simulink model "COMPONENT_MDL_Lag_QUAD_and_PEND_with_spin_rotors"  (R2021b)
(part 4 of 10)

    et228 = Lz_pend.^2.*THE_Theta_D.*m_pend.*cos(THE_Psi).^2.*cos(THE_Phi_pend).^2.*cos(THE_Psi_pend).*sin(THE_Psi_pend).*(2.0./3.0)+Lz_pend.^2.*THE_Theta_D.*m_pend.*cos(THE_Psi).^2.*cos(THE_Psi_pend).*cos(THE_Theta_pend).^2.*sin(THE_Psi_pend).*(2.0./3.0)+(Ly_pend.^2.*THE_Theta_D.*m_pend.*cos(THE_Psi).*cos(THE_Phi_pend).*cos(THE_Theta_pend).*sin(THE_Psi))./1.2e+1-(Ly_pend.^2.*THE_Theta_pend_D.*m_pend.*cos(THE_Psi).*cos(THE_Phi_pend).*cos(THE_Psi_pend).*sin(THE_Psi_pend))./6.0-(Lz_pend.^2.*THE_Theta_D.*m_pend.*cos(THE_Psi).*cos(THE_Phi_pend).*cos(THE_Theta_pend).*sin(THE_Psi))./3.0+Lz_pend.^2.*THE_Theta_pend_D.*m_pend.*cos(THE_Psi).*cos(THE_Phi_pend).*cos(THE_Psi_pend).*sin(THE_Psi_pend).*(2.0./3.0)+(Ly_pend.^2.*THE_Theta_D.*m_pend.*cos(THE_Psi).^2.*cos(THE_Phi_pend).*cos(THE_Psi_pend).^2.*sin(THE_Phi_pend).*sin(THE_Theta_pend))./6.0-Lz_pend.^2.*THE_Theta_D.*m_pend.*cos(THE_Psi).^2.*cos(THE_Phi_pend).*cos(THE_Psi_pend).^2.*sin(THE_Phi_pend).*sin(THE_Theta_pend).*(2.0./3.0)+(Ly_pend.^2.*THE_Psi_D.*m_pend.*cos(THE_Psi).*cos(THE_Phi_pend).*cos(THE_Psi_pend).*sin(THE_Phi_pend).*sin(THE_Psi_pend))./3.0-Lz_pend.^2.*THE_Psi_D.*m_pend.*cos(THE_Psi).*cos(THE_Phi_pend).*cos(THE_Psi_pend).*sin(THE_Phi_pend).*sin(THE_Psi_pend).*(4.0./3.0);
    et229 = (Ly_pend.^2.*THE_Theta_D.*m_pend.*cos(THE_Psi).^2.*cos(THE_Phi_pend).^2.*cos(THE_Psi_pend).*cos(THE_Theta_pend).^2.*sin(THE_Psi_pend))./1.2e+1-(Lz_pend.^2.*THE_Theta_D.*m_pend.*cos(THE_Psi).^2.*cos(THE_Phi_pend).^2.*cos(THE_Psi_pend).*cos(THE_Theta_pend).^2.*sin(THE_Psi_pend))./3.0+(Lz_pend.*THE_Theta_D.*Tv_Z_pend.*m_pend.*cos(THE_Psi).*cos(THE_Phi_pend).*cos(THE_Psi_pend).*sin(THE_Psi))./2.0+Lz_pend.*THE_Psi_D.*Tv_Z_pend.*m_pend.*cos(THE_Phi_pend).*sin(THE_Psi).*sin(THE_Psi_pend).*sin(THE_Theta_pend)-(Ly_pend.^2.*THE_Theta_D.*m_pend.*cos(THE_Psi).*cos(THE_Phi_pend).*cos(THE_Psi_pend).^2.*cos(THE_Theta_pend).*sin(THE_Psi))./6.0+Lz_pend.^2.*THE_Theta_D.*m_pend.*cos(THE_Psi).*cos(THE_Phi_pend).*cos(THE_Psi_pend).^2.*cos(THE_Theta_pend).*sin(THE_Psi).*(2.0./3.0)-(Ly_pend.^2.*THE_Psi_D.*m_pend.*cos(THE_Phi_pend).*cos(THE_Psi_pend).*cos(THE_Theta_pend).*sin(THE_Psi).*sin(THE_Psi_pend).*sin(THE_Theta_pend))./6.0+(Ly_pend.^2.*THE_Phi_pend_D.*m_pend.*cos(THE_Psi).*cos(THE_Psi_pend).*cos(THE_Theta_pend).*sin(THE_Phi_pend).*sin(THE_Psi_pend).*sin(THE_Theta_pend))./6.0+Lz_pend.^2.*THE_Psi_D.*m_pend.*cos(THE_Phi_pend).*cos(THE_Psi_pend).*cos(THE_Theta_pend).*sin(THE_Psi).*sin(THE_Psi_pend).*sin(THE_Theta_pend).*(2.0./3.0);
    et230 = Lz_pend.^2.*THE_Phi_pend_D.*m_pend.*cos(THE_Psi).*cos(THE_Psi_pend).*cos(THE_Theta_pend).*sin(THE_Phi_pend).*sin(THE_Psi_pend).*sin(THE_Theta_pend).*(-2.0./3.0)+(Lz_pend.*THE_Theta_D.*Tv_Z_pend.*m_pend.*cos(THE_Psi).*sin(THE_Psi).*sin(THE_Phi_pend).*sin(THE_Psi_pend).*sin(THE_Theta_pend))./2.0-(Ly_pend.^2.*THE_Psi_D.*m_pend.*cos(THE_Psi).*cos(THE_Phi_pend).*cos(THE_Psi_pend).*cos(THE_Theta_pend).^2.*sin(THE_Phi_pend).*sin(THE_Psi_pend))./6.0+Lz_pend.^2.*THE_Psi_D.*m_pend.*cos(THE_Psi).*cos(THE_Phi_pend).*cos(THE_Psi_pend).*cos(THE_Theta_pend).^2.*sin(THE_Phi_pend).*sin(THE_Psi_pend).*(2.0./3.0)-(Ly_pend.^2.*THE_Theta_D.*m_pend.*cos(THE_Psi).*cos(THE_Psi_pend).*cos(THE_Theta_pend).*sin(THE_Psi).*sin(THE_Phi_pend).*sin(THE_Psi_pend).*sin(THE_Theta_pend))./6.0+Lz_pend.^2.*THE_Theta_D.*m_pend.*cos(THE_Psi).*cos(THE_Psi_pend).*cos(THE_Theta_pend).*sin(THE_Psi).*sin(THE_Phi_pend).*sin(THE_Psi_pend).*sin(THE_Theta_pend).*(2.0./3.0);
    et231 = (Lx_pend.^2.*THE_Theta_D.*m_pend.*sin(THE_Theta_pend.*2.0))./2.4e+1-(Ly_pend.^2.*THE_Theta_D.*m_pend.*sin(THE_Theta_pend.*2.0))./2.4e+1-(Lx_pend.^2.*THE_Psi_D.*m_pend.*cos(THE_Phi_pend).*sin(THE_Psi))./6.0-(Ly_pend.^2.*THE_Phi_pend_D.*m_pend.*cos(THE_Psi).*sin(THE_Phi_pend))./6.0-(Ly_pend.^2.*THE_Psi_pend_D.*m_pend.*cos(THE_Theta_pend).*sin(THE_Psi))./6.0-(Lx_pend.^2.*THE_Theta_D.*m_pend.*cos(THE_Psi).*sin(THE_Psi).*sin(THE_Phi_pend))./1.2e+1-(Lx_pend.^2.*THE_Phi_pend_D.*m_pend.*cos(THE_Theta_pend).*sin(THE_Psi).*sin(THE_Theta_pend))./6.0+(Ly_pend.^2.*THE_Theta_D.*m_pend.*cos(THE_Psi).*sin(THE_Psi).*sin(THE_Phi_pend))./1.2e+1+(Ly_pend.^2.*THE_Psi_pend_D.*m_pend.*cos(THE_Psi).*sin(THE_Phi_pend).*sin(THE_Theta_pend))./6.0+(Ly_pend.^2.*THE_Phi_pend_D.*m_pend.*cos(THE_Theta_pend).*sin(THE_Psi).*sin(THE_Theta_pend))./6.0+(Lx_pend.^2.*THE_Psi_D.*m_pend.*cos(THE_Phi_pend).*cos(THE_Theta_pend).^2.*sin(THE_Psi))./6.0-(Lx_pend.^2.*THE_Theta_D.*m_pend.*cos(THE_Psi).^2.*cos(THE_Theta_pend).*sin(THE_Theta_pend))./6.0;
    et232 = Lx_pend.^2.*THE_Phi_pend_D.*m_pend.*cos(THE_Psi).*cos(THE_Theta_pend).^2.*sin(THE_Phi_pend).*(-1.0./6.0)-(Ly_pend.^2.*THE_Psi_D.*m_pend.*cos(THE_Phi_pend).*cos(THE_Theta_pend).^2.*sin(THE_Psi))./6.0+(Ly_pend.^2.*THE_Phi_pend_D.*m_pend.*cos(THE_Psi).*cos(THE_Psi_pend).^2.*sin(THE_Phi_pend))./6.0+(Ly_pend.^2.*THE_Theta_D.*m_pend.*cos(THE_Psi).^2.*cos(THE_Theta_pend).*sin(THE_Theta_pend))./6.0+(Ly_pend.^2.*THE_Phi_pend_D.*m_pend.*cos(THE_Psi).*cos(THE_Theta_pend).^2.*sin(THE_Phi_pend))./6.0+(Ly_pend.^2.*THE_Psi_pend_D.*m_pend.*cos(THE_Psi_pend).^2.*cos(THE_Theta_pend).*sin(THE_Psi))./6.0+(Ly_pend.^2.*THE_Theta_D.*m_pend.*cos(THE_Psi_pend).^2.*cos(THE_Theta_pend).*sin(THE_Theta_pend))./1.2e+1-Lz_pend.^2.*THE_Phi_pend_D.*m_pend.*cos(THE_Psi).*cos(THE_Psi_pend).^2.*sin(THE_Phi_pend).*(2.0./3.0)-Lz_pend.^2.*THE_Psi_pend_D.*m_pend.*cos(THE_Psi_pend).^2.*cos(THE_Theta_pend).*sin(THE_Psi).*(2.0./3.0)-(Lz_pend.^2.*THE_Theta_D.*m_pend.*cos(THE_Psi_pend).^2.*cos(THE_Theta_pend).*sin(THE_Theta_pend))./3.0+(Lx_pend.^2.*THE_Theta_D.*m_pend.*cos(THE_Psi).*cos(THE_Theta_pend).^2.*sin(THE_Psi).*sin(THE_Phi_pend))./6.0;
    et233 = Ly_pend.^2.*THE_Theta_D.*m_pend.*cos(THE_Psi).*cos(THE_Psi_pend).^2.*sin(THE_Psi).*sin(THE_Phi_pend).*(-1.0./1.2e+1)-(Ly_pend.^2.*THE_Theta_D.*m_pend.*cos(THE_Psi).*cos(THE_Theta_pend).^2.*sin(THE_Psi).*sin(THE_Phi_pend))./6.0-(Ly_pend.^2.*THE_Psi_pend_D.*m_pend.*cos(THE_Psi).*cos(THE_Psi_pend).^2.*sin(THE_Phi_pend).*sin(THE_Theta_pend))./6.0-(Ly_pend.^2.*THE_Phi_pend_D.*m_pend.*cos(THE_Psi_pend).^2.*cos(THE_Theta_pend).*sin(THE_Psi).*sin(THE_Theta_pend))./6.0+(Lz_pend.^2.*THE_Theta_D.*m_pend.*cos(THE_Psi).*cos(THE_Psi_pend).^2.*sin(THE_Psi).*sin(THE_Phi_pend))./3.0+Lz_pend.^2.*THE_Psi_pend_D.*m_pend.*cos(THE_Psi).*cos(THE_Psi_pend).^2.*sin(THE_Phi_pend).*sin(THE_Theta_pend).*(2.0./3.0)+Lz_pend.^2.*THE_Phi_pend_D.*m_pend.*cos(THE_Psi_pend).^2.*cos(THE_Theta_pend).*sin(THE_Psi).*sin(THE_Theta_pend).*(2.0./3.0)+(Lz_pend.*THE_Theta_D.*Tv_Z_pend.*m_pend.*cos(THE_Psi).^2.*cos(THE_Psi_pend).*sin(THE_Theta_pend))./2.0+(Lx_pend.^2.*THE_Theta_D.*m_pend.*cos(THE_Psi).^2.*cos(THE_Phi_pend).^2.*cos(THE_Theta_pend).*sin(THE_Theta_pend))./1.2e+1+(Ly_pend.^2.*THE_Psi_D.*m_pend.*cos(THE_Phi_pend).*cos(THE_Psi_pend).^2.*cos(THE_Theta_pend).^2.*sin(THE_Psi))./6.0;
    et234 = Ly_pend.^2.*THE_Theta_D.*m_pend.*cos(THE_Psi).^2.*cos(THE_Phi_pend).^2.*cos(THE_Theta_pend).*sin(THE_Theta_pend).*(-1.0./1.2e+1)-(Ly_pend.^2.*THE_Theta_D.*m_pend.*cos(THE_Psi).^2.*cos(THE_Psi_pend).^2.*cos(THE_Theta_pend).*sin(THE_Theta_pend))./6.0-(Ly_pend.^2.*THE_Phi_pend_D.*m_pend.*cos(THE_Psi).*cos(THE_Psi_pend).^2.*cos(THE_Theta_pend).^2.*sin(THE_Phi_pend))./6.0-Lz_pend.^2.*THE_Psi_D.*m_pend.*cos(THE_Phi_pend).*cos(THE_Psi_pend).^2.*cos(THE_Theta_pend).^2.*sin(THE_Psi).*(2.0./3.0)+Lz_pend.^2.*THE_Theta_D.*m_pend.*cos(THE_Psi).^2.*cos(THE_Psi_pend).^2.*cos(THE_Theta_pend).*sin(THE_Theta_pend).*(2.0./3.0)+Lz_pend.^2.*THE_Phi_pend_D.*m_pend.*cos(THE_Psi).*cos(THE_Psi_pend).^2.*cos(THE_Theta_pend).^2.*sin(THE_Phi_pend).*(2.0./3.0)+(Ly_pend.^2.*THE_Psi_pend_D.*m_pend.*cos(THE_Psi).*cos(THE_Phi_pend).*cos(THE_Psi_pend).*sin(THE_Psi_pend))./6.0-Lz_pend.^2.*THE_Psi_pend_D.*m_pend.*cos(THE_Psi).*cos(THE_Phi_pend).*cos(THE_Psi_pend).*sin(THE_Psi_pend).*(2.0./3.0)+(Ly_pend.^2.*THE_Theta_D.*m_pend.*cos(THE_Psi).*cos(THE_Psi_pend).^2.*cos(THE_Theta_pend).^2.*sin(THE_Psi).*sin(THE_Phi_pend))./6.0;
    et235 = Lz_pend.^2.*THE_Theta_D.*m_pend.*cos(THE_Psi).*cos(THE_Psi_pend).^2.*cos(THE_Theta_pend).^2.*sin(THE_Psi).*sin(THE_Phi_pend).*(-2.0./3.0)-(Lx_pend.^2.*THE_Psi_D.*m_pend.*cos(THE_Psi).*cos(THE_Phi_pend).*cos(THE_Theta_pend).*sin(THE_Phi_pend).*sin(THE_Theta_pend))./6.0+(Ly_pend.^2.*THE_Psi_D.*m_pend.*cos(THE_Psi).*cos(THE_Phi_pend).*cos(THE_Theta_pend).*sin(THE_Phi_pend).*sin(THE_Theta_pend))./6.0-(Ly_pend.^2.*THE_Phi_pend_D.*m_pend.*cos(THE_Psi).*cos(THE_Phi_pend).*cos(THE_Psi_pend).*sin(THE_Psi_pend).*sin(THE_Theta_pend))./6.0+Lz_pend.^2.*THE_Phi_pend_D.*m_pend.*cos(THE_Psi).*cos(THE_Phi_pend).*cos(THE_Psi_pend).*sin(THE_Psi_pend).*sin(THE_Theta_pend).*(2.0./3.0)+(Ly_pend.^2.*THE_Theta_D.*m_pend.*cos(THE_Psi).^2.*cos(THE_Phi_pend).^2.*cos(THE_Psi_pend).^2.*cos(THE_Theta_pend).*sin(THE_Theta_pend))./1.2e+1-(Lz_pend.^2.*THE_Theta_D.*m_pend.*cos(THE_Psi).^2.*cos(THE_Phi_pend).^2.*cos(THE_Psi_pend).^2.*cos(THE_Theta_pend).*sin(THE_Theta_pend))./3.0-Lz_pend.*THE_Psi_D.*Tv_Z_pend.*m_pend.*cos(THE_Phi_pend).*cos(THE_Psi_pend).*cos(THE_Theta_pend).*sin(THE_Psi)+(Ly_pend.^2.*THE_Psi_D.*m_pend.*cos(THE_Psi).*cos(THE_Phi_pend).^2.*cos(THE_Psi_pend).*cos(THE_Theta_pend).*sin(THE_Psi_pend))./6.0;
    et236 = Lz_pend.^2.*THE_Psi_D.*m_pend.*cos(THE_Psi).*cos(THE_Phi_pend).^2.*cos(THE_Psi_pend).*cos(THE_Theta_pend).*sin(THE_Psi_pend).*(-2.0./3.0)+(Ly_pend.^2.*THE_Theta_D.*m_pend.*cos(THE_Psi).*cos(THE_Phi_pend).*cos(THE_Psi_pend).*sin(THE_Psi).*sin(THE_Psi_pend).*sin(THE_Theta_pend))./1.2e+1-(Lz_pend.^2.*THE_Theta_D.*m_pend.*cos(THE_Psi).*cos(THE_Phi_pend).*cos(THE_Psi_pend).*sin(THE_Psi).*sin(THE_Psi_pend).*sin(THE_Theta_pend))./3.0-(Lz_pend.*THE_Theta_D.*Tv_Z_pend.*m_pend.*cos(THE_Psi).*cos(THE_Psi_pend).*cos(THE_Theta_pend).*sin(THE_Psi).*sin(THE_Phi_pend))./2.0-(Ly_pend.^2.*THE_Psi_D.*m_pend.*cos(THE_Psi).*cos(THE_Phi_pend).*cos(THE_Psi_pend).^2.*cos(THE_Theta_pend).*sin(THE_Phi_pend).*sin(THE_Theta_pend))./6.0+(Ly_pend.^2.*THE_Theta_D.*m_pend.*cos(THE_Psi).^2.*cos(THE_Phi_pend).*cos(THE_Psi_pend).*cos(THE_Theta_pend).*sin(THE_Phi_pend).*sin(THE_Psi_pend))./1.2e+1+Lz_pend.^2.*THE_Psi_D.*m_pend.*cos(THE_Psi).*cos(THE_Phi_pend).*cos(THE_Psi_pend).^2.*cos(THE_Theta_pend).*sin(THE_Phi_pend).*sin(THE_Theta_pend).*(2.0./3.0)-(Lz_pend.^2.*THE_Theta_D.*m_pend.*cos(THE_Psi).^2.*cos(THE_Phi_pend).*cos(THE_Psi_pend).*cos(THE_Theta_pend).*sin(THE_Phi_pend).*sin(THE_Psi_pend))./3.0;
    et237 = Ly_pend.^2.*THE_Psi_D.*m_pend.*cos(THE_Psi).*(-1.0./6.0)+(Ly_pend.^2.*THE_Theta_pend_D.*m_pend.*cos(THE_Psi).*sin(THE_Phi_pend))./6.0-(Lx_pend.^2.*THE_Psi_D.*m_pend.*cos(THE_Psi).*cos(THE_Theta_pend).^2)./6.0+(Ly_pend.^2.*THE_Psi_D.*m_pend.*cos(THE_Psi).*cos(THE_Phi_pend).^2)./6.0+(Ly_pend.^2.*THE_Psi_D.*m_pend.*cos(THE_Psi).*cos(THE_Psi_pend).^2)./6.0+(Ly_pend.^2.*THE_Psi_D.*m_pend.*cos(THE_Psi).*cos(THE_Theta_pend).^2)./6.0-Lz_pend.^2.*THE_Psi_D.*m_pend.*cos(THE_Psi).*cos(THE_Phi_pend).^2.*(2.0./3.0)-Lz_pend.^2.*THE_Psi_D.*m_pend.*cos(THE_Psi).*cos(THE_Psi_pend).^2.*(2.0./3.0)+(Lx_pend.^2.*THE_Theta_pend_D.*m_pend.*cos(THE_Theta_pend).*sin(THE_Psi).*sin(THE_Theta_pend))./6.0-(Ly_pend.^2.*THE_Theta_pend_D.*m_pend.*cos(THE_Theta_pend).*sin(THE_Psi).*sin(THE_Theta_pend))./6.0+(Lx_pend.^2.*THE_Theta_pend_D.*m_pend.*cos(THE_Psi).*cos(THE_Theta_pend).^2.*sin(THE_Phi_pend))./6.0+(Ly_pend.^2.*THE_Theta_D.*m_pend.*cos(THE_Psi).^2.*cos(THE_Phi_pend).*sin(THE_Phi_pend))./1.2e+1;
    et238 = Ly_pend.^2.*THE_Theta_pend_D.*m_pend.*cos(THE_Psi).*cos(THE_Psi_pend).^2.*sin(THE_Phi_pend).*(-1.0./6.0)-(Ly_pend.^2.*THE_Theta_pend_D.*m_pend.*cos(THE_Psi).*cos(THE_Theta_pend).^2.*sin(THE_Phi_pend))./6.0-(Lz_pend.^2.*THE_Theta_D.*m_pend.*cos(THE_Psi).^2.*cos(THE_Phi_pend).*sin(THE_Phi_pend))./3.0+Lz_pend.^2.*THE_Theta_pend_D.*m_pend.*cos(THE_Psi).*cos(THE_Psi_pend).^2.*sin(THE_Phi_pend).*(2.0./3.0)+(Lx_pend.^2.*THE_Psi_D.*m_pend.*cos(THE_Psi).*cos(THE_Phi_pend).^2.*cos(THE_Theta_pend).^2)./6.0-(Ly_pend.^2.*THE_Psi_D.*m_pend.*cos(THE_Psi).*cos(THE_Phi_pend).^2.*cos(THE_Psi_pend).^2)./3.0-(Ly_pend.^2.*THE_Psi_D.*m_pend.*cos(THE_Psi).*cos(THE_Phi_pend).^2.*cos(THE_Theta_pend).^2)./6.0-(Ly_pend.^2.*THE_Psi_D.*m_pend.*cos(THE_Psi).*cos(THE_Psi_pend).^2.*cos(THE_Theta_pend).^2)./6.0+Lz_pend.^2.*THE_Psi_D.*m_pend.*cos(THE_Psi).*cos(THE_Phi_pend).^2.*cos(THE_Psi_pend).^2.*(4.0./3.0)+Lz_pend.^2.*THE_Psi_D.*m_pend.*cos(THE_Psi).*cos(THE_Psi_pend).^2.*cos(THE_Theta_pend).^2.*(2.0./3.0);
    et239 = Lz_pend.^2.*THE_Psi_pend_D.*m_pend.*cos(THE_Psi).*cos(THE_Phi_pend).*cos(THE_Theta_pend).*(-2.0./3.0)-Lz_pend.*THE_Psi_D.*Tv_Z_pend.*m_pend.*cos(THE_Phi_pend).*sin(THE_Psi).*sin(THE_Psi_pend)-(Ly_pend.^2.*THE_Psi_pend_D.*m_pend.*cos(THE_Psi).*cos(THE_Phi_pend).*cos(THE_Psi_pend).^2.*cos(THE_Theta_pend))./6.0+Lz_pend.^2.*THE_Psi_pend_D.*m_pend.*cos(THE_Psi).*cos(THE_Phi_pend).*cos(THE_Psi_pend).^2.*cos(THE_Theta_pend).*(2.0./3.0)-(Ly_pend.^2.*THE_Theta_D.*m_pend.*cos(THE_Psi).^2.*cos(THE_Psi_pend).*sin(THE_Psi_pend).*sin(THE_Theta_pend))./1.2e+1+(Ly_pend.^2.*THE_Psi_pend_D.*m_pend.*cos(THE_Psi_pend).*cos(THE_Theta_pend).^2.*sin(THE_Psi).*sin(THE_Psi_pend))./6.0+(Ly_pend.^2.*THE_Theta_pend_D.*m_pend.*cos(THE_Psi_pend).^2.*cos(THE_Theta_pend).*sin(THE_Psi).*sin(THE_Theta_pend))./6.0+(Lz_pend.^2.*THE_Theta_D.*m_pend.*cos(THE_Psi).^2.*cos(THE_Psi_pend).*sin(THE_Psi_pend).*sin(THE_Theta_pend))./3.0-Lz_pend.^2.*THE_Psi_pend_D.*m_pend.*cos(THE_Psi_pend).*cos(THE_Theta_pend).^2.*sin(THE_Psi).*sin(THE_Psi_pend).*(2.0./3.0)-Lz_pend.^2.*THE_Theta_pend_D.*m_pend.*cos(THE_Psi_pend).^2.*cos(THE_Theta_pend).*sin(THE_Psi).*sin(THE_Theta_pend).*(2.0./3.0);
    et240 = (Lx_pend.^2.*THE_Theta_D.*m_pend.*cos(THE_Psi).^2.*cos(THE_Phi_pend).*cos(THE_Theta_pend).^2.*sin(THE_Phi_pend))./1.2e+1-(Ly_pend.^2.*THE_Theta_D.*m_pend.*cos(THE_Psi).^2.*cos(THE_Phi_pend).*cos(THE_Psi_pend).^2.*sin(THE_Phi_pend))./6.0-(Ly_pend.^2.*THE_Theta_D.*m_pend.*cos(THE_Psi).^2.*cos(THE_Phi_pend).*cos(THE_Theta_pend).^2.*sin(THE_Phi_pend))./1.2e+1+(Ly_pend.^2.*THE_Theta_pend_D.*m_pend.*cos(THE_Psi).*cos(THE_Psi_pend).^2.*cos(THE_Theta_pend).^2.*sin(THE_Phi_pend))./6.0+Lz_pend.^2.*THE_Theta_D.*m_pend.*cos(THE_Psi).^2.*cos(THE_Phi_pend).*cos(THE_Psi_pend).^2.*sin(THE_Phi_pend).*(2.0./3.0)-Lz_pend.^2.*THE_Theta_pend_D.*m_pend.*cos(THE_Psi).*cos(THE_Psi_pend).^2.*cos(THE_Theta_pend).^2.*sin(THE_Phi_pend).*(2.0./3.0)+(Ly_pend.^2.*THE_Psi_D.*m_pend.*cos(THE_Psi).*cos(THE_Phi_pend).^2.*cos(THE_Psi_pend).^2.*cos(THE_Theta_pend).^2)./6.0-Lz_pend.^2.*THE_Psi_D.*m_pend.*cos(THE_Psi).*cos(THE_Phi_pend).^2.*cos(THE_Psi_pend).^2.*cos(THE_Theta_pend).^2.*(2.0./3.0)-(Lx_pend.^2.*THE_Psi_D.*m_pend.*cos(THE_Theta_pend).*sin(THE_Psi).*sin(THE_Phi_pend).*sin(THE_Theta_pend))./6.0;
    et241 = (Ly_pend.^2.*THE_Psi_D.*m_pend.*cos(THE_Theta_pend).*sin(THE_Psi).*sin(THE_Phi_pend).*sin(THE_Theta_pend))./6.0+(Ly_pend.^2.*THE_Theta_D.*m_pend.*cos(THE_Psi).^2.*cos(THE_Phi_pend).^2.*cos(THE_Psi_pend).*sin(THE_Psi_pend).*sin(THE_Theta_pend))./6.0-Lz_pend.^2.*THE_Theta_D.*m_pend.*cos(THE_Psi).^2.*cos(THE_Phi_pend).^2.*cos(THE_Psi_pend).*sin(THE_Psi_pend).*sin(THE_Theta_pend).*(2.0./3.0)+(Lx_pend.^2.*THE_Theta_D.*m_pend.*cos(THE_Psi).*cos(THE_Phi_pend).*cos(THE_Theta_pend).*sin(THE_Psi).*sin(THE_Theta_pend))./1.2e+1-(Ly_pend.^2.*THE_Theta_D.*m_pend.*cos(THE_Psi).*cos(THE_Phi_pend).*cos(THE_Theta_pend).*sin(THE_Psi).*sin(THE_Theta_pend))./1.2e+1+(Ly_pend.^2.*THE_Psi_D.*m_pend.*cos(THE_Phi_pend).*cos(THE_Psi_pend).*cos(THE_Theta_pend).*sin(THE_Psi).*sin(THE_Psi_pend))./6.0+(Ly_pend.^2.*THE_Theta_pend_D.*m_pend.*cos(THE_Psi).*cos(THE_Phi_pend).*cos(THE_Psi_pend).*sin(THE_Psi_pend).*sin(THE_Theta_pend))./6.0-Lz_pend.^2.*THE_Psi_D.*m_pend.*cos(THE_Phi_pend).*cos(THE_Psi_pend).*cos(THE_Theta_pend).*sin(THE_Psi).*sin(THE_Psi_pend).*(2.0./3.0)-Lz_pend.^2.*THE_Theta_pend_D.*m_pend.*cos(THE_Psi).*cos(THE_Phi_pend).*cos(THE_Psi_pend).*sin(THE_Psi_pend).*sin(THE_Theta_pend).*(2.0./3.0);
    et242 = (Ly_pend.^2.*THE_Theta_D.*m_pend.*cos(THE_Psi).^2.*cos(THE_Phi_pend).*cos(THE_Psi_pend).^2.*cos(THE_Theta_pend).^2.*sin(THE_Phi_pend))./1.2e+1-(Lz_pend.^2.*THE_Theta_D.*m_pend.*cos(THE_Psi).^2.*cos(THE_Phi_pend).*cos(THE_Psi_pend).^2.*cos(THE_Theta_pend).^2.*sin(THE_Phi_pend))./3.0-(Lz_pend.*THE_Theta_D.*Tv_Z_pend.*m_pend.*cos(THE_Psi).*sin(THE_Psi).*sin(THE_Phi_pend).*sin(THE_Psi_pend))./2.0+Lz_pend.*THE_Psi_D.*Tv_Z_pend.*m_pend.*cos(THE_Psi_pend).*sin(THE_Psi).*sin(THE_Phi_pend).*sin(THE_Theta_pend)-(Ly_pend.^2.*THE_Psi_D.*m_pend.*cos(THE_Psi_pend).^2.*cos(THE_Theta_pend).*sin(THE_Psi).*sin(THE_Phi_pend).*sin(THE_Theta_pend))./6.0+Lz_pend.^2.*THE_Psi_D.*m_pend.*cos(THE_Psi_pend).^2.*cos(THE_Theta_pend).*sin(THE_Psi).*sin(THE_Phi_pend).*sin(THE_Theta_pend).*(2.0./3.0)+(Ly_pend.^2.*THE_Theta_D.*m_pend.*cos(THE_Psi).*cos(THE_Psi_pend).*cos(THE_Theta_pend).*sin(THE_Psi).*sin(THE_Phi_pend).*sin(THE_Psi_pend))./1.2e+1-(Ly_pend.^2.*THE_Psi_D.*m_pend.*cos(THE_Psi).*cos(THE_Phi_pend).*cos(THE_Psi_pend).*sin(THE_Phi_pend).*sin(THE_Psi_pend).*sin(THE_Theta_pend))./3.0-(Ly_pend.^2.*THE_Psi_pend_D.*m_pend.*cos(THE_Psi).*cos(THE_Psi_pend).*cos(THE_Theta_pend).*sin(THE_Phi_pend).*sin(THE_Psi_pend).*sin(THE_Theta_pend))./6.0;
    et243 = Lz_pend.^2.*THE_Theta_D.*m_pend.*cos(THE_Psi).*cos(THE_Psi_pend).*cos(THE_Theta_pend).*sin(THE_Psi).*sin(THE_Phi_pend).*sin(THE_Psi_pend).*(-1.0./3.0)+Lz_pend.^2.*THE_Psi_D.*m_pend.*cos(THE_Psi).*cos(THE_Phi_pend).*cos(THE_Psi_pend).*sin(THE_Phi_pend).*sin(THE_Psi_pend).*sin(THE_Theta_pend).*(4.0./3.0)+Lz_pend.^2.*THE_Psi_pend_D.*m_pend.*cos(THE_Psi).*cos(THE_Psi_pend).*cos(THE_Theta_pend).*sin(THE_Phi_pend).*sin(THE_Psi_pend).*sin(THE_Theta_pend).*(2.0./3.0)-(Lz_pend.*THE_Theta_D.*Tv_Z_pend.*m_pend.*cos(THE_Psi).*cos(THE_Phi_pend).*cos(THE_Psi_pend).*sin(THE_Psi).*sin(THE_Theta_pend))./2.0+(Ly_pend.^2.*THE_Theta_D.*m_pend.*cos(THE_Psi).*cos(THE_Phi_pend).*cos(THE_Psi_pend).^2.*cos(THE_Theta_pend).*sin(THE_Psi).*sin(THE_Theta_pend))./1.2e+1-(Lz_pend.^2.*THE_Theta_D.*m_pend.*cos(THE_Psi).*cos(THE_Phi_pend).*cos(THE_Psi_pend).^2.*cos(THE_Theta_pend).*sin(THE_Psi).*sin(THE_Theta_pend))./3.0;
    et244 = THE_Psi_D.*Tv_Z_pend.*m_pend.*sin(THE_Psi).*sin(THE_Theta).*2.0+THE_Psi_D.*cg_to_mot_H.*mprop.*sin(THE_Psi).*sin(THE_Theta).*8.0-THE_Theta_D.*Tv_Z_pend.*m_pend.*cos(THE_Psi).*cos(THE_Theta)-THE_Theta_D.*cg_to_mot_H.*mprop.*cos(THE_Psi).*cos(THE_Theta).*4.0-Lz_pend.*THE_Phi_pend_D.*m_pend.*cos(THE_Theta).*cos(THE_Phi_pend).*sin(THE_Psi_pend)-Lz_pend.*THE_Psi_pend_D.*m_pend.*cos(THE_Theta).*cos(THE_Psi_pend).*sin(THE_Phi_pend)+(Lz_pend.*THE_Theta_D.*m_pend.*sin(THE_Theta).*sin(THE_Phi_pend).*sin(THE_Psi_pend))./2.0-(Lz_pend.*THE_Theta_D.*m_pend.*cos(THE_Psi).*cos(THE_Theta).*cos(THE_Psi_pend).*cos(THE_Theta_pend))./2.0-Lz_pend.*THE_Theta_pend_D.*m_pend.*cos(THE_Theta).*cos(THE_Phi_pend).*cos(THE_Psi_pend).*cos(THE_Theta_pend)+Lz_pend.*THE_Psi_D.*m_pend.*cos(THE_Psi).*cos(THE_Phi_pend).*sin(THE_Theta).*sin(THE_Psi_pend)+(Lz_pend.*THE_Theta_D.*m_pend.*cos(THE_Theta).*cos(THE_Phi_pend).*sin(THE_Psi).*sin(THE_Psi_pend))./2.0+Lz_pend.*THE_Psi_D.*m_pend.*cos(THE_Psi_pend).*cos(THE_Theta_pend).*sin(THE_Psi).*sin(THE_Theta)+Lz_pend.*THE_Psi_pend_D.*m_pend.*cos(THE_Phi_pend).*cos(THE_Psi_pend).*sin(THE_Psi).*sin(THE_Theta)+Lz_pend.*THE_Psi_pend_D.*m_pend.*cos(THE_Psi).*cos(THE_Theta_pend).*sin(THE_Theta).*sin(THE_Psi_pend)+(Lz_pend.*THE_Theta_D.*m_pend.*cos(THE_Phi_pend).*cos(THE_Psi_pend).*sin(THE_Theta).*sin(THE_Theta_pend))./2.0+Lz_pend.*THE_Theta_pend_D.*m_pend.*cos(THE_Psi).*cos(THE_Psi_pend).*sin(THE_Theta).*sin(THE_Theta_pend);
    et245 = Lz_pend.*THE_Phi_pend_D.*m_pend.*cos(THE_Theta).*cos(THE_Psi_pend).*sin(THE_Phi_pend).*sin(THE_Theta_pend)+Lz_pend.*THE_Psi_pend_D.*m_pend.*cos(THE_Theta).*cos(THE_Phi_pend).*sin(THE_Psi_pend).*sin(THE_Theta_pend)-Lz_pend.*THE_Phi_pend_D.*m_pend.*sin(THE_Psi).*sin(THE_Theta).*sin(THE_Phi_pend).*sin(THE_Psi_pend)-Lz_pend.*THE_Psi_D.*m_pend.*cos(THE_Psi).*cos(THE_Psi_pend).*sin(THE_Theta).*sin(THE_Phi_pend).*sin(THE_Theta_pend)-(Lz_pend.*THE_Theta_D.*m_pend.*cos(THE_Theta).*cos(THE_Psi_pend).*sin(THE_Psi).*sin(THE_Phi_pend).*sin(THE_Theta_pend))./2.0-Lz_pend.*THE_Phi_pend_D.*m_pend.*cos(THE_Phi_pend).*cos(THE_Psi_pend).*sin(THE_Psi).*sin(THE_Theta).*sin(THE_Theta_pend)-Lz_pend.*THE_Theta_pend_D.*m_pend.*cos(THE_Psi_pend).*cos(THE_Theta_pend).*sin(THE_Psi).*sin(THE_Theta).*sin(THE_Phi_pend)+Lz_pend.*THE_Psi_pend_D.*m_pend.*sin(THE_Psi).*sin(THE_Theta).*sin(THE_Phi_pend).*sin(THE_Psi_pend).*sin(THE_Theta_pend);
    et246 = THE_Psi_D.*cg_to_mot_H.*mprop.*cos(THE_Theta).*sin(THE_Psi).*1.6e+1+THE_Theta_D.*cg_to_mot_H.*mprop.*cos(THE_Psi).*sin(THE_Theta).*8.0+THE_Psi_D.*Tv_Z_pend.*m_pend.*cos(THE_Theta).*sin(THE_Psi).*4.0+THE_Theta_D.*Tv_Z_pend.*m_pend.*cos(THE_Psi).*sin(THE_Theta).*2.0+Lz_pend.*THE_Theta_D.*m_pend.*cos(THE_Theta).*sin(THE_Phi_pend).*sin(THE_Psi_pend)+Lz_pend.*THE_Phi_pend_D.*m_pend.*cos(THE_Phi_pend).*sin(THE_Theta).*sin(THE_Psi_pend).*2.0+Lz_pend.*THE_Psi_pend_D.*m_pend.*cos(THE_Psi_pend).*sin(THE_Theta).*sin(THE_Phi_pend).*2.0+Lz_pend.*THE_Psi_D.*m_pend.*cos(THE_Psi).*cos(THE_Theta).*cos(THE_Phi_pend).*sin(THE_Psi_pend).*2.0+Lz_pend.*THE_Psi_D.*m_pend.*cos(THE_Theta).*cos(THE_Psi_pend).*cos(THE_Theta_pend).*sin(THE_Psi).*2.0+Lz_pend.*THE_Theta_D.*m_pend.*cos(THE_Psi).*cos(THE_Psi_pend).*cos(THE_Theta_pend).*sin(THE_Theta)+Lz_pend.*THE_Psi_pend_D.*m_pend.*cos(THE_Theta).*cos(THE_Phi_pend).*cos(THE_Psi_pend).*sin(THE_Psi).*2.0+Lz_pend.*THE_Psi_pend_D.*m_pend.*cos(THE_Psi).*cos(THE_Theta).*cos(THE_Theta_pend).*sin(THE_Psi_pend).*2.0+Lz_pend.*THE_Theta_D.*m_pend.*cos(THE_Theta).*cos(THE_Phi_pend).*cos(THE_Psi_pend).*sin(THE_Theta_pend)+Lz_pend.*THE_Theta_pend_D.*m_pend.*cos(THE_Psi).*cos(THE_Theta).*cos(THE_Psi_pend).*sin(THE_Theta_pend).*2.0+Lz_pend.*THE_Theta_pend_D.*m_pend.*cos(THE_Phi_pend).*cos(THE_Psi_pend).*cos(THE_Theta_pend).*sin(THE_Theta).*2.0-Lz_pend.*THE_Theta_D.*m_pend.*cos(THE_Phi_pend).*sin(THE_Psi).*sin(THE_Theta).*sin(THE_Psi_pend)-Lz_pend.*THE_Phi_pend_D.*m_pend.*cos(THE_Theta).*sin(THE_Psi).*sin(THE_Phi_pend).*sin(THE_Psi_pend).*2.0;
    et247 = Lz_pend.*THE_Phi_pend_D.*m_pend.*cos(THE_Psi_pend).*sin(THE_Theta).*sin(THE_Phi_pend).*sin(THE_Theta_pend).*-2.0-Lz_pend.*THE_Psi_pend_D.*m_pend.*cos(THE_Phi_pend).*sin(THE_Theta).*sin(THE_Psi_pend).*sin(THE_Theta_pend).*2.0-Lz_pend.*THE_Psi_D.*m_pend.*cos(THE_Psi).*cos(THE_Theta).*cos(THE_Psi_pend).*sin(THE_Phi_pend).*sin(THE_Theta_pend).*2.0-Lz_pend.*THE_Phi_pend_D.*m_pend.*cos(THE_Theta).*cos(THE_Phi_pend).*cos(THE_Psi_pend).*sin(THE_Psi).*sin(THE_Theta_pend).*2.0-Lz_pend.*THE_Theta_pend_D.*m_pend.*cos(THE_Theta).*cos(THE_Psi_pend).*cos(THE_Theta_pend).*sin(THE_Psi).*sin(THE_Phi_pend).*2.0+Lz_pend.*THE_Theta_D.*m_pend.*cos(THE_Psi_pend).*sin(THE_Psi).*sin(THE_Theta).*sin(THE_Phi_pend).*sin(THE_Theta_pend)+Lz_pend.*THE_Psi_pend_D.*m_pend.*cos(THE_Theta).*sin(THE_Psi).*sin(THE_Phi_pend).*sin(THE_Psi_pend).*sin(THE_Theta_pend).*2.0;
    et248 = THE_Psi_D.*cg_to_mot_H.*mprop.*cos(THE_Theta).*sin(THE_Psi).*1.6e+1+THE_Theta_D.*cg_to_mot_H.*mprop.*cos(THE_Psi).*sin(THE_Theta).*8.0+THE_Psi_D.*Tv_Z_pend.*m_pend.*cos(THE_Theta).*sin(THE_Psi).*4.0+THE_Theta_D.*Tv_Z_pend.*m_pend.*cos(THE_Psi).*sin(THE_Theta).*2.0+Lz_pend.*THE_Theta_D.*m_pend.*cos(THE_Theta).*sin(THE_Phi_pend).*sin(THE_Psi_pend)+Lz_pend.*THE_Phi_pend_D.*m_pend.*cos(THE_Phi_pend).*sin(THE_Theta).*sin(THE_Psi_pend).*2.0+Lz_pend.*THE_Psi_pend_D.*m_pend.*cos(THE_Psi_pend).*sin(THE_Theta).*sin(THE_Phi_pend).*2.0+Lz_pend.*THE_Psi_D.*m_pend.*cos(THE_Psi).*cos(THE_Theta).*cos(THE_Phi_pend).*sin(THE_Psi_pend).*2.0+Lz_pend.*THE_Psi_D.*m_pend.*cos(THE_Theta).*cos(THE_Psi_pend).*cos(THE_Theta_pend).*sin(THE_Psi).*2.0+Lz_pend.*THE_Theta_D.*m_pend.*cos(THE_Psi).*cos(THE_Psi_pend).*cos(THE_Theta_pend).*sin(THE_Theta)+Lz_pend.*THE_Psi_pend_D.*m_pend.*cos(THE_Theta).*cos(THE_Phi_pend).*cos(THE_Psi_pend).*sin(THE_Psi).*2.0+Lz_pend.*THE_Psi_pend_D.*m_pend.*cos(THE_Psi).*cos(THE_Theta).*cos(THE_Theta_pend).*sin(THE_Psi_pend).*2.0+Lz_pend.*THE_Theta_D.*m_pend.*cos(THE_Theta).*cos(THE_Phi_pend).*cos(THE_Psi_pend).*sin(THE_Theta_pend)+Lz_pend.*THE_Theta_pend_D.*m_pend.*cos(THE_Psi).*cos(THE_Theta).*cos(THE_Psi_pend).*sin(THE_Theta_pend).*2.0+Lz_pend.*THE_Theta_pend_D.*m_pend.*cos(THE_Phi_pend).*cos(THE_Psi_pend).*cos(THE_Theta_pend).*sin(THE_Theta).*2.0-Lz_pend.*THE_Theta_D.*m_pend.*cos(THE_Phi_pend).*sin(THE_Psi).*sin(THE_Theta).*sin(THE_Psi_pend)-Lz_pend.*THE_Phi_pend_D.*m_pend.*cos(THE_Theta).*sin(THE_Psi).*sin(THE_Phi_pend).*sin(THE_Psi_pend).*2.0;
    et249 = Lz_pend.*THE_Phi_pend_D.*m_pend.*cos(THE_Psi_pend).*sin(THE_Theta).*sin(THE_Phi_pend).*sin(THE_Theta_pend).*-2.0-Lz_pend.*THE_Psi_pend_D.*m_pend.*cos(THE_Phi_pend).*sin(THE_Theta).*sin(THE_Psi_pend).*sin(THE_Theta_pend).*2.0-Lz_pend.*THE_Psi_D.*m_pend.*cos(THE_Psi).*cos(THE_Theta).*cos(THE_Psi_pend).*sin(THE_Phi_pend).*sin(THE_Theta_pend).*2.0-Lz_pend.*THE_Phi_pend_D.*m_pend.*cos(THE_Theta).*cos(THE_Phi_pend).*cos(THE_Psi_pend).*sin(THE_Psi).*sin(THE_Theta_pend).*2.0-Lz_pend.*THE_Theta_pend_D.*m_pend.*cos(THE_Theta).*cos(THE_Psi_pend).*cos(THE_Theta_pend).*sin(THE_Psi).*sin(THE_Phi_pend).*2.0+Lz_pend.*THE_Theta_D.*m_pend.*cos(THE_Psi_pend).*sin(THE_Psi).*sin(THE_Theta).*sin(THE_Phi_pend).*sin(THE_Theta_pend)+Lz_pend.*THE_Psi_pend_D.*m_pend.*cos(THE_Theta).*sin(THE_Psi).*sin(THE_Phi_pend).*sin(THE_Psi_pend).*sin(THE_Theta_pend).*2.0;
    et250 = -I_yz.*THE_Theta_D-Iprop_yz.*THE_Theta_D.*4.0+I_yz.*THE_Theta_D.*cos(THE_Psi).^2.*2.0+Iprop_yz.*THE_Theta_D.*cos(THE_Psi).^2.*8.0+(I_yy.*THE_Theta_D.*sin(THE_Psi.*2.0))./2.0-(I_zz.*THE_Theta_D.*sin(THE_Psi.*2.0))./2.0+Iprop_yy.*THE_Theta_D.*sin(THE_Psi.*2.0).*2.0-Iprop_zz.*THE_Theta_D.*sin(THE_Psi.*2.0).*2.0+Iprop_zz.*wMOT_1.*cos(THE_Psi)+Iprop_zz.*wMOT_2.*cos(THE_Psi)+Iprop_zz.*wMOT_3.*cos(THE_Psi)+Iprop_zz.*wMOT_4.*cos(THE_Psi)+Iprop_yz.*wMOT_1.*sin(THE_Psi)+Iprop_yz.*wMOT_2.*sin(THE_Psi)+Iprop_yz.*wMOT_3.*sin(THE_Psi)+Iprop_yz.*wMOT_4.*sin(THE_Psi)+THE_Theta_D.*cg_to_mot_H.^2.*mprop.*sin(THE_Psi.*2.0).*2.0-THE_Theta_D.*cg_to_mot_L.^2.*mprop.*sin(THE_Psi.*2.0)+(Ly_pend.^2.*THE_Phi_pend_D.*m_pend.*cos(THE_Psi))./6.0+(Lx_pend.^2.*THE_Theta_D.*m_pend.*sin(THE_Psi.*2.0))./2.4e+1-(Ly_pend.^2.*THE_Theta_D.*m_pend.*sin(THE_Psi.*2.0))./2.4e+1+(THE_Theta_D.*Tv_Z_pend.^2.*m_pend.*sin(THE_Psi.*2.0))./2.0+(Lx_pend.^2.*THE_Theta_pend_D.*m_pend.*cos(THE_Phi_pend).*sin(THE_Psi))./6.0;
    et251 = Ly_pend.^2.*THE_Psi_pend_D.*m_pend.*cos(THE_Psi).*sin(THE_Theta_pend).*(-1.0./6.0)+(Lx_pend.^2.*THE_Phi_pend_D.*m_pend.*cos(THE_Psi).*cos(THE_Theta_pend).^2)./6.0-(Ly_pend.^2.*THE_Phi_pend_D.*m_pend.*cos(THE_Psi).*cos(THE_Phi_pend).^2)./6.0-(Ly_pend.^2.*THE_Phi_pend_D.*m_pend.*cos(THE_Psi).*cos(THE_Psi_pend).^2)./6.0-(Ly_pend.^2.*THE_Phi_pend_D.*m_pend.*cos(THE_Psi).*cos(THE_Theta_pend).^2)./6.0+Lz_pend.^2.*THE_Phi_pend_D.*m_pend.*cos(THE_Psi).*cos(THE_Phi_pend).^2.*(2.0./3.0)+Lz_pend.^2.*THE_Phi_pend_D.*m_pend.*cos(THE_Psi).*cos(THE_Psi_pend).^2.*(2.0./3.0)-(Lx_pend.^2.*THE_Theta_D.*m_pend.*cos(THE_Theta_pend).*sin(THE_Phi_pend).*sin(THE_Theta_pend))./1.2e+1+(Ly_pend.^2.*THE_Psi_pend_D.*m_pend.*cos(THE_Theta_pend).*sin(THE_Psi).*sin(THE_Phi_pend))./6.0+(Ly_pend.^2.*THE_Theta_D.*m_pend.*cos(THE_Theta_pend).*sin(THE_Phi_pend).*sin(THE_Theta_pend))./1.2e+1-(Lz_pend.*THE_Theta_D.*Tv_Z_pend.*m_pend.*cos(THE_Phi_pend).*sin(THE_Psi_pend))./2.0-(Lx_pend.^2.*THE_Theta_D.*m_pend.*cos(THE_Psi).*cos(THE_Theta_pend).^2.*sin(THE_Psi))./6.0;
    et252 = Lx_pend.^2.*THE_Theta_pend_D.*m_pend.*cos(THE_Phi_pend).*cos(THE_Theta_pend).^2.*sin(THE_Psi).*(-1.0./6.0)+(Ly_pend.^2.*THE_Theta_D.*m_pend.*cos(THE_Psi).*cos(THE_Phi_pend).^2.*sin(THE_Psi))./1.2e+1+(Ly_pend.^2.*THE_Theta_D.*m_pend.*cos(THE_Psi).*cos(THE_Psi_pend).^2.*sin(THE_Psi))./1.2e+1+(Ly_pend.^2.*THE_Theta_D.*m_pend.*cos(THE_Psi).*cos(THE_Theta_pend).^2.*sin(THE_Psi))./6.0+(Ly_pend.^2.*THE_Psi_pend_D.*m_pend.*cos(THE_Psi).*cos(THE_Phi_pend).^2.*sin(THE_Theta_pend))./6.0+(Ly_pend.^2.*THE_Psi_pend_D.*m_pend.*cos(THE_Psi).*cos(THE_Psi_pend).^2.*sin(THE_Theta_pend))./6.0+(Ly_pend.^2.*THE_Theta_pend_D.*m_pend.*cos(THE_Phi_pend).*cos(THE_Theta_pend).^2.*sin(THE_Psi))./6.0-(Lz_pend.^2.*THE_Theta_D.*m_pend.*cos(THE_Psi).*cos(THE_Phi_pend).^2.*sin(THE_Psi))./3.0-(Lz_pend.^2.*THE_Theta_D.*m_pend.*cos(THE_Psi).*cos(THE_Psi_pend).^2.*sin(THE_Psi))./3.0-Lz_pend.^2.*THE_Psi_pend_D.*m_pend.*cos(THE_Psi).*cos(THE_Phi_pend).^2.*sin(THE_Theta_pend).*(2.0./3.0)-Lz_pend.^2.*THE_Psi_pend_D.*m_pend.*cos(THE_Psi).*cos(THE_Psi_pend).^2.*sin(THE_Theta_pend).*(2.0./3.0);
    et253 = Lx_pend.^2.*THE_Phi_pend_D.*m_pend.*cos(THE_Psi).*cos(THE_Phi_pend).^2.*cos(THE_Theta_pend).^2.*(-1.0./6.0)+(Ly_pend.^2.*THE_Phi_pend_D.*m_pend.*cos(THE_Psi).*cos(THE_Phi_pend).^2.*cos(THE_Psi_pend).^2)./3.0+(Ly_pend.^2.*THE_Phi_pend_D.*m_pend.*cos(THE_Psi).*cos(THE_Phi_pend).^2.*cos(THE_Theta_pend).^2)./6.0+(Ly_pend.^2.*THE_Phi_pend_D.*m_pend.*cos(THE_Psi).*cos(THE_Psi_pend).^2.*cos(THE_Theta_pend).^2)./6.0-Lz_pend.^2.*THE_Phi_pend_D.*m_pend.*cos(THE_Psi).*cos(THE_Phi_pend).^2.*cos(THE_Psi_pend).^2.*(4.0./3.0)-Lz_pend.^2.*THE_Phi_pend_D.*m_pend.*cos(THE_Psi).*cos(THE_Psi_pend).^2.*cos(THE_Theta_pend).^2.*(2.0./3.0)+Lz_pend.*THE_Phi_pend_D.*Tv_Z_pend.*m_pend.*cos(THE_Phi_pend).*sin(THE_Psi).*sin(THE_Psi_pend)+Lz_pend.*THE_Psi_pend_D.*Tv_Z_pend.*m_pend.*cos(THE_Psi_pend).*sin(THE_Psi).*sin(THE_Phi_pend)+(Lz_pend.*THE_Theta_D.*Tv_Z_pend.*m_pend.*cos(THE_Psi_pend).*sin(THE_Phi_pend).*sin(THE_Theta_pend))./2.0+(Lx_pend.^2.*THE_Theta_D.*m_pend.*cos(THE_Psi).^2.*cos(THE_Theta_pend).*sin(THE_Phi_pend).*sin(THE_Theta_pend))./6.0-(Ly_pend.^2.*THE_Theta_D.*m_pend.*cos(THE_Psi).^2.*cos(THE_Theta_pend).*sin(THE_Phi_pend).*sin(THE_Theta_pend))./6.0;
    et254 = Ly_pend.^2.*THE_Psi_pend_D.*m_pend.*cos(THE_Psi_pend).^2.*cos(THE_Theta_pend).*sin(THE_Psi).*sin(THE_Phi_pend).*(-1.0./6.0)-(Ly_pend.^2.*THE_Theta_D.*m_pend.*cos(THE_Psi_pend).^2.*cos(THE_Theta_pend).*sin(THE_Phi_pend).*sin(THE_Theta_pend))./1.2e+1+Lz_pend.^2.*THE_Psi_pend_D.*m_pend.*cos(THE_Psi_pend).^2.*cos(THE_Theta_pend).*sin(THE_Psi).*sin(THE_Phi_pend).*(2.0./3.0)+(Lz_pend.^2.*THE_Theta_D.*m_pend.*cos(THE_Psi_pend).^2.*cos(THE_Theta_pend).*sin(THE_Phi_pend).*sin(THE_Theta_pend))./3.0+Lz_pend.*THE_Theta_D.*Tv_Z_pend.*m_pend.*cos(THE_Psi).^2.*cos(THE_Phi_pend).*sin(THE_Psi_pend)+(Lx_pend.^2.*THE_Theta_D.*m_pend.*cos(THE_Psi).*cos(THE_Phi_pend).^2.*cos(THE_Theta_pend).^2.*sin(THE_Psi))./1.2e+1-(Ly_pend.^2.*THE_Theta_D.*m_pend.*cos(THE_Psi).*cos(THE_Phi_pend).^2.*cos(THE_Psi_pend).^2.*sin(THE_Psi))./6.0-(Ly_pend.^2.*THE_Theta_D.*m_pend.*cos(THE_Psi).*cos(THE_Phi_pend).^2.*cos(THE_Theta_pend).^2.*sin(THE_Psi))./1.2e+1-(Ly_pend.^2.*THE_Theta_D.*m_pend.*cos(THE_Psi).*cos(THE_Psi_pend).^2.*cos(THE_Theta_pend).^2.*sin(THE_Psi))./6.0;
    et255 = Ly_pend.^2.*THE_Psi_pend_D.*m_pend.*cos(THE_Psi).*cos(THE_Phi_pend).^2.*cos(THE_Psi_pend).^2.*sin(THE_Theta_pend).*(-1.0./3.0)-(Ly_pend.^2.*THE_Theta_pend_D.*m_pend.*cos(THE_Phi_pend).*cos(THE_Psi_pend).^2.*cos(THE_Theta_pend).^2.*sin(THE_Psi))./6.0+Lz_pend.^2.*THE_Theta_D.*m_pend.*cos(THE_Psi).*cos(THE_Phi_pend).^2.*cos(THE_Psi_pend).^2.*sin(THE_Psi).*(2.0./3.0)+Lz_pend.^2.*THE_Theta_D.*m_pend.*cos(THE_Psi).*cos(THE_Psi_pend).^2.*cos(THE_Theta_pend).^2.*sin(THE_Psi).*(2.0./3.0)+Lz_pend.^2.*THE_Psi_pend_D.*m_pend.*cos(THE_Psi).*cos(THE_Phi_pend).^2.*cos(THE_Psi_pend).^2.*sin(THE_Theta_pend).*(4.0./3.0)+Lz_pend.^2.*THE_Theta_pend_D.*m_pend.*cos(THE_Phi_pend).*cos(THE_Psi_pend).^2.*cos(THE_Theta_pend).^2.*sin(THE_Psi).*(2.0./3.0)+(Ly_pend.^2.*THE_Theta_D.*m_pend.*cos(THE_Phi_pend).*cos(THE_Psi_pend).*cos(THE_Theta_pend).*sin(THE_Psi_pend))./1.2e+1-(Lz_pend.^2.*THE_Theta_D.*m_pend.*cos(THE_Phi_pend).*cos(THE_Psi_pend).*cos(THE_Theta_pend).*sin(THE_Psi_pend))./3.0-(Ly_pend.^2.*THE_Phi_pend_D.*m_pend.*cos(THE_Psi).*cos(THE_Phi_pend).^2.*cos(THE_Psi_pend).^2.*cos(THE_Theta_pend).^2)./6.0;
    et256 = Lz_pend.^2.*THE_Phi_pend_D.*m_pend.*cos(THE_Psi).*cos(THE_Phi_pend).^2.*cos(THE_Psi_pend).^2.*cos(THE_Theta_pend).^2.*(2.0./3.0)+(Lx_pend.^2.*THE_Phi_pend_D.*m_pend.*cos(THE_Theta_pend).*sin(THE_Psi).*sin(THE_Phi_pend).*sin(THE_Theta_pend))./6.0-(Ly_pend.^2.*THE_Phi_pend_D.*m_pend.*cos(THE_Theta_pend).*sin(THE_Psi).*sin(THE_Phi_pend).*sin(THE_Theta_pend))./6.0-Lz_pend.*THE_Theta_D.*Tv_Z_pend.*m_pend.*cos(THE_Psi).^2.*cos(THE_Psi_pend).*sin(THE_Phi_pend).*sin(THE_Theta_pend)+(Ly_pend.^2.*THE_Theta_D.*m_pend.*cos(THE_Psi).^2.*cos(THE_Psi_pend).^2.*cos(THE_Theta_pend).*sin(THE_Phi_pend).*sin(THE_Theta_pend))./6.0-Lz_pend.^2.*THE_Theta_D.*m_pend.*cos(THE_Psi).^2.*cos(THE_Psi_pend).^2.*cos(THE_Theta_pend).*sin(THE_Phi_pend).*sin(THE_Theta_pend).*(2.0./3.0)+(Lx_pend.^2.*THE_Theta_pend_D.*m_pend.*cos(THE_Psi).*cos(THE_Phi_pend).*cos(THE_Theta_pend).*sin(THE_Phi_pend).*sin(THE_Theta_pend))./6.0-(Ly_pend.^2.*THE_Psi_pend_D.*m_pend.*cos(THE_Psi).*cos(THE_Phi_pend).*cos(THE_Psi_pend).*sin(THE_Phi_pend).*sin(THE_Psi_pend))./3.0-(Ly_pend.^2.*THE_Phi_pend_D.*m_pend.*cos(THE_Phi_pend).*cos(THE_Psi_pend).*cos(THE_Theta_pend).*sin(THE_Psi).*sin(THE_Psi_pend))./6.0;
    et257 = Ly_pend.^2.*THE_Theta_pend_D.*m_pend.*cos(THE_Psi).*cos(THE_Phi_pend).*cos(THE_Theta_pend).*sin(THE_Phi_pend).*sin(THE_Theta_pend).*(-1.0./6.0)+Lz_pend.^2.*THE_Psi_pend_D.*m_pend.*cos(THE_Psi).*cos(THE_Phi_pend).*cos(THE_Psi_pend).*sin(THE_Phi_pend).*sin(THE_Psi_pend).*(4.0./3.0)+Lz_pend.^2.*THE_Phi_pend_D.*m_pend.*cos(THE_Phi_pend).*cos(THE_Psi_pend).*cos(THE_Theta_pend).*sin(THE_Psi).*sin(THE_Psi_pend).*(2.0./3.0)+(Ly_pend.^2.*THE_Theta_D.*m_pend.*cos(THE_Psi).*cos(THE_Phi_pend).^2.*cos(THE_Psi_pend).^2.*cos(THE_Theta_pend).^2.*sin(THE_Psi))./1.2e+1-(Lz_pend.^2.*THE_Theta_D.*m_pend.*cos(THE_Psi).*cos(THE_Phi_pend).^2.*cos(THE_Psi_pend).^2.*cos(THE_Theta_pend).^2.*sin(THE_Psi))./3.0+Lz_pend.*THE_Theta_D.*Tv_Z_pend.*m_pend.*cos(THE_Psi).*cos(THE_Psi_pend).*cos(THE_Theta_pend).*sin(THE_Psi)+Lz_pend.*THE_Theta_pend_D.*Tv_Z_pend.*m_pend.*cos(THE_Phi_pend).*cos(THE_Psi_pend).*cos(THE_Theta_pend).*sin(THE_Psi)-Lz_pend.*THE_Phi_pend_D.*Tv_Z_pend.*m_pend.*cos(THE_Psi_pend).*sin(THE_Psi).*sin(THE_Phi_pend).*sin(THE_Theta_pend)-Lz_pend.*THE_Psi_pend_D.*Tv_Z_pend.*m_pend.*cos(THE_Phi_pend).*sin(THE_Psi).*sin(THE_Psi_pend).*sin(THE_Theta_pend)-(Ly_pend.^2.*THE_Theta_D.*m_pend.*cos(THE_Psi).^2.*cos(THE_Phi_pend).*cos(THE_Psi_pend).*cos(THE_Theta_pend).*sin(THE_Psi_pend))./6.0;
    et258 = Ly_pend.^2.*THE_Theta_pend_D.*m_pend.*cos(THE_Psi).*cos(THE_Phi_pend).^2.*cos(THE_Psi_pend).*cos(THE_Theta_pend).*sin(THE_Psi_pend).*(-1.0./6.0)+Lz_pend.^2.*THE_Theta_D.*m_pend.*cos(THE_Psi).^2.*cos(THE_Phi_pend).*cos(THE_Psi_pend).*cos(THE_Theta_pend).*sin(THE_Psi_pend).*(2.0./3.0)+Lz_pend.^2.*THE_Theta_pend_D.*m_pend.*cos(THE_Psi).*cos(THE_Phi_pend).^2.*cos(THE_Psi_pend).*cos(THE_Theta_pend).*sin(THE_Psi_pend).*(2.0./3.0)+(Ly_pend.^2.*THE_Phi_pend_D.*m_pend.*cos(THE_Psi_pend).^2.*cos(THE_Theta_pend).*sin(THE_Psi).*sin(THE_Phi_pend).*sin(THE_Theta_pend))./6.0-Lz_pend.^2.*THE_Phi_pend_D.*m_pend.*cos(THE_Psi_pend).^2.*cos(THE_Theta_pend).*sin(THE_Psi).*sin(THE_Phi_pend).*sin(THE_Theta_pend).*(2.0./3.0)+(Ly_pend.^2.*THE_Phi_pend_D.*m_pend.*cos(THE_Psi).*cos(THE_Phi_pend).*cos(THE_Psi_pend).*sin(THE_Phi_pend).*sin(THE_Psi_pend).*sin(THE_Theta_pend))./3.0+(Ly_pend.^2.*THE_Psi_pend_D.*m_pend.*cos(THE_Phi_pend).*cos(THE_Psi_pend).*cos(THE_Theta_pend).*sin(THE_Psi).*sin(THE_Psi_pend).*sin(THE_Theta_pend))./6.0-Lz_pend.^2.*THE_Phi_pend_D.*m_pend.*cos(THE_Psi).*cos(THE_Phi_pend).*cos(THE_Psi_pend).*sin(THE_Phi_pend).*sin(THE_Psi_pend).*sin(THE_Theta_pend).*(4.0./3.0)-Lz_pend.^2.*THE_Psi_pend_D.*m_pend.*cos(THE_Phi_pend).*cos(THE_Psi_pend).*cos(THE_Theta_pend).*sin(THE_Psi).*sin(THE_Psi_pend).*sin(THE_Theta_pend).*(2.0./3.0);
    et259 = (Ly_pend.^2.*THE_Psi_pend_D.*m_pend.*cos(THE_Psi).*cos(THE_Phi_pend).*cos(THE_Psi_pend).*cos(THE_Theta_pend).^2.*sin(THE_Phi_pend).*sin(THE_Psi_pend))./6.0+(Ly_pend.^2.*THE_Theta_pend_D.*m_pend.*cos(THE_Psi).*cos(THE_Phi_pend).*cos(THE_Psi_pend).^2.*cos(THE_Theta_pend).*sin(THE_Phi_pend).*sin(THE_Theta_pend))./6.0-Lz_pend.^2.*THE_Psi_pend_D.*m_pend.*cos(THE_Psi).*cos(THE_Phi_pend).*cos(THE_Psi_pend).*cos(THE_Theta_pend).^2.*sin(THE_Phi_pend).*sin(THE_Psi_pend).*(2.0./3.0)-Lz_pend.^2.*THE_Theta_pend_D.*m_pend.*cos(THE_Psi).*cos(THE_Phi_pend).*cos(THE_Psi_pend).^2.*cos(THE_Theta_pend).*sin(THE_Phi_pend).*sin(THE_Theta_pend).*(2.0./3.0)-(Ly_pend.^2.*THE_Theta_D.*m_pend.*cos(THE_Psi).*cos(THE_Phi_pend).*cos(THE_Psi_pend).*sin(THE_Psi).*sin(THE_Phi_pend).*sin(THE_Psi_pend).*sin(THE_Theta_pend))./6.0+Lz_pend.^2.*THE_Theta_D.*m_pend.*cos(THE_Psi).*cos(THE_Phi_pend).*cos(THE_Psi_pend).*sin(THE_Psi).*sin(THE_Phi_pend).*sin(THE_Psi_pend).*sin(THE_Theta_pend).*(2.0./3.0);
    et260 = I_yz.*THE_Psi_D.*2.0+Iprop_yz.*THE_Psi_D.*8.0-I_yz.*THE_Psi_D.*cos(THE_Psi).^2.*4.0-Iprop_yz.*THE_Psi_D.*cos(THE_Psi).^2.*1.6e+1-I_yy.*THE_Psi_D.*sin(THE_Psi.*2.0)+I_zz.*THE_Psi_D.*sin(THE_Psi.*2.0)-Iprop_yy.*THE_Psi_D.*sin(THE_Psi.*2.0).*4.0+Iprop_zz.*THE_Psi_D.*sin(THE_Psi.*2.0).*4.0-THE_Psi_D.*cg_to_mot_H.^2.*mprop.*sin(THE_Psi.*2.0).*4.0+THE_Psi_D.*cg_to_mot_L.^2.*mprop.*sin(THE_Psi.*2.0).*2.0-(Lx_pend.^2.*THE_Psi_D.*m_pend.*sin(THE_Psi.*2.0))./1.2e+1-(Lx_pend.^2.*THE_Theta_pend_D.*m_pend.*sin(THE_Theta_pend.*2.0))./1.2e+1+(Ly_pend.^2.*THE_Psi_D.*m_pend.*sin(THE_Psi.*2.0))./1.2e+1+(Ly_pend.^2.*THE_Theta_pend_D.*m_pend.*sin(THE_Theta_pend.*2.0))./1.2e+1-THE_Psi_D.*Tv_Z_pend.^2.*m_pend.*sin(THE_Psi.*2.0)+(Lx_pend.^2.*THE_Theta_pend_D.*m_pend.*cos(THE_Psi).*sin(THE_Psi).*sin(THE_Phi_pend))./6.0+(Lx_pend.^2.*THE_Psi_D.*m_pend.*cos(THE_Theta_pend).*sin(THE_Phi_pend).*sin(THE_Theta_pend))./6.0-(Ly_pend.^2.*THE_Theta_pend_D.*m_pend.*cos(THE_Psi).*sin(THE_Psi).*sin(THE_Phi_pend))./6.0;
    et261 = Ly_pend.^2.*THE_Psi_D.*m_pend.*cos(THE_Theta_pend).*sin(THE_Phi_pend).*sin(THE_Theta_pend).*(-1.0./6.0)+Lz_pend.*THE_Psi_D.*Tv_Z_pend.*m_pend.*cos(THE_Phi_pend).*sin(THE_Psi_pend)+(Lx_pend.^2.*THE_Psi_D.*m_pend.*cos(THE_Psi).*cos(THE_Theta_pend).^2.*sin(THE_Psi))./3.0+(Lx_pend.^2.*THE_Theta_pend_D.*m_pend.*cos(THE_Psi).^2.*cos(THE_Theta_pend).*sin(THE_Theta_pend))./3.0-(Ly_pend.^2.*THE_Psi_D.*m_pend.*cos(THE_Psi).*cos(THE_Phi_pend).^2.*sin(THE_Psi))./6.0-(Ly_pend.^2.*THE_Psi_D.*m_pend.*cos(THE_Psi).*cos(THE_Psi_pend).^2.*sin(THE_Psi))./6.0-(Ly_pend.^2.*THE_Psi_D.*m_pend.*cos(THE_Psi).*cos(THE_Theta_pend).^2.*sin(THE_Psi))./3.0-(Ly_pend.^2.*THE_Phi_pend_D.*m_pend.*cos(THE_Psi).^2.*cos(THE_Phi_pend).*sin(THE_Phi_pend))./6.0-(Ly_pend.^2.*THE_Psi_pend_D.*m_pend.*cos(THE_Psi).^2.*cos(THE_Psi_pend).*sin(THE_Psi_pend))./6.0-(Ly_pend.^2.*THE_Theta_pend_D.*m_pend.*cos(THE_Psi).^2.*cos(THE_Theta_pend).*sin(THE_Theta_pend))./3.0-(Ly_pend.^2.*THE_Psi_pend_D.*m_pend.*cos(THE_Psi_pend).*cos(THE_Theta_pend).^2.*sin(THE_Psi_pend))./6.0;
    et262 = Ly_pend.^2.*THE_Theta_pend_D.*m_pend.*cos(THE_Psi_pend).^2.*cos(THE_Theta_pend).*sin(THE_Theta_pend).*(-1.0./6.0)+Lz_pend.^2.*THE_Psi_D.*m_pend.*cos(THE_Psi).*cos(THE_Phi_pend).^2.*sin(THE_Psi).*(2.0./3.0)+Lz_pend.^2.*THE_Psi_D.*m_pend.*cos(THE_Psi).*cos(THE_Psi_pend).^2.*sin(THE_Psi).*(2.0./3.0)+Lz_pend.^2.*THE_Phi_pend_D.*m_pend.*cos(THE_Psi).^2.*cos(THE_Phi_pend).*sin(THE_Phi_pend).*(2.0./3.0)+Lz_pend.^2.*THE_Psi_pend_D.*m_pend.*cos(THE_Psi).^2.*cos(THE_Psi_pend).*sin(THE_Psi_pend).*(2.0./3.0)+Lz_pend.^2.*THE_Psi_pend_D.*m_pend.*cos(THE_Psi_pend).*cos(THE_Theta_pend).^2.*sin(THE_Psi_pend).*(2.0./3.0)+Lz_pend.^2.*THE_Theta_pend_D.*m_pend.*cos(THE_Psi_pend).^2.*cos(THE_Theta_pend).*sin(THE_Theta_pend).*(2.0./3.0)-Lz_pend.*THE_Psi_D.*Tv_Z_pend.*m_pend.*cos(THE_Psi_pend).*sin(THE_Phi_pend).*sin(THE_Theta_pend)-(Lx_pend.^2.*THE_Psi_D.*m_pend.*cos(THE_Psi).^2.*cos(THE_Theta_pend).*sin(THE_Phi_pend).*sin(THE_Theta_pend))./3.0-(Lx_pend.^2.*THE_Theta_pend_D.*m_pend.*cos(THE_Psi).*cos(THE_Theta_pend).^2.*sin(THE_Psi).*sin(THE_Phi_pend))./3.0+(Ly_pend.^2.*THE_Theta_pend_D.*m_pend.*cos(THE_Psi).*cos(THE_Psi_pend).^2.*sin(THE_Psi).*sin(THE_Phi_pend))./6.0;
    et263 = (Ly_pend.^2.*THE_Psi_D.*m_pend.*cos(THE_Psi).^2.*cos(THE_Theta_pend).*sin(THE_Phi_pend).*sin(THE_Theta_pend))./3.0+(Ly_pend.^2.*THE_Theta_pend_D.*m_pend.*cos(THE_Psi).*cos(THE_Theta_pend).^2.*sin(THE_Psi).*sin(THE_Phi_pend))./3.0+(Ly_pend.^2.*THE_Psi_pend_D.*m_pend.*cos(THE_Psi).^2.*cos(THE_Phi_pend).*sin(THE_Phi_pend).*sin(THE_Theta_pend))./6.0+(Ly_pend.^2.*THE_Phi_pend_D.*m_pend.*cos(THE_Psi).^2.*cos(THE_Psi_pend).*sin(THE_Psi_pend).*sin(THE_Theta_pend))./6.0+(Ly_pend.^2.*THE_Psi_D.*m_pend.*cos(THE_Psi_pend).^2.*cos(THE_Theta_pend).*sin(THE_Phi_pend).*sin(THE_Theta_pend))./6.0-Lz_pend.^2.*THE_Theta_pend_D.*m_pend.*cos(THE_Psi).*cos(THE_Psi_pend).^2.*sin(THE_Psi).*sin(THE_Phi_pend).*(2.0./3.0)-Lz_pend.^2.*THE_Psi_pend_D.*m_pend.*cos(THE_Psi).^2.*cos(THE_Phi_pend).*sin(THE_Phi_pend).*sin(THE_Theta_pend).*(2.0./3.0)-Lz_pend.^2.*THE_Phi_pend_D.*m_pend.*cos(THE_Psi).^2.*cos(THE_Psi_pend).*sin(THE_Psi_pend).*sin(THE_Theta_pend).*(2.0./3.0)-Lz_pend.^2.*THE_Psi_D.*m_pend.*cos(THE_Psi_pend).^2.*cos(THE_Theta_pend).*sin(THE_Phi_pend).*sin(THE_Theta_pend).*(2.0./3.0)-Lz_pend.*THE_Psi_D.*Tv_Z_pend.*m_pend.*cos(THE_Psi).^2.*cos(THE_Phi_pend).*sin(THE_Psi_pend).*2.0;
    et264 = -Lz_pend.*THE_Psi_pend_D.*Tv_Z_pend.*m_pend.*cos(THE_Psi).^2.*cos(THE_Theta_pend).*sin(THE_Psi_pend)-Lz_pend.*THE_Theta_pend_D.*Tv_Z_pend.*m_pend.*cos(THE_Psi).^2.*cos(THE_Psi_pend).*sin(THE_Theta_pend)-(Lx_pend.^2.*THE_Psi_D.*m_pend.*cos(THE_Psi).*cos(THE_Phi_pend).^2.*cos(THE_Theta_pend).^2.*sin(THE_Psi))./6.0-(Lx_pend.^2.*THE_Phi_pend_D.*m_pend.*cos(THE_Psi).^2.*cos(THE_Phi_pend).*cos(THE_Theta_pend).^2.*sin(THE_Phi_pend))./6.0-(Lx_pend.^2.*THE_Theta_pend_D.*m_pend.*cos(THE_Psi).^2.*cos(THE_Phi_pend).^2.*cos(THE_Theta_pend).*sin(THE_Theta_pend))./6.0+(Ly_pend.^2.*THE_Psi_D.*m_pend.*cos(THE_Psi).*cos(THE_Phi_pend).^2.*cos(THE_Psi_pend).^2.*sin(THE_Psi))./3.0+(Ly_pend.^2.*THE_Psi_D.*m_pend.*cos(THE_Psi).*cos(THE_Phi_pend).^2.*cos(THE_Theta_pend).^2.*sin(THE_Psi))./6.0+(Ly_pend.^2.*THE_Psi_D.*m_pend.*cos(THE_Psi).*cos(THE_Psi_pend).^2.*cos(THE_Theta_pend).^2.*sin(THE_Psi))./3.0+(Ly_pend.^2.*THE_Phi_pend_D.*m_pend.*cos(THE_Psi).^2.*cos(THE_Phi_pend).*cos(THE_Psi_pend).^2.*sin(THE_Phi_pend))./3.0;
    et265 = (Ly_pend.^2.*THE_Psi_pend_D.*m_pend.*cos(THE_Psi).^2.*cos(THE_Phi_pend).^2.*cos(THE_Psi_pend).*sin(THE_Psi_pend))./3.0+(Ly_pend.^2.*THE_Phi_pend_D.*m_pend.*cos(THE_Psi).^2.*cos(THE_Phi_pend).*cos(THE_Theta_pend).^2.*sin(THE_Phi_pend))./6.0+(Ly_pend.^2.*THE_Psi_pend_D.*m_pend.*cos(THE_Psi).^2.*cos(THE_Psi_pend).*cos(THE_Theta_pend).^2.*sin(THE_Psi_pend))./3.0+(Ly_pend.^2.*THE_Theta_pend_D.*m_pend.*cos(THE_Psi).^2.*cos(THE_Phi_pend).^2.*cos(THE_Theta_pend).*sin(THE_Theta_pend))./6.0+(Ly_pend.^2.*THE_Theta_pend_D.*m_pend.*cos(THE_Psi).^2.*cos(THE_Psi_pend).^2.*cos(THE_Theta_pend).*sin(THE_Theta_pend))./3.0-Lz_pend.^2.*THE_Psi_D.*m_pend.*cos(THE_Psi).*cos(THE_Phi_pend).^2.*cos(THE_Psi_pend).^2.*sin(THE_Psi).*(4.0./3.0)-Lz_pend.^2.*THE_Psi_D.*m_pend.*cos(THE_Psi).*cos(THE_Psi_pend).^2.*cos(THE_Theta_pend).^2.*sin(THE_Psi).*(4.0./3.0)-Lz_pend.^2.*THE_Phi_pend_D.*m_pend.*cos(THE_Psi).^2.*cos(THE_Phi_pend).*cos(THE_Psi_pend).^2.*sin(THE_Phi_pend).*(4.0./3.0)-Lz_pend.^2.*THE_Psi_pend_D.*m_pend.*cos(THE_Psi).^2.*cos(THE_Phi_pend).^2.*cos(THE_Psi_pend).*sin(THE_Psi_pend).*(4.0./3.0);
    et266 = Lz_pend.^2.*THE_Psi_pend_D.*m_pend.*cos(THE_Psi).^2.*cos(THE_Psi_pend).*cos(THE_Theta_pend).^2.*sin(THE_Psi_pend).*(-4.0./3.0)-Lz_pend.^2.*THE_Theta_pend_D.*m_pend.*cos(THE_Psi).^2.*cos(THE_Psi_pend).^2.*cos(THE_Theta_pend).*sin(THE_Theta_pend).*(4.0./3.0)-(Ly_pend.^2.*THE_Psi_pend_D.*m_pend.*cos(THE_Psi).*cos(THE_Phi_pend).*cos(THE_Theta_pend).*sin(THE_Psi))./6.0-(Ly_pend.^2.*THE_Psi_D.*m_pend.*cos(THE_Phi_pend).*cos(THE_Psi_pend).*cos(THE_Theta_pend).*sin(THE_Psi_pend))./6.0+Lz_pend.^2.*THE_Psi_pend_D.*m_pend.*cos(THE_Psi).*cos(THE_Phi_pend).*cos(THE_Theta_pend).*sin(THE_Psi).*(2.0./3.0)+Lz_pend.^2.*THE_Psi_D.*m_pend.*cos(THE_Phi_pend).*cos(THE_Psi_pend).*cos(THE_Theta_pend).*sin(THE_Psi_pend).*(2.0./3.0)+Lz_pend.*THE_Psi_D.*Tv_Z_pend.*m_pend.*cos(THE_Psi).^2.*cos(THE_Psi_pend).*sin(THE_Phi_pend).*sin(THE_Theta_pend).*2.0-(Ly_pend.^2.*THE_Psi_D.*m_pend.*cos(THE_Psi).^2.*cos(THE_Psi_pend).^2.*cos(THE_Theta_pend).*sin(THE_Phi_pend).*sin(THE_Theta_pend))./3.0-(Ly_pend.^2.*THE_Theta_pend_D.*m_pend.*cos(THE_Psi).*cos(THE_Psi_pend).^2.*cos(THE_Theta_pend).^2.*sin(THE_Psi).*sin(THE_Phi_pend))./3.0;
    et267 = Ly_pend.^2.*THE_Phi_pend_D.*m_pend.*cos(THE_Psi).^2.*cos(THE_Phi_pend).^2.*cos(THE_Psi_pend).*sin(THE_Psi_pend).*sin(THE_Theta_pend).*(-1.0./3.0)-(Ly_pend.^2.*THE_Psi_pend_D.*m_pend.*cos(THE_Psi).^2.*cos(THE_Phi_pend).*cos(THE_Psi_pend).^2.*sin(THE_Phi_pend).*sin(THE_Theta_pend))./3.0+Lz_pend.^2.*THE_Psi_D.*m_pend.*cos(THE_Psi).^2.*cos(THE_Psi_pend).^2.*cos(THE_Theta_pend).*sin(THE_Phi_pend).*sin(THE_Theta_pend).*(4.0./3.0)+Lz_pend.^2.*THE_Theta_pend_D.*m_pend.*cos(THE_Psi).*cos(THE_Psi_pend).^2.*cos(THE_Theta_pend).^2.*sin(THE_Psi).*sin(THE_Phi_pend).*(4.0./3.0)+Lz_pend.^2.*THE_Phi_pend_D.*m_pend.*cos(THE_Psi).^2.*cos(THE_Phi_pend).^2.*cos(THE_Psi_pend).*sin(THE_Psi_pend).*sin(THE_Theta_pend).*(4.0./3.0)+Lz_pend.^2.*THE_Psi_pend_D.*m_pend.*cos(THE_Psi).^2.*cos(THE_Phi_pend).*cos(THE_Psi_pend).^2.*sin(THE_Phi_pend).*sin(THE_Theta_pend).*(4.0./3.0)-(Lx_pend.^2.*THE_Phi_pend_D.*m_pend.*cos(THE_Psi).*cos(THE_Phi_pend).*cos(THE_Theta_pend).*sin(THE_Psi).*sin(THE_Theta_pend))./6.0+(Ly_pend.^2.*THE_Phi_pend_D.*m_pend.*cos(THE_Psi).*cos(THE_Phi_pend).*cos(THE_Theta_pend).*sin(THE_Psi).*sin(THE_Theta_pend))./6.0;
    et268 = Ly_pend.^2.*THE_Psi_D.*m_pend.*cos(THE_Psi).*cos(THE_Phi_pend).^2.*cos(THE_Psi_pend).^2.*cos(THE_Theta_pend).^2.*sin(THE_Psi).*(-1.0./6.0)-(Ly_pend.^2.*THE_Phi_pend_D.*m_pend.*cos(THE_Psi).^2.*cos(THE_Phi_pend).*cos(THE_Psi_pend).^2.*cos(THE_Theta_pend).^2.*sin(THE_Phi_pend))./6.0-(Ly_pend.^2.*THE_Psi_pend_D.*m_pend.*cos(THE_Psi).^2.*cos(THE_Phi_pend).^2.*cos(THE_Psi_pend).*cos(THE_Theta_pend).^2.*sin(THE_Psi_pend))./6.0-(Ly_pend.^2.*THE_Theta_pend_D.*m_pend.*cos(THE_Psi).^2.*cos(THE_Phi_pend).^2.*cos(THE_Psi_pend).^2.*cos(THE_Theta_pend).*sin(THE_Theta_pend))./6.0+Lz_pend.^2.*THE_Psi_D.*m_pend.*cos(THE_Psi).*cos(THE_Phi_pend).^2.*cos(THE_Psi_pend).^2.*cos(THE_Theta_pend).^2.*sin(THE_Psi).*(2.0./3.0)+Lz_pend.^2.*THE_Phi_pend_D.*m_pend.*cos(THE_Psi).^2.*cos(THE_Phi_pend).*cos(THE_Psi_pend).^2.*cos(THE_Theta_pend).^2.*sin(THE_Phi_pend).*(2.0./3.0)+Lz_pend.^2.*THE_Psi_pend_D.*m_pend.*cos(THE_Psi).^2.*cos(THE_Phi_pend).^2.*cos(THE_Psi_pend).*cos(THE_Theta_pend).^2.*sin(THE_Psi_pend).*(2.0./3.0);
    et269 = Lz_pend.^2.*THE_Theta_pend_D.*m_pend.*cos(THE_Psi).^2.*cos(THE_Phi_pend).^2.*cos(THE_Psi_pend).^2.*cos(THE_Theta_pend).*sin(THE_Theta_pend).*(2.0./3.0)-Lz_pend.*THE_Psi_D.*Tv_Z_pend.*m_pend.*cos(THE_Psi).*cos(THE_Psi_pend).*cos(THE_Theta_pend).*sin(THE_Psi).*2.0-Lz_pend.*THE_Psi_pend_D.*Tv_Z_pend.*m_pend.*cos(THE_Psi).*cos(THE_Phi_pend).*cos(THE_Psi_pend).*sin(THE_Psi)+Lz_pend.*THE_Phi_pend_D.*Tv_Z_pend.*m_pend.*cos(THE_Psi).*sin(THE_Psi).*sin(THE_Phi_pend).*sin(THE_Psi_pend)+(Ly_pend.^2.*THE_Psi_D.*m_pend.*cos(THE_Psi).^2.*cos(THE_Phi_pend).*cos(THE_Psi_pend).*cos(THE_Theta_pend).*sin(THE_Psi_pend))./3.0+(Ly_pend.^2.*THE_Psi_pend_D.*m_pend.*cos(THE_Psi).*cos(THE_Phi_pend).*cos(THE_Psi_pend).^2.*cos(THE_Theta_pend).*sin(THE_Psi))./3.0-Lz_pend.^2.*THE_Psi_D.*m_pend.*cos(THE_Psi).^2.*cos(THE_Phi_pend).*cos(THE_Psi_pend).*cos(THE_Theta_pend).*sin(THE_Psi_pend).*(4.0./3.0)-Lz_pend.^2.*THE_Psi_pend_D.*m_pend.*cos(THE_Psi).*cos(THE_Phi_pend).*cos(THE_Psi_pend).^2.*cos(THE_Theta_pend).*sin(THE_Psi).*(4.0./3.0)-(Ly_pend.^2.*THE_Phi_pend_D.*m_pend.*cos(THE_Psi).*cos(THE_Psi_pend).*cos(THE_Theta_pend).*sin(THE_Psi).*sin(THE_Phi_pend).*sin(THE_Psi_pend))./6.0-(Ly_pend.^2.*THE_Theta_pend_D.*m_pend.*cos(THE_Psi).*cos(THE_Phi_pend).*cos(THE_Psi_pend).*sin(THE_Psi).*sin(THE_Psi_pend).*sin(THE_Theta_pend))./6.0;
    et270 = Lz_pend.^2.*THE_Phi_pend_D.*m_pend.*cos(THE_Psi).*cos(THE_Psi_pend).*cos(THE_Theta_pend).*sin(THE_Psi).*sin(THE_Phi_pend).*sin(THE_Psi_pend).*(2.0./3.0)+Lz_pend.^2.*THE_Theta_pend_D.*m_pend.*cos(THE_Psi).*cos(THE_Phi_pend).*cos(THE_Psi_pend).*sin(THE_Psi).*sin(THE_Psi_pend).*sin(THE_Theta_pend).*(2.0./3.0)+Lz_pend.*THE_Phi_pend_D.*Tv_Z_pend.*m_pend.*cos(THE_Psi).*cos(THE_Phi_pend).*cos(THE_Psi_pend).*sin(THE_Psi).*sin(THE_Theta_pend)+Lz_pend.*THE_Theta_pend_D.*Tv_Z_pend.*m_pend.*cos(THE_Psi).*cos(THE_Psi_pend).*cos(THE_Theta_pend).*sin(THE_Psi).*sin(THE_Phi_pend)-Lz_pend.*THE_Psi_pend_D.*Tv_Z_pend.*m_pend.*cos(THE_Psi).*sin(THE_Psi).*sin(THE_Phi_pend).*sin(THE_Psi_pend).*sin(THE_Theta_pend)-(Ly_pend.^2.*THE_Phi_pend_D.*m_pend.*cos(THE_Psi).*cos(THE_Phi_pend).*cos(THE_Psi_pend).^2.*cos(THE_Theta_pend).*sin(THE_Psi).*sin(THE_Theta_pend))./6.0-(Ly_pend.^2.*THE_Theta_pend_D.*m_pend.*cos(THE_Psi).^2.*cos(THE_Phi_pend).*cos(THE_Psi_pend).*cos(THE_Theta_pend).*sin(THE_Phi_pend).*sin(THE_Psi_pend))./6.0+Lz_pend.^2.*THE_Phi_pend_D.*m_pend.*cos(THE_Psi).*cos(THE_Phi_pend).*cos(THE_Psi_pend).^2.*cos(THE_Theta_pend).*sin(THE_Psi).*sin(THE_Theta_pend).*(2.0./3.0)+Lz_pend.^2.*THE_Theta_pend_D.*m_pend.*cos(THE_Psi).^2.*cos(THE_Phi_pend).*cos(THE_Psi_pend).*cos(THE_Theta_pend).*sin(THE_Phi_pend).*sin(THE_Psi_pend).*(2.0./3.0);
    et271 = (Ly_pend.^2.*THE_Psi_D.*m_pend.*cos(THE_Psi).*cos(THE_Phi_pend).*cos(THE_Psi_pend).*sin(THE_Psi).*sin(THE_Phi_pend).*sin(THE_Psi_pend).*sin(THE_Theta_pend))./3.0+(Ly_pend.^2.*THE_Psi_pend_D.*m_pend.*cos(THE_Psi).*cos(THE_Psi_pend).*cos(THE_Theta_pend).*sin(THE_Psi).*sin(THE_Phi_pend).*sin(THE_Psi_pend).*sin(THE_Theta_pend))./3.0-Lz_pend.^2.*THE_Psi_D.*m_pend.*cos(THE_Psi).*cos(THE_Phi_pend).*cos(THE_Psi_pend).*sin(THE_Psi).*sin(THE_Phi_pend).*sin(THE_Psi_pend).*sin(THE_Theta_pend).*(4.0./3.0)-Lz_pend.^2.*THE_Psi_pend_D.*m_pend.*cos(THE_Psi).*cos(THE_Psi_pend).*cos(THE_Theta_pend).*sin(THE_Psi).*sin(THE_Phi_pend).*sin(THE_Psi_pend).*sin(THE_Theta_pend).*(4.0./3.0);
    et272 = -I_xx.*THE_Psi_D.*cos(THE_Theta)-I_yy.*THE_Psi_D.*cos(THE_Theta)+I_zz.*THE_Psi_D.*cos(THE_Theta)-Iprop_xx.*THE_Psi_D.*cos(THE_Theta).*4.0-Iprop_yy.*THE_Psi_D.*cos(THE_Theta).*4.0+Iprop_zz.*THE_Psi_D.*cos(THE_Theta).*4.0+I_yz.*THE_Theta_D.*sin(THE_Theta)+Iprop_yz.*THE_Theta_D.*sin(THE_Theta).*4.0-Iprop_xz.*wMOT_1.*cos(THE_Theta)-Iprop_xz.*wMOT_2.*cos(THE_Theta)-Iprop_xz.*wMOT_3.*cos(THE_Theta)-Iprop_xz.*wMOT_4.*cos(THE_Theta)-I_xy.*THE_Theta_D.*cos(THE_Psi).*cos(THE_Theta)-Iprop_xy.*THE_Theta_D.*cos(THE_Psi).*cos(THE_Theta).*4.0+I_xz.*THE_Theta_D.*cos(THE_Theta).*sin(THE_Psi)+Iprop_xz.*THE_Theta_D.*cos(THE_Theta).*sin(THE_Psi).*4.0-(Lx_pend.^2.*THE_Psi_D.*m_pend.*cos(THE_Theta))./6.0-THE_Psi_D.*Tv_Z_pend.^2.*m_pend.*cos(THE_Theta).*2.0-THE_Psi_D.*cg_to_mot_H.^2.*mprop.*cos(THE_Theta).*8.0-Iprop_zz.*wMOT_1.*cos(THE_Psi).*sin(THE_Theta)-Iprop_zz.*wMOT_2.*cos(THE_Psi).*sin(THE_Theta)-Iprop_zz.*wMOT_3.*cos(THE_Psi).*sin(THE_Theta)-Iprop_zz.*wMOT_4.*cos(THE_Psi).*sin(THE_Theta)-Iprop_yz.*wMOT_1.*sin(THE_Psi).*sin(THE_Theta)-Iprop_yz.*wMOT_2.*sin(THE_Psi).*sin(THE_Theta);
    et273 = -Iprop_yz.*wMOT_3.*sin(THE_Psi).*sin(THE_Theta)-Iprop_yz.*wMOT_4.*sin(THE_Psi).*sin(THE_Theta)+I_yy.*THE_Psi_D.*cos(THE_Psi).^2.*cos(THE_Theta).*2.0-I_zz.*THE_Psi_D.*cos(THE_Psi).^2.*cos(THE_Theta).*2.0+Iprop_yy.*THE_Psi_D.*cos(THE_Psi).^2.*cos(THE_Theta).*8.0-Iprop_zz.*THE_Psi_D.*cos(THE_Psi).^2.*cos(THE_Theta).*8.0-I_yz.*THE_Theta_D.*cos(THE_Psi).^2.*sin(THE_Theta).*2.0-Iprop_yz.*THE_Theta_D.*cos(THE_Psi).^2.*sin(THE_Theta).*8.0-I_yz.*THE_Psi_D.*cos(THE_Psi).*cos(THE_Theta).*sin(THE_Psi).*4.0-Iprop_yz.*THE_Psi_D.*cos(THE_Psi).*cos(THE_Theta).*sin(THE_Psi).*1.6e+1-I_yy.*THE_Theta_D.*cos(THE_Psi).*sin(THE_Psi).*sin(THE_Theta)+I_zz.*THE_Theta_D.*cos(THE_Psi).*sin(THE_Psi).*sin(THE_Theta)-Iprop_yy.*THE_Theta_D.*cos(THE_Psi).*sin(THE_Psi).*sin(THE_Theta).*4.0+Iprop_zz.*THE_Theta_D.*cos(THE_Psi).*sin(THE_Psi).*sin(THE_Theta).*4.0+(Lx_pend.^2.*THE_Theta_pend_D.*m_pend.*cos(THE_Theta).*sin(THE_Phi_pend))./6.0-(Ly_pend.^2.*THE_Phi_pend_D.*m_pend.*cos(THE_Psi).*sin(THE_Theta))./6.0+(Lx_pend.^2.*THE_Psi_D.*m_pend.*cos(THE_Psi).^2.*cos(THE_Theta))./6.0;
    et274 = (Lx_pend.^2.*THE_Psi_D.*m_pend.*cos(THE_Theta).*cos(THE_Theta_pend).^2)./6.0-(Ly_pend.^2.*THE_Psi_D.*m_pend.*cos(THE_Psi).^2.*cos(THE_Theta))./6.0-(Ly_pend.^2.*THE_Psi_D.*m_pend.*cos(THE_Theta).*cos(THE_Theta_pend).^2)./6.0+THE_Psi_D.*Tv_Z_pend.^2.*m_pend.*cos(THE_Psi).^2.*cos(THE_Theta).*2.0+THE_Psi_D.*cg_to_mot_H.^2.*mprop.*cos(THE_Psi).^2.*cos(THE_Theta).*8.0-THE_Psi_D.*cg_to_mot_L.^2.*mprop.*cos(THE_Psi).^2.*cos(THE_Theta).*4.0-(Lx_pend.^2.*THE_Theta_D.*m_pend.*cos(THE_Psi).*sin(THE_Psi).*sin(THE_Theta))./1.2e+1-(Lx_pend.^2.*THE_Theta_pend_D.*m_pend.*cos(THE_Phi_pend).*sin(THE_Psi).*sin(THE_Theta))./6.0+(Ly_pend.^2.*THE_Theta_D.*m_pend.*cos(THE_Psi).*sin(THE_Psi).*sin(THE_Theta))./1.2e+1+(Ly_pend.^2.*THE_Psi_pend_D.*m_pend.*cos(THE_Psi).*sin(THE_Theta).*sin(THE_Theta_pend))./6.0-THE_Theta_D.*Tv_Z_pend.^2.*m_pend.*cos(THE_Psi).*sin(THE_Psi).*sin(THE_Theta)-THE_Theta_D.*cg_to_mot_H.^2.*mprop.*cos(THE_Psi).*sin(THE_Psi).*sin(THE_Theta).*4.0+THE_Theta_D.*cg_to_mot_L.^2.*mprop.*cos(THE_Psi).*sin(THE_Psi).*sin(THE_Theta).*2.0;
    et275 = Lx_pend.^2.*THE_Phi_pend_D.*m_pend.*cos(THE_Psi).*cos(THE_Theta_pend).^2.*sin(THE_Theta).*(-1.0./6.0)-(Lx_pend.^2.*THE_Theta_pend_D.*m_pend.*cos(THE_Psi).^2.*cos(THE_Theta).*sin(THE_Phi_pend))./6.0-(Lx_pend.^2.*THE_Theta_pend_D.*m_pend.*cos(THE_Theta).*cos(THE_Theta_pend).^2.*sin(THE_Phi_pend))./6.0+(Ly_pend.^2.*THE_Phi_pend_D.*m_pend.*cos(THE_Psi).*cos(THE_Phi_pend).^2.*sin(THE_Theta))./6.0+(Ly_pend.^2.*THE_Phi_pend_D.*m_pend.*cos(THE_Psi).*cos(THE_Psi_pend).^2.*sin(THE_Theta))./6.0+(Ly_pend.^2.*THE_Phi_pend_D.*m_pend.*cos(THE_Psi).*cos(THE_Theta_pend).^2.*sin(THE_Theta))./6.0+(Ly_pend.^2.*THE_Theta_pend_D.*m_pend.*cos(THE_Psi).^2.*cos(THE_Theta).*sin(THE_Phi_pend))./6.0+(Ly_pend.^2.*THE_Theta_pend_D.*m_pend.*cos(THE_Theta).*cos(THE_Theta_pend).^2.*sin(THE_Phi_pend))./6.0-Lz_pend.^2.*THE_Phi_pend_D.*m_pend.*cos(THE_Psi).*cos(THE_Phi_pend).^2.*sin(THE_Theta).*(2.0./3.0)-Lz_pend.^2.*THE_Phi_pend_D.*m_pend.*cos(THE_Psi).*cos(THE_Psi_pend).^2.*sin(THE_Theta).*(2.0./3.0)-(Lx_pend.^2.*THE_Psi_D.*m_pend.*cos(THE_Psi).^2.*cos(THE_Theta).*cos(THE_Theta_pend).^2)./3.0;
    et276 = (Ly_pend.^2.*THE_Psi_D.*m_pend.*cos(THE_Psi).^2.*cos(THE_Theta).*cos(THE_Phi_pend).^2)./6.0+(Ly_pend.^2.*THE_Psi_D.*m_pend.*cos(THE_Psi).^2.*cos(THE_Theta).*cos(THE_Psi_pend).^2)./6.0+(Ly_pend.^2.*THE_Psi_D.*m_pend.*cos(THE_Psi).^2.*cos(THE_Theta).*cos(THE_Theta_pend).^2)./3.0+(Ly_pend.^2.*THE_Psi_D.*m_pend.*cos(THE_Theta).*cos(THE_Psi_pend).^2.*cos(THE_Theta_pend).^2)./6.0-Lz_pend.^2.*THE_Psi_D.*m_pend.*cos(THE_Psi).^2.*cos(THE_Theta).*cos(THE_Phi_pend).^2.*(2.0./3.0)-Lz_pend.^2.*THE_Psi_D.*m_pend.*cos(THE_Psi).^2.*cos(THE_Theta).*cos(THE_Psi_pend).^2.*(2.0./3.0)-Lz_pend.^2.*THE_Psi_D.*m_pend.*cos(THE_Theta).*cos(THE_Psi_pend).^2.*cos(THE_Theta_pend).^2.*(2.0./3.0)-(Ly_pend.^2.*THE_Psi_pend_D.*m_pend.*cos(THE_Theta).*cos(THE_Phi_pend).*cos(THE_Theta_pend))./6.0+(Lz_pend.*THE_Theta_D.*Tv_Z_pend.*m_pend.*cos(THE_Phi_pend).*sin(THE_Theta).*sin(THE_Psi_pend))./2.0+Lz_pend.*THE_Phi_pend_D.*Tv_Z_pend.*m_pend.*cos(THE_Theta).*sin(THE_Phi_pend).*sin(THE_Psi_pend)+(Ly_pend.^2.*THE_Psi_pend_D.*m_pend.*cos(THE_Psi).^2.*cos(THE_Theta).*cos(THE_Phi_pend).*cos(THE_Theta_pend))./6.0;
    et277 = (Ly_pend.^2.*THE_Psi_pend_D.*m_pend.*cos(THE_Theta).*cos(THE_Phi_pend).*cos(THE_Psi_pend).^2.*cos(THE_Theta_pend))./6.0-Lz_pend.^2.*THE_Psi_pend_D.*m_pend.*cos(THE_Psi).^2.*cos(THE_Theta).*cos(THE_Phi_pend).*cos(THE_Theta_pend).*(2.0./3.0)-Lz_pend.^2.*THE_Psi_pend_D.*m_pend.*cos(THE_Theta).*cos(THE_Phi_pend).*cos(THE_Psi_pend).^2.*cos(THE_Theta_pend).*(2.0./3.0)+(Lx_pend.^2.*THE_Theta_D.*m_pend.*cos(THE_Psi).*cos(THE_Theta_pend).^2.*sin(THE_Psi).*sin(THE_Theta))./6.0+(Lx_pend.^2.*THE_Theta_pend_D.*m_pend.*cos(THE_Phi_pend).*cos(THE_Theta_pend).^2.*sin(THE_Psi).*sin(THE_Theta))./6.0-(Ly_pend.^2.*THE_Theta_D.*m_pend.*cos(THE_Psi).*cos(THE_Phi_pend).^2.*sin(THE_Psi).*sin(THE_Theta))./1.2e+1-(Ly_pend.^2.*THE_Theta_D.*m_pend.*cos(THE_Psi).*cos(THE_Psi_pend).^2.*sin(THE_Psi).*sin(THE_Theta))./1.2e+1-(Ly_pend.^2.*THE_Theta_D.*m_pend.*cos(THE_Psi).*cos(THE_Theta_pend).^2.*sin(THE_Psi).*sin(THE_Theta))./6.0-(Ly_pend.^2.*THE_Psi_pend_D.*m_pend.*cos(THE_Psi).*cos(THE_Phi_pend).^2.*sin(THE_Theta).*sin(THE_Theta_pend))./6.0-(Ly_pend.^2.*THE_Psi_pend_D.*m_pend.*cos(THE_Psi).*cos(THE_Psi_pend).^2.*sin(THE_Theta).*sin(THE_Theta_pend))./6.0;
    et278 = Ly_pend.^2.*THE_Theta_pend_D.*m_pend.*cos(THE_Phi_pend).*cos(THE_Theta_pend).^2.*sin(THE_Psi).*sin(THE_Theta).*(-1.0./6.0)+(Lz_pend.^2.*THE_Theta_D.*m_pend.*cos(THE_Psi).*cos(THE_Phi_pend).^2.*sin(THE_Psi).*sin(THE_Theta))./3.0+(Lz_pend.^2.*THE_Theta_D.*m_pend.*cos(THE_Psi).*cos(THE_Psi_pend).^2.*sin(THE_Psi).*sin(THE_Theta))./3.0+Lz_pend.^2.*THE_Psi_pend_D.*m_pend.*cos(THE_Psi).*cos(THE_Phi_pend).^2.*sin(THE_Theta).*sin(THE_Theta_pend).*(2.0./3.0)+Lz_pend.^2.*THE_Psi_pend_D.*m_pend.*cos(THE_Psi).*cos(THE_Psi_pend).^2.*sin(THE_Theta).*sin(THE_Theta_pend).*(2.0./3.0)+(Lx_pend.^2.*THE_Phi_pend_D.*m_pend.*cos(THE_Psi).*cos(THE_Phi_pend).^2.*cos(THE_Theta_pend).^2.*sin(THE_Theta))./6.0+(Lx_pend.^2.*THE_Theta_pend_D.*m_pend.*cos(THE_Psi).^2.*cos(THE_Theta).*cos(THE_Theta_pend).^2.*sin(THE_Phi_pend))./3.0-(Ly_pend.^2.*THE_Phi_pend_D.*m_pend.*cos(THE_Psi).*cos(THE_Phi_pend).^2.*cos(THE_Psi_pend).^2.*sin(THE_Theta))./3.0-(Ly_pend.^2.*THE_Phi_pend_D.*m_pend.*cos(THE_Psi).*cos(THE_Phi_pend).^2.*cos(THE_Theta_pend).^2.*sin(THE_Theta))./6.0;
    et279 = Ly_pend.^2.*THE_Phi_pend_D.*m_pend.*cos(THE_Psi).*cos(THE_Psi_pend).^2.*cos(THE_Theta_pend).^2.*sin(THE_Theta).*(-1.0./6.0)-(Ly_pend.^2.*THE_Theta_pend_D.*m_pend.*cos(THE_Psi).^2.*cos(THE_Theta).*cos(THE_Psi_pend).^2.*sin(THE_Phi_pend))./6.0-(Ly_pend.^2.*THE_Theta_pend_D.*m_pend.*cos(THE_Psi).^2.*cos(THE_Theta).*cos(THE_Theta_pend).^2.*sin(THE_Phi_pend))./3.0-(Ly_pend.^2.*THE_Theta_pend_D.*m_pend.*cos(THE_Theta).*cos(THE_Psi_pend).^2.*cos(THE_Theta_pend).^2.*sin(THE_Phi_pend))./6.0+Lz_pend.^2.*THE_Phi_pend_D.*m_pend.*cos(THE_Psi).*cos(THE_Phi_pend).^2.*cos(THE_Psi_pend).^2.*sin(THE_Theta).*(4.0./3.0)+Lz_pend.^2.*THE_Phi_pend_D.*m_pend.*cos(THE_Psi).*cos(THE_Psi_pend).^2.*cos(THE_Theta_pend).^2.*sin(THE_Theta).*(2.0./3.0)+Lz_pend.^2.*THE_Theta_pend_D.*m_pend.*cos(THE_Psi).^2.*cos(THE_Theta).*cos(THE_Psi_pend).^2.*sin(THE_Phi_pend).*(2.0./3.0)+Lz_pend.^2.*THE_Theta_pend_D.*m_pend.*cos(THE_Theta).*cos(THE_Psi_pend).^2.*cos(THE_Theta_pend).^2.*sin(THE_Phi_pend).*(2.0./3.0)-(Lx_pend.^2.*THE_Phi_pend_D.*m_pend.*cos(THE_Theta).*cos(THE_Phi_pend).*cos(THE_Theta_pend).*sin(THE_Theta_pend))./6.0;
    et280 = (Ly_pend.^2.*THE_Theta_D.*m_pend.*cos(THE_Psi).*cos(THE_Theta).*cos(THE_Phi_pend).*sin(THE_Phi_pend))./1.2e+1+(Ly_pend.^2.*THE_Phi_pend_D.*m_pend.*cos(THE_Theta).*cos(THE_Phi_pend).*cos(THE_Theta_pend).*sin(THE_Theta_pend))./6.0-(Lz_pend.^2.*THE_Theta_D.*m_pend.*cos(THE_Psi).*cos(THE_Theta).*cos(THE_Phi_pend).*sin(THE_Phi_pend))./3.0+(Lx_pend.^2.*THE_Psi_D.*m_pend.*cos(THE_Psi).^2.*cos(THE_Theta).*cos(THE_Phi_pend).^2.*cos(THE_Theta_pend).^2)./6.0-(Ly_pend.^2.*THE_Psi_D.*m_pend.*cos(THE_Psi).^2.*cos(THE_Theta).*cos(THE_Phi_pend).^2.*cos(THE_Psi_pend).^2)./3.0-(Ly_pend.^2.*THE_Psi_D.*m_pend.*cos(THE_Psi).^2.*cos(THE_Theta).*cos(THE_Phi_pend).^2.*cos(THE_Theta_pend).^2)./6.0-(Ly_pend.^2.*THE_Psi_D.*m_pend.*cos(THE_Psi).^2.*cos(THE_Theta).*cos(THE_Psi_pend).^2.*cos(THE_Theta_pend).^2)./3.0+Lz_pend.^2.*THE_Psi_D.*m_pend.*cos(THE_Psi).^2.*cos(THE_Theta).*cos(THE_Phi_pend).^2.*cos(THE_Psi_pend).^2.*(4.0./3.0)+Lz_pend.^2.*THE_Psi_D.*m_pend.*cos(THE_Psi).^2.*cos(THE_Theta).*cos(THE_Psi_pend).^2.*cos(THE_Theta_pend).^2.*(4.0./3.0);
    et281 = (Lx_pend.^2.*THE_Theta_D.*m_pend.*cos(THE_Theta_pend).*sin(THE_Theta).*sin(THE_Phi_pend).*sin(THE_Theta_pend))./1.2e+1-(Ly_pend.^2.*THE_Psi_pend_D.*m_pend.*cos(THE_Theta_pend).*sin(THE_Psi).*sin(THE_Theta).*sin(THE_Phi_pend))./6.0-(Ly_pend.^2.*THE_Theta_D.*m_pend.*cos(THE_Theta_pend).*sin(THE_Theta).*sin(THE_Phi_pend).*sin(THE_Theta_pend))./1.2e+1-Lz_pend.*THE_Psi_D.*Tv_Z_pend.*m_pend.*cos(THE_Theta).*cos(THE_Psi_pend).*cos(THE_Theta_pend).*2.0-Lz_pend.*THE_Psi_pend_D.*Tv_Z_pend.*m_pend.*cos(THE_Theta).*cos(THE_Phi_pend).*cos(THE_Psi_pend)+Lz_pend.*THE_Psi_D.*Tv_Z_pend.*m_pend.*cos(THE_Psi).^2.*cos(THE_Theta).*cos(THE_Psi_pend).*cos(THE_Theta_pend).*2.0+Lz_pend.*THE_Psi_pend_D.*Tv_Z_pend.*m_pend.*cos(THE_Psi).^2.*cos(THE_Theta).*cos(THE_Phi_pend).*cos(THE_Psi_pend)-Lz_pend.*THE_Theta_D.*Tv_Z_pend.*m_pend.*cos(THE_Psi).^2.*cos(THE_Phi_pend).*sin(THE_Theta).*sin(THE_Psi_pend)-Lz_pend.*THE_Phi_pend_D.*Tv_Z_pend.*m_pend.*cos(THE_Psi).^2.*cos(THE_Theta).*sin(THE_Phi_pend).*sin(THE_Psi_pend)-(Ly_pend.^2.*THE_Psi_pend_D.*m_pend.*cos(THE_Psi).^2.*cos(THE_Theta).*cos(THE_Phi_pend).*cos(THE_Psi_pend).^2.*cos(THE_Theta_pend))./3.0+Lz_pend.^2.*THE_Psi_pend_D.*m_pend.*cos(THE_Psi).^2.*cos(THE_Theta).*cos(THE_Phi_pend).*cos(THE_Psi_pend).^2.*cos(THE_Theta_pend).*(4.0./3.0);
    et282 = Lx_pend.^2.*THE_Theta_D.*m_pend.*cos(THE_Psi).*cos(THE_Phi_pend).^2.*cos(THE_Theta_pend).^2.*sin(THE_Psi).*sin(THE_Theta).*(-1.0./1.2e+1)+(Ly_pend.^2.*THE_Theta_D.*m_pend.*cos(THE_Psi).*cos(THE_Phi_pend).^2.*cos(THE_Psi_pend).^2.*sin(THE_Psi).*sin(THE_Theta))./6.0+(Ly_pend.^2.*THE_Theta_D.*m_pend.*cos(THE_Psi).*cos(THE_Phi_pend).^2.*cos(THE_Theta_pend).^2.*sin(THE_Psi).*sin(THE_Theta))./1.2e+1+(Ly_pend.^2.*THE_Theta_D.*m_pend.*cos(THE_Psi).*cos(THE_Psi_pend).^2.*cos(THE_Theta_pend).^2.*sin(THE_Psi).*sin(THE_Theta))./6.0+(Ly_pend.^2.*THE_Psi_pend_D.*m_pend.*cos(THE_Psi).*cos(THE_Phi_pend).^2.*cos(THE_Psi_pend).^2.*sin(THE_Theta).*sin(THE_Theta_pend))./3.0+(Ly_pend.^2.*THE_Theta_pend_D.*m_pend.*cos(THE_Phi_pend).*cos(THE_Psi_pend).^2.*cos(THE_Theta_pend).^2.*sin(THE_Psi).*sin(THE_Theta))./6.0-Lz_pend.^2.*THE_Theta_D.*m_pend.*cos(THE_Psi).*cos(THE_Phi_pend).^2.*cos(THE_Psi_pend).^2.*sin(THE_Psi).*sin(THE_Theta).*(2.0./3.0)-Lz_pend.^2.*THE_Theta_D.*m_pend.*cos(THE_Psi).*cos(THE_Psi_pend).^2.*cos(THE_Theta_pend).^2.*sin(THE_Psi).*sin(THE_Theta).*(2.0./3.0);
    et283 = Lz_pend.^2.*THE_Psi_pend_D.*m_pend.*cos(THE_Psi).*cos(THE_Phi_pend).^2.*cos(THE_Psi_pend).^2.*sin(THE_Theta).*sin(THE_Theta_pend).*(-4.0./3.0)-Lz_pend.^2.*THE_Theta_pend_D.*m_pend.*cos(THE_Phi_pend).*cos(THE_Psi_pend).^2.*cos(THE_Theta_pend).^2.*sin(THE_Psi).*sin(THE_Theta).*(2.0./3.0)+(Lx_pend.^2.*THE_Theta_D.*m_pend.*cos(THE_Theta).*cos(THE_Phi_pend).*cos(THE_Theta_pend).*sin(THE_Psi).*sin(THE_Theta_pend))./1.2e+1+(Lx_pend.^2.*THE_Theta_pend_D.*m_pend.*cos(THE_Psi).*cos(THE_Theta).*cos(THE_Theta_pend).*sin(THE_Psi).*sin(THE_Theta_pend))./3.0-(Ly_pend.^2.*THE_Phi_pend_D.*m_pend.*cos(THE_Psi).*cos(THE_Theta).*cos(THE_Phi_pend).*sin(THE_Psi).*sin(THE_Phi_pend))./6.0-(Ly_pend.^2.*THE_Psi_pend_D.*m_pend.*cos(THE_Psi).*cos(THE_Theta).*cos(THE_Psi_pend).*sin(THE_Psi).*sin(THE_Psi_pend))./6.0-(Ly_pend.^2.*THE_Theta_D.*m_pend.*cos(THE_Psi).*cos(THE_Theta).*cos(THE_Psi_pend).*sin(THE_Psi_pend).*sin(THE_Theta_pend))./1.2e+1-(Ly_pend.^2.*THE_Theta_D.*m_pend.*cos(THE_Theta).*cos(THE_Phi_pend).*cos(THE_Theta_pend).*sin(THE_Psi).*sin(THE_Theta_pend))./1.2e+1-(Ly_pend.^2.*THE_Theta_pend_D.*m_pend.*cos(THE_Psi).*cos(THE_Theta).*cos(THE_Theta_pend).*sin(THE_Psi).*sin(THE_Theta_pend))./3.0;
    et284 = Ly_pend.^2.*THE_Theta_D.*m_pend.*cos(THE_Phi_pend).*cos(THE_Psi_pend).*cos(THE_Theta_pend).*sin(THE_Theta).*sin(THE_Psi_pend).*(-1.0./1.2e+1)-(Ly_pend.^2.*THE_Phi_pend_D.*m_pend.*cos(THE_Theta).*cos(THE_Psi_pend).*cos(THE_Theta_pend).*sin(THE_Phi_pend).*sin(THE_Psi_pend))./6.0+Lz_pend.^2.*THE_Phi_pend_D.*m_pend.*cos(THE_Psi).*cos(THE_Theta).*cos(THE_Phi_pend).*sin(THE_Psi).*sin(THE_Phi_pend).*(2.0./3.0)+Lz_pend.^2.*THE_Psi_pend_D.*m_pend.*cos(THE_Psi).*cos(THE_Theta).*cos(THE_Psi_pend).*sin(THE_Psi).*sin(THE_Psi_pend).*(2.0./3.0)+(Lz_pend.^2.*THE_Theta_D.*m_pend.*cos(THE_Psi).*cos(THE_Theta).*cos(THE_Psi_pend).*sin(THE_Psi_pend).*sin(THE_Theta_pend))./3.0+(Lz_pend.^2.*THE_Theta_D.*m_pend.*cos(THE_Phi_pend).*cos(THE_Psi_pend).*cos(THE_Theta_pend).*sin(THE_Theta).*sin(THE_Psi_pend))./3.0+Lz_pend.^2.*THE_Phi_pend_D.*m_pend.*cos(THE_Theta).*cos(THE_Psi_pend).*cos(THE_Theta_pend).*sin(THE_Phi_pend).*sin(THE_Psi_pend).*(2.0./3.0)+(Ly_pend.^2.*THE_Phi_pend_D.*m_pend.*cos(THE_Psi).*cos(THE_Phi_pend).^2.*cos(THE_Psi_pend).^2.*cos(THE_Theta_pend).^2.*sin(THE_Theta))./6.0+(Ly_pend.^2.*THE_Theta_pend_D.*m_pend.*cos(THE_Psi).^2.*cos(THE_Theta).*cos(THE_Psi_pend).^2.*cos(THE_Theta_pend).^2.*sin(THE_Phi_pend))./3.0;
    et285 = Lz_pend.^2.*THE_Phi_pend_D.*m_pend.*cos(THE_Psi).*cos(THE_Phi_pend).^2.*cos(THE_Psi_pend).^2.*cos(THE_Theta_pend).^2.*sin(THE_Theta).*(-2.0./3.0)-Lz_pend.^2.*THE_Theta_pend_D.*m_pend.*cos(THE_Psi).^2.*cos(THE_Theta).*cos(THE_Psi_pend).^2.*cos(THE_Theta_pend).^2.*sin(THE_Phi_pend).*(4.0./3.0)-(Lx_pend.^2.*THE_Phi_pend_D.*m_pend.*cos(THE_Theta_pend).*sin(THE_Psi).*sin(THE_Theta).*sin(THE_Phi_pend).*sin(THE_Theta_pend))./6.0+(Ly_pend.^2.*THE_Phi_pend_D.*m_pend.*cos(THE_Theta_pend).*sin(THE_Psi).*sin(THE_Theta).*sin(THE_Phi_pend).*sin(THE_Theta_pend))./6.0+Lz_pend.*THE_Phi_pend_D.*Tv_Z_pend.*m_pend.*cos(THE_Theta).*cos(THE_Phi_pend).*cos(THE_Psi_pend).*sin(THE_Theta_pend)+Lz_pend.*THE_Theta_pend_D.*Tv_Z_pend.*m_pend.*cos(THE_Theta).*cos(THE_Psi_pend).*cos(THE_Theta_pend).*sin(THE_Phi_pend)-(Lz_pend.*THE_Theta_D.*Tv_Z_pend.*m_pend.*cos(THE_Theta).*sin(THE_Psi).*sin(THE_Phi_pend).*sin(THE_Psi_pend))./2.0-Lz_pend.*THE_Phi_pend_D.*Tv_Z_pend.*m_pend.*cos(THE_Phi_pend).*sin(THE_Psi).*sin(THE_Theta).*sin(THE_Psi_pend)-Lz_pend.*THE_Psi_pend_D.*Tv_Z_pend.*m_pend.*cos(THE_Psi_pend).*sin(THE_Psi).*sin(THE_Theta).*sin(THE_Phi_pend)-(Lz_pend.*THE_Theta_D.*Tv_Z_pend.*m_pend.*cos(THE_Psi_pend).*sin(THE_Theta).*sin(THE_Phi_pend).*sin(THE_Theta_pend))./2.0-Lz_pend.*THE_Psi_pend_D.*Tv_Z_pend.*m_pend.*cos(THE_Theta).*sin(THE_Phi_pend).*sin(THE_Psi_pend).*sin(THE_Theta_pend);
    et286 = (Lx_pend.^2.*THE_Theta_D.*m_pend.*cos(THE_Psi).*cos(THE_Theta).*cos(THE_Phi_pend).*cos(THE_Theta_pend).^2.*sin(THE_Phi_pend))./1.2e+1+(Lx_pend.^2.*THE_Phi_pend_D.*m_pend.*cos(THE_Psi).^2.*cos(THE_Theta).*cos(THE_Phi_pend).*cos(THE_Theta_pend).*sin(THE_Theta_pend))./6.0-(Ly_pend.^2.*THE_Theta_D.*m_pend.*cos(THE_Psi).*cos(THE_Theta).*cos(THE_Phi_pend).*cos(THE_Psi_pend).^2.*sin(THE_Phi_pend))./6.0-(Ly_pend.^2.*THE_Theta_D.*m_pend.*cos(THE_Psi).*cos(THE_Theta).*cos(THE_Phi_pend).*cos(THE_Theta_pend).^2.*sin(THE_Phi_pend))./1.2e+1-(Ly_pend.^2.*THE_Phi_pend_D.*m_pend.*cos(THE_Psi).^2.*cos(THE_Theta).*cos(THE_Phi_pend).*cos(THE_Theta_pend).*sin(THE_Theta_pend))./6.0-(Ly_pend.^2.*THE_Phi_pend_D.*m_pend.*cos(THE_Theta).*cos(THE_Phi_pend).*cos(THE_Psi_pend).^2.*cos(THE_Theta_pend).*sin(THE_Theta_pend))./6.0+Lz_pend.^2.*THE_Theta_D.*m_pend.*cos(THE_Psi).*cos(THE_Theta).*cos(THE_Phi_pend).*cos(THE_Psi_pend).^2.*sin(THE_Phi_pend).*(2.0./3.0)+Lz_pend.^2.*THE_Phi_pend_D.*m_pend.*cos(THE_Theta).*cos(THE_Phi_pend).*cos(THE_Psi_pend).^2.*cos(THE_Theta_pend).*sin(THE_Theta_pend).*(2.0./3.0);
    et287 = (Ly_pend.^2.*THE_Psi_D.*m_pend.*cos(THE_Psi).^2.*cos(THE_Theta).*cos(THE_Phi_pend).^2.*cos(THE_Psi_pend).^2.*cos(THE_Theta_pend).^2)./6.0-Lz_pend.^2.*THE_Psi_D.*m_pend.*cos(THE_Psi).^2.*cos(THE_Theta).*cos(THE_Phi_pend).^2.*cos(THE_Psi_pend).^2.*cos(THE_Theta_pend).^2.*(2.0./3.0)-(Lx_pend.^2.*THE_Theta_D.*m_pend.*cos(THE_Psi).^2.*cos(THE_Theta_pend).*sin(THE_Theta).*sin(THE_Phi_pend).*sin(THE_Theta_pend))./6.0+(Ly_pend.^2.*THE_Theta_D.*m_pend.*cos(THE_Psi).^2.*cos(THE_Theta_pend).*sin(THE_Theta).*sin(THE_Phi_pend).*sin(THE_Theta_pend))./6.0+(Ly_pend.^2.*THE_Psi_pend_D.*m_pend.*cos(THE_Psi_pend).^2.*cos(THE_Theta_pend).*sin(THE_Psi).*sin(THE_Theta).*sin(THE_Phi_pend))./6.0+(Ly_pend.^2.*THE_Theta_D.*m_pend.*cos(THE_Psi_pend).^2.*cos(THE_Theta_pend).*sin(THE_Theta).*sin(THE_Phi_pend).*sin(THE_Theta_pend))./1.2e+1-Lz_pend.^2.*THE_Psi_pend_D.*m_pend.*cos(THE_Psi_pend).^2.*cos(THE_Theta_pend).*sin(THE_Psi).*sin(THE_Theta).*sin(THE_Phi_pend).*(2.0./3.0)-(Lz_pend.^2.*THE_Theta_D.*m_pend.*cos(THE_Psi_pend).^2.*cos(THE_Theta_pend).*sin(THE_Theta).*sin(THE_Phi_pend).*sin(THE_Theta_pend))./3.0;
    et288 = Ly_pend.^2.*THE_Theta_D.*m_pend.*cos(THE_Psi).^2.*cos(THE_Psi_pend).^2.*cos(THE_Theta_pend).*sin(THE_Theta).*sin(THE_Phi_pend).*sin(THE_Theta_pend).*(-1.0./6.0)+Lz_pend.^2.*THE_Theta_D.*m_pend.*cos(THE_Psi).^2.*cos(THE_Psi_pend).^2.*cos(THE_Theta_pend).*sin(THE_Theta).*sin(THE_Phi_pend).*sin(THE_Theta_pend).*(2.0./3.0)-(Lx_pend.^2.*THE_Psi_D.*m_pend.*cos(THE_Psi).*cos(THE_Theta).*cos(THE_Theta_pend).*sin(THE_Psi).*sin(THE_Phi_pend).*sin(THE_Theta_pend))./3.0-(Lx_pend.^2.*THE_Theta_pend_D.*m_pend.*cos(THE_Psi).*cos(THE_Phi_pend).*cos(THE_Theta_pend).*sin(THE_Theta).*sin(THE_Phi_pend).*sin(THE_Theta_pend))./6.0+(Ly_pend.^2.*THE_Psi_D.*m_pend.*cos(THE_Psi).*cos(THE_Theta).*cos(THE_Theta_pend).*sin(THE_Psi).*sin(THE_Phi_pend).*sin(THE_Theta_pend))./3.0+(Ly_pend.^2.*THE_Psi_pend_D.*m_pend.*cos(THE_Psi).*cos(THE_Theta).*cos(THE_Phi_pend).*sin(THE_Psi).*sin(THE_Phi_pend).*sin(THE_Theta_pend))./6.0+(Ly_pend.^2.*THE_Phi_pend_D.*m_pend.*cos(THE_Psi).*cos(THE_Theta).*cos(THE_Psi_pend).*sin(THE_Psi).*sin(THE_Psi_pend).*sin(THE_Theta_pend))./6.0+(Ly_pend.^2.*THE_Theta_D.*m_pend.*cos(THE_Theta).*cos(THE_Psi_pend).*cos(THE_Theta_pend).*sin(THE_Psi).*sin(THE_Phi_pend).*sin(THE_Psi_pend))./1.2e+1;
    et289 = (Ly_pend.^2.*THE_Psi_pend_D.*m_pend.*cos(THE_Psi).*cos(THE_Phi_pend).*cos(THE_Psi_pend).*sin(THE_Theta).*sin(THE_Phi_pend).*sin(THE_Psi_pend))./3.0+(Ly_pend.^2.*THE_Phi_pend_D.*m_pend.*cos(THE_Phi_pend).*cos(THE_Psi_pend).*cos(THE_Theta_pend).*sin(THE_Psi).*sin(THE_Theta).*sin(THE_Psi_pend))./6.0+(Ly_pend.^2.*THE_Theta_pend_D.*m_pend.*cos(THE_Psi).*cos(THE_Phi_pend).*cos(THE_Theta_pend).*sin(THE_Theta).*sin(THE_Phi_pend).*sin(THE_Theta_pend))./6.0+(Ly_pend.^2.*THE_Psi_pend_D.*m_pend.*cos(THE_Theta).*cos(THE_Psi_pend).*cos(THE_Theta_pend).*sin(THE_Phi_pend).*sin(THE_Psi_pend).*sin(THE_Theta_pend))./6.0-Lz_pend.^2.*THE_Psi_pend_D.*m_pend.*cos(THE_Psi).*cos(THE_Theta).*cos(THE_Phi_pend).*sin(THE_Psi).*sin(THE_Phi_pend).*sin(THE_Theta_pend).*(2.0./3.0)-Lz_pend.^2.*THE_Phi_pend_D.*m_pend.*cos(THE_Psi).*cos(THE_Theta).*cos(THE_Psi_pend).*sin(THE_Psi).*sin(THE_Psi_pend).*sin(THE_Theta_pend).*(2.0./3.0)-(Lz_pend.^2.*THE_Theta_D.*m_pend.*cos(THE_Theta).*cos(THE_Psi_pend).*cos(THE_Theta_pend).*sin(THE_Psi).*sin(THE_Phi_pend).*sin(THE_Psi_pend))./3.0-Lz_pend.^2.*THE_Psi_pend_D.*m_pend.*cos(THE_Psi).*cos(THE_Phi_pend).*cos(THE_Psi_pend).*sin(THE_Theta).*sin(THE_Phi_pend).*sin(THE_Psi_pend).*(4.0./3.0)-Lz_pend.^2.*THE_Phi_pend_D.*m_pend.*cos(THE_Phi_pend).*cos(THE_Psi_pend).*cos(THE_Theta_pend).*sin(THE_Psi).*sin(THE_Theta).*sin(THE_Psi_pend).*(2.0./3.0);
    et290 = Lz_pend.^2.*THE_Psi_pend_D.*m_pend.*cos(THE_Theta).*cos(THE_Psi_pend).*cos(THE_Theta_pend).*sin(THE_Phi_pend).*sin(THE_Psi_pend).*sin(THE_Theta_pend).*(-2.0./3.0)-(Ly_pend.^2.*THE_Theta_D.*m_pend.*cos(THE_Psi).*cos(THE_Phi_pend).^2.*cos(THE_Psi_pend).^2.*cos(THE_Theta_pend).^2.*sin(THE_Psi).*sin(THE_Theta))./1.2e+1+(Lz_pend.^2.*THE_Theta_D.*m_pend.*cos(THE_Psi).*cos(THE_Phi_pend).^2.*cos(THE_Psi_pend).^2.*cos(THE_Theta_pend).^2.*sin(THE_Psi).*sin(THE_Theta))./3.0-Lz_pend.*THE_Psi_D.*Tv_Z_pend.*m_pend.*cos(THE_Psi).*cos(THE_Theta).*cos(THE_Phi_pend).*sin(THE_Psi).*sin(THE_Psi_pend).*2.0-Lz_pend.*THE_Theta_D.*Tv_Z_pend.*m_pend.*cos(THE_Psi).*cos(THE_Psi_pend).*cos(THE_Theta_pend).*sin(THE_Psi).*sin(THE_Theta)-Lz_pend.*THE_Psi_pend_D.*Tv_Z_pend.*m_pend.*cos(THE_Psi).*cos(THE_Theta).*cos(THE_Theta_pend).*sin(THE_Psi).*sin(THE_Psi_pend)-(Lz_pend.*THE_Theta_D.*Tv_Z_pend.*m_pend.*cos(THE_Theta).*cos(THE_Phi_pend).*cos(THE_Psi_pend).*sin(THE_Psi).*sin(THE_Theta_pend))./2.0-Lz_pend.*THE_Theta_pend_D.*Tv_Z_pend.*m_pend.*cos(THE_Psi).*cos(THE_Theta).*cos(THE_Psi_pend).*sin(THE_Psi).*sin(THE_Theta_pend)-Lz_pend.*THE_Theta_pend_D.*Tv_Z_pend.*m_pend.*cos(THE_Phi_pend).*cos(THE_Psi_pend).*cos(THE_Theta_pend).*sin(THE_Psi).*sin(THE_Theta)+Lz_pend.*THE_Phi_pend_D.*Tv_Z_pend.*m_pend.*cos(THE_Psi_pend).*sin(THE_Psi).*sin(THE_Theta).*sin(THE_Phi_pend).*sin(THE_Theta_pend);
    et291 = Lz_pend.*THE_Psi_pend_D.*Tv_Z_pend.*m_pend.*cos(THE_Phi_pend).*sin(THE_Psi).*sin(THE_Theta).*sin(THE_Psi_pend).*sin(THE_Theta_pend)-(Lx_pend.^2.*THE_Phi_pend_D.*m_pend.*cos(THE_Psi).*cos(THE_Theta).*cos(THE_Phi_pend).*cos(THE_Theta_pend).^2.*sin(THE_Psi).*sin(THE_Phi_pend))./6.0-(Lx_pend.^2.*THE_Theta_pend_D.*m_pend.*cos(THE_Psi).*cos(THE_Theta).*cos(THE_Phi_pend).^2.*cos(THE_Theta_pend).*sin(THE_Psi).*sin(THE_Theta_pend))./6.0+(Ly_pend.^2.*THE_Phi_pend_D.*m_pend.*cos(THE_Psi).*cos(THE_Theta).*cos(THE_Phi_pend).*cos(THE_Psi_pend).^2.*sin(THE_Psi).*sin(THE_Phi_pend))./3.0+(Ly_pend.^2.*THE_Psi_pend_D.*m_pend.*cos(THE_Psi).*cos(THE_Theta).*cos(THE_Phi_pend).^2.*cos(THE_Psi_pend).*sin(THE_Psi).*sin(THE_Psi_pend))./3.0+(Ly_pend.^2.*THE_Phi_pend_D.*m_pend.*cos(THE_Psi).*cos(THE_Theta).*cos(THE_Phi_pend).*cos(THE_Theta_pend).^2.*sin(THE_Psi).*sin(THE_Phi_pend))./6.0+(Ly_pend.^2.*THE_Psi_pend_D.*m_pend.*cos(THE_Psi).*cos(THE_Theta).*cos(THE_Psi_pend).*cos(THE_Theta_pend).^2.*sin(THE_Psi).*sin(THE_Psi_pend))./3.0+(Ly_pend.^2.*THE_Theta_D.*m_pend.*cos(THE_Psi).*cos(THE_Theta).*cos(THE_Phi_pend).^2.*cos(THE_Psi_pend).*sin(THE_Psi_pend).*sin(THE_Theta_pend))./6.0;
    et292 = (Ly_pend.^2.*THE_Theta_D.*m_pend.*cos(THE_Psi).^2.*cos(THE_Phi_pend).*cos(THE_Psi_pend).*cos(THE_Theta_pend).*sin(THE_Theta).*sin(THE_Psi_pend))./6.0+(Ly_pend.^2.*THE_Theta_D.*m_pend.*cos(THE_Theta).*cos(THE_Phi_pend).*cos(THE_Psi_pend).^2.*cos(THE_Theta_pend).*sin(THE_Psi).*sin(THE_Theta_pend))./1.2e+1+(Ly_pend.^2.*THE_Theta_pend_D.*m_pend.*cos(THE_Psi).*cos(THE_Theta).*cos(THE_Phi_pend).^2.*cos(THE_Theta_pend).*sin(THE_Psi).*sin(THE_Theta_pend))./6.0+(Ly_pend.^2.*THE_Theta_pend_D.*m_pend.*cos(THE_Psi).*cos(THE_Theta).*cos(THE_Psi_pend).^2.*cos(THE_Theta_pend).*sin(THE_Psi).*sin(THE_Theta_pend))./3.0+(Ly_pend.^2.*THE_Phi_pend_D.*m_pend.*cos(THE_Psi).^2.*cos(THE_Theta).*cos(THE_Psi_pend).*cos(THE_Theta_pend).*sin(THE_Phi_pend).*sin(THE_Psi_pend))./6.0+(Ly_pend.^2.*THE_Theta_pend_D.*m_pend.*cos(THE_Psi).*cos(THE_Phi_pend).^2.*cos(THE_Psi_pend).*cos(THE_Theta_pend).*sin(THE_Theta).*sin(THE_Psi_pend))./6.0+(Ly_pend.^2.*THE_Theta_pend_D.*m_pend.*cos(THE_Psi).^2.*cos(THE_Theta).*cos(THE_Phi_pend).*cos(THE_Psi_pend).*sin(THE_Psi_pend).*sin(THE_Theta_pend))./6.0-Lz_pend.^2.*THE_Phi_pend_D.*m_pend.*cos(THE_Psi).*cos(THE_Theta).*cos(THE_Phi_pend).*cos(THE_Psi_pend).^2.*sin(THE_Psi).*sin(THE_Phi_pend).*(4.0./3.0);
    et293 = Lz_pend.^2.*THE_Psi_pend_D.*m_pend.*cos(THE_Psi).*cos(THE_Theta).*cos(THE_Phi_pend).^2.*cos(THE_Psi_pend).*sin(THE_Psi).*sin(THE_Psi_pend).*(-4.0./3.0)-Lz_pend.^2.*THE_Psi_pend_D.*m_pend.*cos(THE_Psi).*cos(THE_Theta).*cos(THE_Psi_pend).*cos(THE_Theta_pend).^2.*sin(THE_Psi).*sin(THE_Psi_pend).*(4.0./3.0)-Lz_pend.^2.*THE_Theta_D.*m_pend.*cos(THE_Psi).*cos(THE_Theta).*cos(THE_Phi_pend).^2.*cos(THE_Psi_pend).*sin(THE_Psi_pend).*sin(THE_Theta_pend).*(2.0./3.0)-Lz_pend.^2.*THE_Theta_D.*m_pend.*cos(THE_Psi).^2.*cos(THE_Phi_pend).*cos(THE_Psi_pend).*cos(THE_Theta_pend).*sin(THE_Theta).*sin(THE_Psi_pend).*(2.0./3.0)-(Lz_pend.^2.*THE_Theta_D.*m_pend.*cos(THE_Theta).*cos(THE_Phi_pend).*cos(THE_Psi_pend).^2.*cos(THE_Theta_pend).*sin(THE_Psi).*sin(THE_Theta_pend))./3.0-Lz_pend.^2.*THE_Theta_pend_D.*m_pend.*cos(THE_Psi).*cos(THE_Theta).*cos(THE_Psi_pend).^2.*cos(THE_Theta_pend).*sin(THE_Psi).*sin(THE_Theta_pend).*(4.0./3.0)-Lz_pend.^2.*THE_Phi_pend_D.*m_pend.*cos(THE_Psi).^2.*cos(THE_Theta).*cos(THE_Psi_pend).*cos(THE_Theta_pend).*sin(THE_Phi_pend).*sin(THE_Psi_pend).*(2.0./3.0)-Lz_pend.^2.*THE_Theta_pend_D.*m_pend.*cos(THE_Psi).*cos(THE_Phi_pend).^2.*cos(THE_Psi_pend).*cos(THE_Theta_pend).*sin(THE_Theta).*sin(THE_Psi_pend).*(2.0./3.0);
    et294 = Lz_pend.^2.*THE_Theta_pend_D.*m_pend.*cos(THE_Psi).^2.*cos(THE_Theta).*cos(THE_Phi_pend).*cos(THE_Psi_pend).*sin(THE_Psi_pend).*sin(THE_Theta_pend).*(-2.0./3.0)-(Ly_pend.^2.*THE_Phi_pend_D.*m_pend.*cos(THE_Psi_pend).^2.*cos(THE_Theta_pend).*sin(THE_Psi).*sin(THE_Theta).*sin(THE_Phi_pend).*sin(THE_Theta_pend))./6.0+Lz_pend.^2.*THE_Phi_pend_D.*m_pend.*cos(THE_Psi_pend).^2.*cos(THE_Theta_pend).*sin(THE_Psi).*sin(THE_Theta).*sin(THE_Phi_pend).*sin(THE_Theta_pend).*(2.0./3.0)-Lz_pend.*THE_Phi_pend_D.*Tv_Z_pend.*m_pend.*cos(THE_Psi).^2.*cos(THE_Theta).*cos(THE_Phi_pend).*cos(THE_Psi_pend).*sin(THE_Theta_pend)-Lz_pend.*THE_Theta_pend_D.*Tv_Z_pend.*m_pend.*cos(THE_Psi).^2.*cos(THE_Theta).*cos(THE_Psi_pend).*cos(THE_Theta_pend).*sin(THE_Phi_pend)+Lz_pend.*THE_Theta_D.*Tv_Z_pend.*m_pend.*cos(THE_Psi).^2.*cos(THE_Psi_pend).*sin(THE_Theta).*sin(THE_Phi_pend).*sin(THE_Theta_pend)+Lz_pend.*THE_Psi_pend_D.*Tv_Z_pend.*m_pend.*cos(THE_Psi).^2.*cos(THE_Theta).*sin(THE_Phi_pend).*sin(THE_Psi_pend).*sin(THE_Theta_pend)+(Ly_pend.^2.*THE_Theta_D.*m_pend.*cos(THE_Psi).*cos(THE_Theta).*cos(THE_Phi_pend).*cos(THE_Psi_pend).^2.*cos(THE_Theta_pend).^2.*sin(THE_Phi_pend))./1.2e+1+(Ly_pend.^2.*THE_Phi_pend_D.*m_pend.*cos(THE_Psi).^2.*cos(THE_Theta).*cos(THE_Phi_pend).*cos(THE_Psi_pend).^2.*cos(THE_Theta_pend).*sin(THE_Theta_pend))./6.0;
    et295 = Lz_pend.^2.*THE_Theta_D.*m_pend.*cos(THE_Psi).*cos(THE_Theta).*cos(THE_Phi_pend).*cos(THE_Psi_pend).^2.*cos(THE_Theta_pend).^2.*sin(THE_Phi_pend).*(-1.0./3.0)-Lz_pend.^2.*THE_Phi_pend_D.*m_pend.*cos(THE_Psi).^2.*cos(THE_Theta).*cos(THE_Phi_pend).*cos(THE_Psi_pend).^2.*cos(THE_Theta_pend).*sin(THE_Theta_pend).*(2.0./3.0)-(Ly_pend.^2.*THE_Phi_pend_D.*m_pend.*cos(THE_Psi).*cos(THE_Phi_pend).*cos(THE_Psi_pend).*sin(THE_Theta).*sin(THE_Phi_pend).*sin(THE_Psi_pend).*sin(THE_Theta_pend))./3.0-(Ly_pend.^2.*THE_Psi_pend_D.*m_pend.*cos(THE_Phi_pend).*cos(THE_Psi_pend).*cos(THE_Theta_pend).*sin(THE_Psi).*sin(THE_Theta).*sin(THE_Psi_pend).*sin(THE_Theta_pend))./6.0+Lz_pend.^2.*THE_Phi_pend_D.*m_pend.*cos(THE_Psi).*cos(THE_Phi_pend).*cos(THE_Psi_pend).*sin(THE_Theta).*sin(THE_Phi_pend).*sin(THE_Psi_pend).*sin(THE_Theta_pend).*(4.0./3.0)+Lz_pend.^2.*THE_Psi_pend_D.*m_pend.*cos(THE_Phi_pend).*cos(THE_Psi_pend).*cos(THE_Theta_pend).*sin(THE_Psi).*sin(THE_Theta).*sin(THE_Psi_pend).*sin(THE_Theta_pend).*(2.0./3.0)+Lz_pend.*THE_Psi_D.*Tv_Z_pend.*m_pend.*cos(THE_Psi).*cos(THE_Theta).*cos(THE_Psi_pend).*sin(THE_Psi).*sin(THE_Phi_pend).*sin(THE_Theta_pend).*2.0-(Ly_pend.^2.*THE_Psi_D.*m_pend.*cos(THE_Psi).*cos(THE_Theta).*cos(THE_Psi_pend).^2.*cos(THE_Theta_pend).*sin(THE_Psi).*sin(THE_Phi_pend).*sin(THE_Theta_pend))./3.0;
    et296 = Ly_pend.^2.*THE_Psi_D.*m_pend.*cos(THE_Psi).^2.*cos(THE_Theta).*cos(THE_Phi_pend).*cos(THE_Psi_pend).*sin(THE_Phi_pend).*sin(THE_Psi_pend).*sin(THE_Theta_pend).*(-1.0./3.0)-(Ly_pend.^2.*THE_Phi_pend_D.*m_pend.*cos(THE_Psi).*cos(THE_Theta).*cos(THE_Phi_pend).^2.*cos(THE_Psi_pend).*sin(THE_Psi).*sin(THE_Psi_pend).*sin(THE_Theta_pend))./3.0-(Ly_pend.^2.*THE_Psi_pend_D.*m_pend.*cos(THE_Psi).*cos(THE_Theta).*cos(THE_Phi_pend).*cos(THE_Psi_pend).^2.*sin(THE_Psi).*sin(THE_Phi_pend).*sin(THE_Theta_pend))./3.0-(Ly_pend.^2.*THE_Psi_pend_D.*m_pend.*cos(THE_Psi).*cos(THE_Phi_pend).*cos(THE_Psi_pend).*cos(THE_Theta_pend).^2.*sin(THE_Theta).*sin(THE_Phi_pend).*sin(THE_Psi_pend))./6.0-(Ly_pend.^2.*THE_Psi_pend_D.*m_pend.*cos(THE_Psi).^2.*cos(THE_Theta).*cos(THE_Psi_pend).*cos(THE_Theta_pend).*sin(THE_Phi_pend).*sin(THE_Psi_pend).*sin(THE_Theta_pend))./3.0-(Ly_pend.^2.*THE_Theta_pend_D.*m_pend.*cos(THE_Psi).*cos(THE_Phi_pend).*cos(THE_Psi_pend).^2.*cos(THE_Theta_pend).*sin(THE_Theta).*sin(THE_Phi_pend).*sin(THE_Theta_pend))./6.0+Lz_pend.^2.*THE_Psi_D.*m_pend.*cos(THE_Psi).*cos(THE_Theta).*cos(THE_Psi_pend).^2.*cos(THE_Theta_pend).*sin(THE_Psi).*sin(THE_Phi_pend).*sin(THE_Theta_pend).*(4.0./3.0);
    et297 = Lz_pend.^2.*THE_Psi_D.*m_pend.*cos(THE_Psi).^2.*cos(THE_Theta).*cos(THE_Phi_pend).*cos(THE_Psi_pend).*sin(THE_Phi_pend).*sin(THE_Psi_pend).*sin(THE_Theta_pend).*(4.0./3.0)+Lz_pend.^2.*THE_Phi_pend_D.*m_pend.*cos(THE_Psi).*cos(THE_Theta).*cos(THE_Phi_pend).^2.*cos(THE_Psi_pend).*sin(THE_Psi).*sin(THE_Psi_pend).*sin(THE_Theta_pend).*(4.0./3.0)+Lz_pend.^2.*THE_Psi_pend_D.*m_pend.*cos(THE_Psi).*cos(THE_Theta).*cos(THE_Phi_pend).*cos(THE_Psi_pend).^2.*sin(THE_Psi).*sin(THE_Phi_pend).*sin(THE_Theta_pend).*(4.0./3.0)+Lz_pend.^2.*THE_Psi_pend_D.*m_pend.*cos(THE_Psi).*cos(THE_Phi_pend).*cos(THE_Psi_pend).*cos(THE_Theta_pend).^2.*sin(THE_Theta).*sin(THE_Phi_pend).*sin(THE_Psi_pend).*(2.0./3.0)+Lz_pend.^2.*THE_Psi_pend_D.*m_pend.*cos(THE_Psi).^2.*cos(THE_Theta).*cos(THE_Psi_pend).*cos(THE_Theta_pend).*sin(THE_Phi_pend).*sin(THE_Psi_pend).*sin(THE_Theta_pend).*(4.0./3.0)+Lz_pend.^2.*THE_Theta_pend_D.*m_pend.*cos(THE_Psi).*cos(THE_Phi_pend).*cos(THE_Psi_pend).^2.*cos(THE_Theta_pend).*sin(THE_Theta).*sin(THE_Phi_pend).*sin(THE_Theta_pend).*(2.0./3.0)-(Ly_pend.^2.*THE_Phi_pend_D.*m_pend.*cos(THE_Psi).*cos(THE_Theta).*cos(THE_Phi_pend).*cos(THE_Psi_pend).^2.*cos(THE_Theta_pend).^2.*sin(THE_Psi).*sin(THE_Phi_pend))./6.0;
    et298 = Ly_pend.^2.*THE_Psi_pend_D.*m_pend.*cos(THE_Psi).*cos(THE_Theta).*cos(THE_Phi_pend).^2.*cos(THE_Psi_pend).*cos(THE_Theta_pend).^2.*sin(THE_Psi).*sin(THE_Psi_pend).*(-1.0./6.0)-(Ly_pend.^2.*THE_Theta_pend_D.*m_pend.*cos(THE_Psi).*cos(THE_Theta).*cos(THE_Phi_pend).^2.*cos(THE_Psi_pend).^2.*cos(THE_Theta_pend).*sin(THE_Psi).*sin(THE_Theta_pend))./6.0+Lz_pend.^2.*THE_Phi_pend_D.*m_pend.*cos(THE_Psi).*cos(THE_Theta).*cos(THE_Phi_pend).*cos(THE_Psi_pend).^2.*cos(THE_Theta_pend).^2.*sin(THE_Psi).*sin(THE_Phi_pend).*(2.0./3.0)+Lz_pend.^2.*THE_Psi_pend_D.*m_pend.*cos(THE_Psi).*cos(THE_Theta).*cos(THE_Phi_pend).^2.*cos(THE_Psi_pend).*cos(THE_Theta_pend).^2.*sin(THE_Psi).*sin(THE_Psi_pend).*(2.0./3.0)+Lz_pend.^2.*THE_Theta_pend_D.*m_pend.*cos(THE_Psi).*cos(THE_Theta).*cos(THE_Phi_pend).^2.*cos(THE_Psi_pend).^2.*cos(THE_Theta_pend).*sin(THE_Psi).*sin(THE_Theta_pend).*(2.0./3.0)+(Ly_pend.^2.*THE_Psi_D.*m_pend.*cos(THE_Psi).*cos(THE_Theta).*cos(THE_Phi_pend).*cos(THE_Psi_pend).*cos(THE_Theta_pend).*sin(THE_Psi).*sin(THE_Psi_pend))./3.0-Lz_pend.^2.*THE_Psi_D.*m_pend.*cos(THE_Psi).*cos(THE_Theta).*cos(THE_Phi_pend).*cos(THE_Psi_pend).*cos(THE_Theta_pend).*sin(THE_Psi).*sin(THE_Psi_pend).*(4.0./3.0);
    et299 = Ly_pend.^2.*THE_Theta_pend_D.*m_pend.*cos(THE_Psi).*cos(THE_Theta).*cos(THE_Phi_pend).*cos(THE_Psi_pend).*cos(THE_Theta_pend).*sin(THE_Psi).*sin(THE_Phi_pend).*sin(THE_Psi_pend).*(-1.0./6.0)+Lz_pend.^2.*THE_Theta_pend_D.*m_pend.*cos(THE_Psi).*cos(THE_Theta).*cos(THE_Phi_pend).*cos(THE_Psi_pend).*cos(THE_Theta_pend).*sin(THE_Psi).*sin(THE_Phi_pend).*sin(THE_Psi_pend).*(2.0./3.0)+(Ly_pend.^2.*THE_Theta_D.*m_pend.*cos(THE_Psi).*cos(THE_Phi_pend).*cos(THE_Psi_pend).*sin(THE_Psi).*sin(THE_Theta).*sin(THE_Phi_pend).*sin(THE_Psi_pend).*sin(THE_Theta_pend))./6.0-Lz_pend.^2.*THE_Theta_D.*m_pend.*cos(THE_Psi).*cos(THE_Phi_pend).*cos(THE_Psi_pend).*sin(THE_Psi).*sin(THE_Theta).*sin(THE_Phi_pend).*sin(THE_Psi_pend).*sin(THE_Theta_pend).*(2.0./3.0);
    et300 = (Ly_pend.^2.*THE_Psi_D.*sin(THE_Psi_pend.*2.0))./2.0-Lz_pend.^2.*THE_Psi_D.*sin(THE_Psi_pend.*2.0).*2.0+Ly_pend.^2.*THE_Theta_pend_D.*cos(THE_Phi_pend).*sin(THE_Theta_pend).*2.0+Lz_pend.^2.*THE_Phi_pend_D.*cos(THE_Theta_pend).*sin(THE_Phi_pend).*8.0-Ly_pend.^2.*THE_Psi_D.*cos(THE_Phi_pend).*sin(THE_Phi_pend).*sin(THE_Theta_pend)-Ly_pend.^2.*THE_Theta_pend_D.*cos(THE_Psi_pend).*sin(THE_Phi_pend).*sin(THE_Psi_pend).*2.0+Lz_pend.^2.*THE_Psi_D.*cos(THE_Phi_pend).*sin(THE_Phi_pend).*sin(THE_Theta_pend).*4.0+Lz_pend.^2.*THE_Theta_pend_D.*cos(THE_Psi_pend).*sin(THE_Phi_pend).*sin(THE_Psi_pend).*8.0-Lz_pend.*THE_Psi_D.*Tv_Z_pend.*cos(THE_Theta_pend).*sin(THE_Psi_pend).*6.0-Ly_pend.^2.*THE_Psi_D.*cos(THE_Phi_pend).^2.*cos(THE_Psi_pend).*sin(THE_Psi_pend).*2.0+Ly_pend.^2.*THE_Phi_pend_D.*cos(THE_Psi_pend).^2.*cos(THE_Theta_pend).*sin(THE_Phi_pend).*2.0-Ly_pend.^2.*THE_Theta_pend_D.*cos(THE_Phi_pend).*cos(THE_Psi_pend).^2.*sin(THE_Theta_pend).*2.0+Lz_pend.^2.*THE_Psi_D.*cos(THE_Phi_pend).^2.*cos(THE_Psi_pend).*sin(THE_Psi_pend).*8.0-Lz_pend.^2.*THE_Phi_pend_D.*cos(THE_Psi_pend).^2.*cos(THE_Theta_pend).*sin(THE_Phi_pend).*8.0+Lz_pend.^2.*THE_Theta_pend_D.*cos(THE_Phi_pend).*cos(THE_Psi_pend).^2.*sin(THE_Theta_pend).*8.0;
    et301 = Ly_pend.^2.*THE_Psi_D.*cos(THE_Phi_pend).^2.*cos(THE_Psi_pend).*cos(THE_Theta_pend).^2.*sin(THE_Psi_pend)-Lz_pend.^2.*THE_Psi_D.*cos(THE_Phi_pend).^2.*cos(THE_Psi_pend).*cos(THE_Theta_pend).^2.*sin(THE_Psi_pend).*4.0+Ly_pend.^2.*THE_Psi_D.*cos(THE_Phi_pend).*cos(THE_Psi_pend).^2.*sin(THE_Phi_pend).*sin(THE_Theta_pend).*2.0-Lz_pend.^2.*THE_Psi_D.*cos(THE_Phi_pend).*cos(THE_Psi_pend).^2.*sin(THE_Phi_pend).*sin(THE_Theta_pend).*8.0-Ly_pend.^2.*THE_Phi_pend_D.*cos(THE_Phi_pend).*cos(THE_Psi_pend).*cos(THE_Theta_pend).*sin(THE_Psi_pend).*sin(THE_Theta_pend).*2.0+Lz_pend.^2.*THE_Phi_pend_D.*cos(THE_Phi_pend).*cos(THE_Psi_pend).*cos(THE_Theta_pend).*sin(THE_Psi_pend).*sin(THE_Theta_pend).*8.0;
    et302 = Ly_pend.^2.*THE_Phi_pend_D.*m_pend.*cos(THE_Phi_pend).*(-1.0./6.0)+(Ly_pend.^2.*THE_Psi_pend_D.*m_pend.*cos(THE_Phi_pend).*sin(THE_Theta_pend))./6.0-(Lx_pend.^2.*THE_Phi_pend_D.*m_pend.*cos(THE_Phi_pend).*cos(THE_Theta_pend).^2)./6.0+(Ly_pend.^2.*THE_Phi_pend_D.*m_pend.*cos(THE_Phi_pend).*cos(THE_Psi_pend).^2)./6.0+(Ly_pend.^2.*THE_Phi_pend_D.*m_pend.*cos(THE_Phi_pend).*cos(THE_Theta_pend).^2)./6.0-Lz_pend.^2.*THE_Phi_pend_D.*m_pend.*cos(THE_Phi_pend).*cos(THE_Psi_pend).^2.*(2.0./3.0)-(Ly_pend.^2.*THE_Psi_pend_D.*m_pend.*cos(THE_Psi_pend).*sin(THE_Phi_pend).*sin(THE_Psi_pend))./6.0+Lz_pend.^2.*THE_Psi_pend_D.*m_pend.*cos(THE_Psi_pend).*sin(THE_Phi_pend).*sin(THE_Psi_pend).*(2.0./3.0)+(Lz_pend.*THE_Psi_D.*Tv_Z_pend.*m_pend.*cos(THE_Psi_pend).*sin(THE_Theta_pend))./2.0-(Lx_pend.^2.*THE_Psi_D.*m_pend.*cos(THE_Phi_pend).^2.*cos(THE_Theta_pend).*sin(THE_Theta_pend))./1.2e+1+(Ly_pend.^2.*THE_Psi_D.*m_pend.*cos(THE_Phi_pend).^2.*cos(THE_Theta_pend).*sin(THE_Theta_pend))./1.2e+1-(Ly_pend.^2.*THE_Psi_pend_D.*m_pend.*cos(THE_Phi_pend).*cos(THE_Psi_pend).^2.*sin(THE_Theta_pend))./6.0;
    et303 = Lz_pend.^2.*THE_Psi_pend_D.*m_pend.*cos(THE_Phi_pend).*cos(THE_Psi_pend).^2.*sin(THE_Theta_pend).*(2.0./3.0)-(Ly_pend.^2.*THE_Phi_pend_D.*m_pend.*cos(THE_Phi_pend).*cos(THE_Psi_pend).^2.*cos(THE_Theta_pend).^2)./6.0+Lz_pend.^2.*THE_Phi_pend_D.*m_pend.*cos(THE_Phi_pend).*cos(THE_Psi_pend).^2.*cos(THE_Theta_pend).^2.*(2.0./3.0)-(Ly_pend.^2.*THE_Psi_D.*m_pend.*cos(THE_Phi_pend).^2.*cos(THE_Psi_pend).^2.*cos(THE_Theta_pend).*sin(THE_Theta_pend))./1.2e+1+(Lz_pend.^2.*THE_Psi_D.*m_pend.*cos(THE_Phi_pend).^2.*cos(THE_Psi_pend).^2.*cos(THE_Theta_pend).*sin(THE_Theta_pend))./3.0+(Ly_pend.^2.*THE_Phi_pend_D.*m_pend.*cos(THE_Psi_pend).*sin(THE_Phi_pend).*sin(THE_Psi_pend).*sin(THE_Theta_pend))./6.0-Lz_pend.^2.*THE_Phi_pend_D.*m_pend.*cos(THE_Psi_pend).*sin(THE_Phi_pend).*sin(THE_Psi_pend).*sin(THE_Theta_pend).*(2.0./3.0)-(Ly_pend.^2.*THE_Psi_D.*m_pend.*cos(THE_Phi_pend).*cos(THE_Psi_pend).*cos(THE_Theta_pend).*sin(THE_Phi_pend).*sin(THE_Psi_pend))./1.2e+1+(Lz_pend.^2.*THE_Psi_D.*m_pend.*cos(THE_Phi_pend).*cos(THE_Psi_pend).*cos(THE_Theta_pend).*sin(THE_Phi_pend).*sin(THE_Psi_pend))./3.0;
    et304 = Ly_pend.^2.*THE_Theta_pend_D.*cos(THE_Phi_pend).*2.0-(Ly_pend.^2.*THE_Psi_D.*sin(THE_Phi_pend.*2.0))./2.0+Lz_pend.^2.*THE_Psi_D.*sin(THE_Phi_pend.*2.0).*2.0+Lx_pend.^2.*THE_Theta_pend_D.*cos(THE_Phi_pend).*cos(THE_Theta_pend).^2.*2.0-Ly_pend.^2.*THE_Theta_pend_D.*cos(THE_Phi_pend).*cos(THE_Psi_pend).^2.*2.0-Ly_pend.^2.*THE_Theta_pend_D.*cos(THE_Phi_pend).*cos(THE_Theta_pend).^2.*2.0+Lz_pend.^2.*THE_Theta_pend_D.*cos(THE_Phi_pend).*cos(THE_Psi_pend).^2.*8.0+Lz_pend.^2.*THE_Psi_pend_D.*cos(THE_Theta_pend).*sin(THE_Phi_pend).*8.0+Ly_pend.^2.*THE_Theta_pend_D.*cos(THE_Phi_pend).*cos(THE_Psi_pend).^2.*cos(THE_Theta_pend).^2.*2.0-Lz_pend.^2.*THE_Theta_pend_D.*cos(THE_Phi_pend).*cos(THE_Psi_pend).^2.*cos(THE_Theta_pend).^2.*8.0+Ly_pend.^2.*THE_Psi_D.*cos(THE_Psi_pend).*sin(THE_Psi_pend).*sin(THE_Theta_pend)-Lz_pend.^2.*THE_Psi_D.*cos(THE_Psi_pend).*sin(THE_Psi_pend).*sin(THE_Theta_pend).*4.0-Lx_pend.^2.*THE_Psi_D.*cos(THE_Phi_pend).*cos(THE_Theta_pend).^2.*sin(THE_Phi_pend)+Ly_pend.^2.*THE_Psi_D.*cos(THE_Phi_pend).*cos(THE_Psi_pend).^2.*sin(THE_Phi_pend).*2.0+Ly_pend.^2.*THE_Psi_D.*cos(THE_Phi_pend).*cos(THE_Theta_pend).^2.*sin(THE_Phi_pend);
    et305 = Ly_pend.^2.*THE_Psi_pend_D.*cos(THE_Psi_pend).^2.*cos(THE_Theta_pend).*sin(THE_Phi_pend).*2.0-Lz_pend.^2.*THE_Psi_D.*cos(THE_Phi_pend).*cos(THE_Psi_pend).^2.*sin(THE_Phi_pend).*8.0-Lz_pend.^2.*THE_Psi_pend_D.*cos(THE_Psi_pend).^2.*cos(THE_Theta_pend).*sin(THE_Phi_pend).*8.0-Ly_pend.^2.*THE_Psi_D.*cos(THE_Phi_pend).*cos(THE_Psi_pend).^2.*cos(THE_Theta_pend).^2.*sin(THE_Phi_pend)+Lz_pend.^2.*THE_Psi_D.*cos(THE_Phi_pend).*cos(THE_Psi_pend).^2.*cos(THE_Theta_pend).^2.*sin(THE_Phi_pend).*4.0-Ly_pend.^2.*THE_Theta_pend_D.*cos(THE_Psi_pend).*sin(THE_Phi_pend).*sin(THE_Psi_pend).*sin(THE_Theta_pend).*2.0+Lz_pend.^2.*THE_Theta_pend_D.*cos(THE_Psi_pend).*sin(THE_Phi_pend).*sin(THE_Psi_pend).*sin(THE_Theta_pend).*8.0-Ly_pend.^2.*THE_Psi_D.*cos(THE_Phi_pend).^2.*cos(THE_Psi_pend).*sin(THE_Psi_pend).*sin(THE_Theta_pend).*2.0+Lz_pend.^2.*THE_Psi_D.*cos(THE_Phi_pend).^2.*cos(THE_Psi_pend).*sin(THE_Psi_pend).*sin(THE_Theta_pend).*8.0-Ly_pend.^2.*THE_Psi_pend_D.*cos(THE_Phi_pend).*cos(THE_Psi_pend).*cos(THE_Theta_pend).*sin(THE_Psi_pend).*sin(THE_Theta_pend).*2.0+Lz_pend.^2.*THE_Psi_pend_D.*cos(THE_Phi_pend).*cos(THE_Psi_pend).*cos(THE_Theta_pend).*sin(THE_Psi_pend).*sin(THE_Theta_pend).*8.0;
    et306 = THE_Psi_D.*cg_to_mot_H.*mprop.*cos(THE_Phi).*sin(THE_Psi).*4.0+THE_Psi_D.*Tv_Z_pend.*m_pend.*cos(THE_Phi).*sin(THE_Psi)-THE_Psi_D.*Tv_Z_pend.*m_pend.*cos(THE_Psi).*sin(THE_Phi).*sin(THE_Theta)-THE_Psi_D.*cg_to_mot_H.*mprop.*cos(THE_Psi).*sin(THE_Phi).*sin(THE_Theta).*4.0+(Lz_pend.*THE_Psi_D.*m_pend.*cos(THE_Phi).*cos(THE_Psi).*cos(THE_Phi_pend).*sin(THE_Psi_pend))./2.0+(Lz_pend.*THE_Psi_D.*m_pend.*cos(THE_Phi).*cos(THE_Psi_pend).*cos(THE_Theta_pend).*sin(THE_Psi))./2.0+Lz_pend.*THE_Psi_pend_D.*m_pend.*cos(THE_Phi).*cos(THE_Phi_pend).*cos(THE_Psi_pend).*sin(THE_Psi)+Lz_pend.*THE_Psi_pend_D.*m_pend.*cos(THE_Phi).*cos(THE_Psi).*cos(THE_Theta_pend).*sin(THE_Psi_pend)+Lz_pend.*THE_Theta_pend_D.*m_pend.*cos(THE_Phi).*cos(THE_Psi).*cos(THE_Psi_pend).*sin(THE_Theta_pend)-Lz_pend.*THE_Phi_pend_D.*m_pend.*cos(THE_Phi).*sin(THE_Psi).*sin(THE_Phi_pend).*sin(THE_Psi_pend)-(Lz_pend.*THE_Psi_D.*m_pend.*cos(THE_Psi).*cos(THE_Psi_pend).*cos(THE_Theta_pend).*sin(THE_Phi).*sin(THE_Theta))./2.0-(Lz_pend.*THE_Psi_D.*m_pend.*cos(THE_Phi).*cos(THE_Psi).*cos(THE_Psi_pend).*sin(THE_Phi_pend).*sin(THE_Theta_pend))./2.0-Lz_pend.*THE_Psi_pend_D.*m_pend.*cos(THE_Psi).*cos(THE_Phi_pend).*cos(THE_Psi_pend).*sin(THE_Phi).*sin(THE_Theta)-Lz_pend.*THE_Phi_pend_D.*m_pend.*cos(THE_Phi).*cos(THE_Phi_pend).*cos(THE_Psi_pend).*sin(THE_Psi).*sin(THE_Theta_pend);
    et307 = -Lz_pend.*THE_Theta_pend_D.*m_pend.*cos(THE_Phi).*cos(THE_Psi_pend).*cos(THE_Theta_pend).*sin(THE_Psi).*sin(THE_Phi_pend)+(Lz_pend.*THE_Psi_D.*m_pend.*cos(THE_Phi_pend).*sin(THE_Phi).*sin(THE_Psi).*sin(THE_Theta).*sin(THE_Psi_pend))./2.0+Lz_pend.*THE_Phi_pend_D.*m_pend.*cos(THE_Psi).*sin(THE_Phi).*sin(THE_Theta).*sin(THE_Phi_pend).*sin(THE_Psi_pend)+Lz_pend.*THE_Psi_pend_D.*m_pend.*cos(THE_Theta_pend).*sin(THE_Phi).*sin(THE_Psi).*sin(THE_Theta).*sin(THE_Psi_pend)+Lz_pend.*THE_Theta_pend_D.*m_pend.*cos(THE_Psi_pend).*sin(THE_Phi).*sin(THE_Psi).*sin(THE_Theta).*sin(THE_Theta_pend)+Lz_pend.*THE_Psi_pend_D.*m_pend.*cos(THE_Phi).*sin(THE_Psi).*sin(THE_Phi_pend).*sin(THE_Psi_pend).*sin(THE_Theta_pend)-(Lz_pend.*THE_Psi_D.*m_pend.*cos(THE_Psi_pend).*sin(THE_Phi).*sin(THE_Psi).*sin(THE_Theta).*sin(THE_Phi_pend).*sin(THE_Theta_pend))./2.0-Lz_pend.*THE_Psi_pend_D.*m_pend.*cos(THE_Psi).*sin(THE_Phi).*sin(THE_Theta).*sin(THE_Phi_pend).*sin(THE_Psi_pend).*sin(THE_Theta_pend)+Lz_pend.*THE_Phi_pend_D.*m_pend.*cos(THE_Psi).*cos(THE_Phi_pend).*cos(THE_Psi_pend).*sin(THE_Phi).*sin(THE_Theta).*sin(THE_Theta_pend)+Lz_pend.*THE_Theta_pend_D.*m_pend.*cos(THE_Psi).*cos(THE_Psi_pend).*cos(THE_Theta_pend).*sin(THE_Phi).*sin(THE_Theta).*sin(THE_Phi_pend);
    et308 = -THE_Psi_D.*Tv_Z_pend.*m_pend.*sin(THE_Phi).*sin(THE_Psi)-THE_Psi_D.*cg_to_mot_H.*mprop.*sin(THE_Phi).*sin(THE_Psi).*4.0-THE_Psi_D.*Tv_Z_pend.*m_pend.*cos(THE_Phi).*cos(THE_Psi).*sin(THE_Theta)-THE_Psi_D.*cg_to_mot_H.*mprop.*cos(THE_Phi).*cos(THE_Psi).*sin(THE_Theta).*4.0-(Lz_pend.*THE_Psi_D.*m_pend.*cos(THE_Psi).*cos(THE_Phi_pend).*sin(THE_Phi).*sin(THE_Psi_pend))./2.0-(Lz_pend.*THE_Psi_D.*m_pend.*cos(THE_Psi_pend).*cos(THE_Theta_pend).*sin(THE_Phi).*sin(THE_Psi))./2.0-Lz_pend.*THE_Psi_pend_D.*m_pend.*cos(THE_Phi_pend).*cos(THE_Psi_pend).*sin(THE_Phi).*sin(THE_Psi)-Lz_pend.*THE_Psi_pend_D.*m_pend.*cos(THE_Psi).*cos(THE_Theta_pend).*sin(THE_Phi).*sin(THE_Psi_pend)-Lz_pend.*THE_Theta_pend_D.*m_pend.*cos(THE_Psi).*cos(THE_Psi_pend).*sin(THE_Phi).*sin(THE_Theta_pend)+Lz_pend.*THE_Phi_pend_D.*m_pend.*sin(THE_Phi).*sin(THE_Psi).*sin(THE_Phi_pend).*sin(THE_Psi_pend)-(Lz_pend.*THE_Psi_D.*m_pend.*cos(THE_Phi).*cos(THE_Psi).*cos(THE_Psi_pend).*cos(THE_Theta_pend).*sin(THE_Theta))./2.0-Lz_pend.*THE_Psi_pend_D.*m_pend.*cos(THE_Phi).*cos(THE_Psi).*cos(THE_Phi_pend).*cos(THE_Psi_pend).*sin(THE_Theta)+(Lz_pend.*THE_Psi_D.*m_pend.*cos(THE_Phi).*cos(THE_Phi_pend).*sin(THE_Psi).*sin(THE_Theta).*sin(THE_Psi_pend))./2.0+Lz_pend.*THE_Phi_pend_D.*m_pend.*cos(THE_Phi).*cos(THE_Psi).*sin(THE_Theta).*sin(THE_Phi_pend).*sin(THE_Psi_pend);
    et309 = (Lz_pend.*THE_Psi_D.*m_pend.*cos(THE_Psi).*cos(THE_Psi_pend).*sin(THE_Phi).*sin(THE_Phi_pend).*sin(THE_Theta_pend))./2.0+Lz_pend.*THE_Psi_pend_D.*m_pend.*cos(THE_Phi).*cos(THE_Theta_pend).*sin(THE_Psi).*sin(THE_Theta).*sin(THE_Psi_pend)+Lz_pend.*THE_Theta_pend_D.*m_pend.*cos(THE_Phi).*cos(THE_Psi_pend).*sin(THE_Psi).*sin(THE_Theta).*sin(THE_Theta_pend)+Lz_pend.*THE_Phi_pend_D.*m_pend.*cos(THE_Phi_pend).*cos(THE_Psi_pend).*sin(THE_Phi).*sin(THE_Psi).*sin(THE_Theta_pend)+Lz_pend.*THE_Theta_pend_D.*m_pend.*cos(THE_Psi_pend).*cos(THE_Theta_pend).*sin(THE_Phi).*sin(THE_Psi).*sin(THE_Phi_pend)-Lz_pend.*THE_Psi_pend_D.*m_pend.*sin(THE_Phi).*sin(THE_Psi).*sin(THE_Phi_pend).*sin(THE_Psi_pend).*sin(THE_Theta_pend)+Lz_pend.*THE_Phi_pend_D.*m_pend.*cos(THE_Phi).*cos(THE_Psi).*cos(THE_Phi_pend).*cos(THE_Psi_pend).*sin(THE_Theta).*sin(THE_Theta_pend)+Lz_pend.*THE_Theta_pend_D.*m_pend.*cos(THE_Phi).*cos(THE_Psi).*cos(THE_Psi_pend).*cos(THE_Theta_pend).*sin(THE_Theta).*sin(THE_Phi_pend)-(Lz_pend.*THE_Psi_D.*m_pend.*cos(THE_Phi).*cos(THE_Psi_pend).*sin(THE_Psi).*sin(THE_Theta).*sin(THE_Phi_pend).*sin(THE_Theta_pend))./2.0-Lz_pend.*THE_Psi_pend_D.*m_pend.*cos(THE_Phi).*cos(THE_Psi).*sin(THE_Theta).*sin(THE_Phi_pend).*sin(THE_Psi_pend).*sin(THE_Theta_pend);
    et310 = (Ly_pend.^2.*THE_Phi_pend_D.*m_pend.*sin(THE_Phi_pend.*2.0))./1.2e+1+(Ly_pend.^2.*THE_Psi_pend_D.*m_pend.*sin(THE_Psi_pend.*2.0))./1.2e+1-(Lz_pend.^2.*THE_Phi_pend_D.*m_pend.*sin(THE_Phi_pend.*2.0))./3.0-(Lz_pend.^2.*THE_Psi_pend_D.*m_pend.*sin(THE_Psi_pend.*2.0))./3.0-(Ly_pend.^2.*THE_Psi_pend_D.*m_pend.*cos(THE_Phi_pend).*sin(THE_Phi_pend).*sin(THE_Theta_pend))./6.0-(Ly_pend.^2.*THE_Phi_pend_D.*m_pend.*cos(THE_Psi_pend).*sin(THE_Psi_pend).*sin(THE_Theta_pend))./6.0+Lz_pend.^2.*THE_Psi_pend_D.*m_pend.*cos(THE_Phi_pend).*sin(THE_Phi_pend).*sin(THE_Theta_pend).*(2.0./3.0)+Lz_pend.^2.*THE_Phi_pend_D.*m_pend.*cos(THE_Psi_pend).*sin(THE_Psi_pend).*sin(THE_Theta_pend).*(2.0./3.0)-Lz_pend.*THE_Psi_pend_D.*Tv_Z_pend.*m_pend.*cos(THE_Theta_pend).*sin(THE_Psi_pend)-Lz_pend.*THE_Theta_pend_D.*Tv_Z_pend.*m_pend.*cos(THE_Psi_pend).*sin(THE_Theta_pend)+(Lx_pend.^2.*THE_Phi_pend_D.*m_pend.*cos(THE_Phi_pend).*cos(THE_Theta_pend).^2.*sin(THE_Phi_pend))./6.0+(Lx_pend.^2.*THE_Theta_pend_D.*m_pend.*cos(THE_Phi_pend).^2.*cos(THE_Theta_pend).*sin(THE_Theta_pend))./6.0-(Ly_pend.^2.*THE_Phi_pend_D.*m_pend.*cos(THE_Phi_pend).*cos(THE_Psi_pend).^2.*sin(THE_Phi_pend))./3.0;
    et311 = Ly_pend.^2.*THE_Psi_pend_D.*m_pend.*cos(THE_Phi_pend).^2.*cos(THE_Psi_pend).*sin(THE_Psi_pend).*(-1.0./3.0)-(Ly_pend.^2.*THE_Phi_pend_D.*m_pend.*cos(THE_Phi_pend).*cos(THE_Theta_pend).^2.*sin(THE_Phi_pend))./6.0-(Ly_pend.^2.*THE_Theta_pend_D.*m_pend.*cos(THE_Phi_pend).^2.*cos(THE_Theta_pend).*sin(THE_Theta_pend))./6.0+Lz_pend.^2.*THE_Phi_pend_D.*m_pend.*cos(THE_Phi_pend).*cos(THE_Psi_pend).^2.*sin(THE_Phi_pend).*(4.0./3.0)+Lz_pend.^2.*THE_Psi_pend_D.*m_pend.*cos(THE_Phi_pend).^2.*cos(THE_Psi_pend).*sin(THE_Psi_pend).*(4.0./3.0)+(Ly_pend.^2.*THE_Phi_pend_D.*m_pend.*cos(THE_Phi_pend).^2.*cos(THE_Psi_pend).*sin(THE_Psi_pend).*sin(THE_Theta_pend))./3.0+(Ly_pend.^2.*THE_Psi_pend_D.*m_pend.*cos(THE_Phi_pend).*cos(THE_Psi_pend).^2.*sin(THE_Phi_pend).*sin(THE_Theta_pend))./3.0-Lz_pend.^2.*THE_Phi_pend_D.*m_pend.*cos(THE_Phi_pend).^2.*cos(THE_Psi_pend).*sin(THE_Psi_pend).*sin(THE_Theta_pend).*(4.0./3.0)-Lz_pend.^2.*THE_Psi_pend_D.*m_pend.*cos(THE_Phi_pend).*cos(THE_Psi_pend).^2.*sin(THE_Phi_pend).*sin(THE_Theta_pend).*(4.0./3.0)+(Ly_pend.^2.*THE_Phi_pend_D.*m_pend.*cos(THE_Phi_pend).*cos(THE_Psi_pend).^2.*cos(THE_Theta_pend).^2.*sin(THE_Phi_pend))./6.0;
    et312 = (Ly_pend.^2.*THE_Psi_pend_D.*m_pend.*cos(THE_Phi_pend).^2.*cos(THE_Psi_pend).*cos(THE_Theta_pend).^2.*sin(THE_Psi_pend))./6.0+(Ly_pend.^2.*THE_Theta_pend_D.*m_pend.*cos(THE_Phi_pend).^2.*cos(THE_Psi_pend).^2.*cos(THE_Theta_pend).*sin(THE_Theta_pend))./6.0-Lz_pend.^2.*THE_Phi_pend_D.*m_pend.*cos(THE_Phi_pend).*cos(THE_Psi_pend).^2.*cos(THE_Theta_pend).^2.*sin(THE_Phi_pend).*(2.0./3.0)-Lz_pend.^2.*THE_Psi_pend_D.*m_pend.*cos(THE_Phi_pend).^2.*cos(THE_Psi_pend).*cos(THE_Theta_pend).^2.*sin(THE_Psi_pend).*(2.0./3.0)-Lz_pend.^2.*THE_Theta_pend_D.*m_pend.*cos(THE_Phi_pend).^2.*cos(THE_Psi_pend).^2.*cos(THE_Theta_pend).*sin(THE_Theta_pend).*(2.0./3.0)+(Ly_pend.^2.*THE_Theta_pend_D.*m_pend.*cos(THE_Phi_pend).*cos(THE_Psi_pend).*cos(THE_Theta_pend).*sin(THE_Phi_pend).*sin(THE_Psi_pend))./6.0-Lz_pend.^2.*THE_Theta_pend_D.*m_pend.*cos(THE_Phi_pend).*cos(THE_Psi_pend).*cos(THE_Theta_pend).*sin(THE_Phi_pend).*sin(THE_Psi_pend).*(2.0./3.0);
    et313 = -I_xz.*THE_Psi_D.*cos(THE_Psi)-Iprop_xz.*THE_Psi_D.*cos(THE_Psi).*4.0-I_xy.*THE_Psi_D.*sin(THE_Psi)-Iprop_xy.*THE_Psi_D.*sin(THE_Psi).*4.0-Iprop_zz.*wMOT_1.*cos(THE_Psi)-Iprop_zz.*wMOT_2.*cos(THE_Psi)-Iprop_zz.*wMOT_3.*cos(THE_Psi)-Iprop_zz.*wMOT_4.*cos(THE_Psi)-Iprop_yz.*wMOT_1.*sin(THE_Psi)-Iprop_yz.*wMOT_2.*sin(THE_Psi)-Iprop_yz.*wMOT_3.*sin(THE_Psi)-Iprop_yz.*wMOT_4.*sin(THE_Psi)-Lz_pend.^2.*THE_Phi_pend_D.*m_pend.*cos(THE_Psi).*(2.0./3.0)-(Ly_pend.^2.*THE_Theta_pend_D.*m_pend.*cos(THE_Phi_pend).*sin(THE_Psi))./6.0+Lz_pend.^2.*THE_Psi_pend_D.*m_pend.*cos(THE_Psi).*sin(THE_Theta_pend).*(2.0./3.0)-(Ly_pend.^2.*THE_Phi_pend_D.*m_pend.*cos(THE_Psi).*cos(THE_Phi_pend).^2)./6.0-(Ly_pend.^2.*THE_Phi_pend_D.*m_pend.*cos(THE_Psi).*cos(THE_Psi_pend).^2)./6.0+Lz_pend.^2.*THE_Phi_pend_D.*m_pend.*cos(THE_Psi).*cos(THE_Phi_pend).^2.*(2.0./3.0)+Lz_pend.^2.*THE_Phi_pend_D.*m_pend.*cos(THE_Psi).*cos(THE_Psi_pend).^2.*(2.0./3.0);
    et314 = (Ly_pend.^2.*THE_Psi_D.*m_pend.*cos(THE_Phi_pend).*sin(THE_Psi).*sin(THE_Phi_pend))./1.2e+1-(Lz_pend.^2.*THE_Psi_D.*m_pend.*cos(THE_Phi_pend).*sin(THE_Psi).*sin(THE_Phi_pend))./3.0-Lz_pend.^2.*THE_Psi_pend_D.*m_pend.*cos(THE_Theta_pend).*sin(THE_Psi).*sin(THE_Phi_pend).*(2.0./3.0)-(Lx_pend.^2.*THE_Theta_pend_D.*m_pend.*cos(THE_Phi_pend).*cos(THE_Theta_pend).^2.*sin(THE_Psi))./6.0+(Ly_pend.^2.*THE_Psi_pend_D.*m_pend.*cos(THE_Psi).*cos(THE_Phi_pend).^2.*sin(THE_Theta_pend))./6.0+(Ly_pend.^2.*THE_Theta_pend_D.*m_pend.*cos(THE_Phi_pend).*cos(THE_Psi_pend).^2.*sin(THE_Psi))./6.0+(Ly_pend.^2.*THE_Psi_pend_D.*m_pend.*cos(THE_Psi).*cos(THE_Psi_pend).^2.*sin(THE_Theta_pend))./6.0+(Ly_pend.^2.*THE_Theta_pend_D.*m_pend.*cos(THE_Phi_pend).*cos(THE_Theta_pend).^2.*sin(THE_Psi))./6.0-Lz_pend.^2.*THE_Psi_pend_D.*m_pend.*cos(THE_Psi).*cos(THE_Phi_pend).^2.*sin(THE_Theta_pend).*(2.0./3.0)-Lz_pend.^2.*THE_Theta_pend_D.*m_pend.*cos(THE_Phi_pend).*cos(THE_Psi_pend).^2.*sin(THE_Psi).*(2.0./3.0)-Lz_pend.^2.*THE_Psi_pend_D.*m_pend.*cos(THE_Psi).*cos(THE_Psi_pend).^2.*sin(THE_Theta_pend).*(2.0./3.0);
    et315 = Lx_pend.^2.*THE_Phi_pend_D.*m_pend.*cos(THE_Psi).*cos(THE_Phi_pend).^2.*cos(THE_Theta_pend).^2.*(-1.0./6.0)+(Ly_pend.^2.*THE_Phi_pend_D.*m_pend.*cos(THE_Psi).*cos(THE_Phi_pend).^2.*cos(THE_Psi_pend).^2)./3.0+(Ly_pend.^2.*THE_Phi_pend_D.*m_pend.*cos(THE_Psi).*cos(THE_Phi_pend).^2.*cos(THE_Theta_pend).^2)./6.0-Lz_pend.^2.*THE_Phi_pend_D.*m_pend.*cos(THE_Psi).*cos(THE_Phi_pend).^2.*cos(THE_Psi_pend).^2.*(4.0./3.0)+(Lz_pend.*THE_Psi_D.*Tv_Z_pend.*m_pend.*cos(THE_Psi).*sin(THE_Phi_pend).*sin(THE_Psi_pend))./2.0+(Lx_pend.^2.*THE_Psi_D.*m_pend.*cos(THE_Phi_pend).*cos(THE_Theta_pend).^2.*sin(THE_Psi).*sin(THE_Phi_pend))./1.2e+1-(Ly_pend.^2.*THE_Psi_D.*m_pend.*cos(THE_Phi_pend).*cos(THE_Psi_pend).^2.*sin(THE_Psi).*sin(THE_Phi_pend))./6.0-(Ly_pend.^2.*THE_Psi_D.*m_pend.*cos(THE_Phi_pend).*cos(THE_Theta_pend).^2.*sin(THE_Psi).*sin(THE_Phi_pend))./1.2e+1-(Ly_pend.^2.*THE_Psi_pend_D.*m_pend.*cos(THE_Psi_pend).^2.*cos(THE_Theta_pend).*sin(THE_Psi).*sin(THE_Phi_pend))./6.0+Lz_pend.^2.*THE_Psi_D.*m_pend.*cos(THE_Phi_pend).*cos(THE_Psi_pend).^2.*sin(THE_Psi).*sin(THE_Phi_pend).*(2.0./3.0);
    et316 = Lz_pend.^2.*THE_Psi_pend_D.*m_pend.*cos(THE_Psi_pend).^2.*cos(THE_Theta_pend).*sin(THE_Psi).*sin(THE_Phi_pend).*(2.0./3.0)-(Ly_pend.^2.*THE_Psi_pend_D.*m_pend.*cos(THE_Psi).*cos(THE_Phi_pend).^2.*cos(THE_Psi_pend).^2.*sin(THE_Theta_pend))./3.0-(Ly_pend.^2.*THE_Theta_pend_D.*m_pend.*cos(THE_Phi_pend).*cos(THE_Psi_pend).^2.*cos(THE_Theta_pend).^2.*sin(THE_Psi))./6.0+Lz_pend.^2.*THE_Psi_pend_D.*m_pend.*cos(THE_Psi).*cos(THE_Phi_pend).^2.*cos(THE_Psi_pend).^2.*sin(THE_Theta_pend).*(4.0./3.0)+Lz_pend.^2.*THE_Theta_pend_D.*m_pend.*cos(THE_Phi_pend).*cos(THE_Psi_pend).^2.*cos(THE_Theta_pend).^2.*sin(THE_Psi).*(2.0./3.0)-(Lx_pend.^2.*THE_Psi_D.*m_pend.*cos(THE_Psi).*cos(THE_Phi_pend).*cos(THE_Theta_pend).*sin(THE_Theta_pend))./1.2e+1+(Ly_pend.^2.*THE_Psi_D.*m_pend.*cos(THE_Psi).*cos(THE_Phi_pend).*cos(THE_Theta_pend).*sin(THE_Theta_pend))./1.2e+1+(Ly_pend.^2.*THE_Theta_pend_D.*m_pend.*cos(THE_Psi).*cos(THE_Psi_pend).*cos(THE_Theta_pend).*sin(THE_Psi_pend))./6.0-Lz_pend.^2.*THE_Theta_pend_D.*m_pend.*cos(THE_Psi).*cos(THE_Psi_pend).*cos(THE_Theta_pend).*sin(THE_Psi_pend).*(2.0./3.0);
    et317 = Ly_pend.^2.*THE_Phi_pend_D.*m_pend.*cos(THE_Psi).*cos(THE_Phi_pend).^2.*cos(THE_Psi_pend).^2.*cos(THE_Theta_pend).^2.*(-1.0./6.0)+Lz_pend.^2.*THE_Phi_pend_D.*m_pend.*cos(THE_Psi).*cos(THE_Phi_pend).^2.*cos(THE_Psi_pend).^2.*cos(THE_Theta_pend).^2.*(2.0./3.0)-(Ly_pend.^2.*THE_Psi_D.*m_pend.*cos(THE_Psi_pend).*sin(THE_Psi).*sin(THE_Psi_pend).*sin(THE_Theta_pend))./1.2e+1+(Lz_pend.^2.*THE_Psi_D.*m_pend.*cos(THE_Psi_pend).*sin(THE_Psi).*sin(THE_Psi_pend).*sin(THE_Theta_pend))./3.0+(Ly_pend.^2.*THE_Psi_D.*m_pend.*cos(THE_Phi_pend).*cos(THE_Psi_pend).^2.*cos(THE_Theta_pend).^2.*sin(THE_Psi).*sin(THE_Phi_pend))./1.2e+1-(Lz_pend.^2.*THE_Psi_D.*m_pend.*cos(THE_Phi_pend).*cos(THE_Psi_pend).^2.*cos(THE_Theta_pend).^2.*sin(THE_Psi).*sin(THE_Phi_pend))./3.0+(Lx_pend.^2.*THE_Theta_pend_D.*m_pend.*cos(THE_Psi).*cos(THE_Phi_pend).*cos(THE_Theta_pend).*sin(THE_Phi_pend).*sin(THE_Theta_pend))./6.0-(Ly_pend.^2.*THE_Psi_D.*m_pend.*cos(THE_Psi).*cos(THE_Psi_pend).*cos(THE_Theta_pend).*sin(THE_Phi_pend).*sin(THE_Psi_pend))./1.2e+1-(Ly_pend.^2.*THE_Psi_pend_D.*m_pend.*cos(THE_Psi).*cos(THE_Phi_pend).*cos(THE_Psi_pend).*sin(THE_Phi_pend).*sin(THE_Psi_pend))./3.0;
    et318 = Ly_pend.^2.*THE_Theta_pend_D.*m_pend.*cos(THE_Psi).*cos(THE_Phi_pend).*cos(THE_Theta_pend).*sin(THE_Phi_pend).*sin(THE_Theta_pend).*(-1.0./6.0)+(Lz_pend.^2.*THE_Psi_D.*m_pend.*cos(THE_Psi).*cos(THE_Psi_pend).*cos(THE_Theta_pend).*sin(THE_Phi_pend).*sin(THE_Psi_pend))./3.0+Lz_pend.^2.*THE_Psi_pend_D.*m_pend.*cos(THE_Psi).*cos(THE_Phi_pend).*cos(THE_Psi_pend).*sin(THE_Phi_pend).*sin(THE_Psi_pend).*(4.0./3.0)+(Ly_pend.^2.*THE_Theta_pend_D.*m_pend.*cos(THE_Psi_pend).*sin(THE_Psi).*sin(THE_Phi_pend).*sin(THE_Psi_pend).*sin(THE_Theta_pend))./6.0-Lz_pend.^2.*THE_Theta_pend_D.*m_pend.*cos(THE_Psi_pend).*sin(THE_Psi).*sin(THE_Phi_pend).*sin(THE_Psi_pend).*sin(THE_Theta_pend).*(2.0./3.0)+(Lz_pend.*THE_Psi_D.*Tv_Z_pend.*m_pend.*cos(THE_Psi).*cos(THE_Phi_pend).*cos(THE_Psi_pend).*sin(THE_Theta_pend))./2.0-(Ly_pend.^2.*THE_Psi_D.*m_pend.*cos(THE_Psi).*cos(THE_Phi_pend).*cos(THE_Psi_pend).^2.*cos(THE_Theta_pend).*sin(THE_Theta_pend))./1.2e+1-(Ly_pend.^2.*THE_Theta_pend_D.*m_pend.*cos(THE_Psi).*cos(THE_Phi_pend).^2.*cos(THE_Psi_pend).*cos(THE_Theta_pend).*sin(THE_Psi_pend))./6.0+(Lz_pend.^2.*THE_Psi_D.*m_pend.*cos(THE_Psi).*cos(THE_Phi_pend).*cos(THE_Psi_pend).^2.*cos(THE_Theta_pend).*sin(THE_Theta_pend))./3.0+Lz_pend.^2.*THE_Theta_pend_D.*m_pend.*cos(THE_Psi).*cos(THE_Phi_pend).^2.*cos(THE_Psi_pend).*cos(THE_Theta_pend).*sin(THE_Psi_pend).*(2.0./3.0);
    et319 = (Ly_pend.^2.*THE_Psi_D.*m_pend.*cos(THE_Phi_pend).^2.*cos(THE_Psi_pend).*sin(THE_Psi).*sin(THE_Psi_pend).*sin(THE_Theta_pend))./6.0-Lz_pend.^2.*THE_Psi_D.*m_pend.*cos(THE_Phi_pend).^2.*cos(THE_Psi_pend).*sin(THE_Psi).*sin(THE_Psi_pend).*sin(THE_Theta_pend).*(2.0./3.0)+(Ly_pend.^2.*THE_Phi_pend_D.*m_pend.*cos(THE_Psi).*cos(THE_Phi_pend).*cos(THE_Psi_pend).*sin(THE_Phi_pend).*sin(THE_Psi_pend).*sin(THE_Theta_pend))./3.0+(Ly_pend.^2.*THE_Psi_pend_D.*m_pend.*cos(THE_Phi_pend).*cos(THE_Psi_pend).*cos(THE_Theta_pend).*sin(THE_Psi).*sin(THE_Psi_pend).*sin(THE_Theta_pend))./6.0-Lz_pend.^2.*THE_Phi_pend_D.*m_pend.*cos(THE_Psi).*cos(THE_Phi_pend).*cos(THE_Psi_pend).*sin(THE_Phi_pend).*sin(THE_Psi_pend).*sin(THE_Theta_pend).*(4.0./3.0)-Lz_pend.^2.*THE_Psi_pend_D.*m_pend.*cos(THE_Phi_pend).*cos(THE_Psi_pend).*cos(THE_Theta_pend).*sin(THE_Psi).*sin(THE_Psi_pend).*sin(THE_Theta_pend).*(2.0./3.0)+(Ly_pend.^2.*THE_Psi_pend_D.*m_pend.*cos(THE_Psi).*cos(THE_Phi_pend).*cos(THE_Psi_pend).*cos(THE_Theta_pend).^2.*sin(THE_Phi_pend).*sin(THE_Psi_pend))./6.0+(Ly_pend.^2.*THE_Theta_pend_D.*m_pend.*cos(THE_Psi).*cos(THE_Phi_pend).*cos(THE_Psi_pend).^2.*cos(THE_Theta_pend).*sin(THE_Phi_pend).*sin(THE_Theta_pend))./6.0-Lz_pend.^2.*THE_Psi_pend_D.*m_pend.*cos(THE_Psi).*cos(THE_Phi_pend).*cos(THE_Psi_pend).*cos(THE_Theta_pend).^2.*sin(THE_Phi_pend).*sin(THE_Psi_pend).*(2.0./3.0);
    et320 = Lz_pend.^2.*THE_Theta_pend_D.*m_pend.*cos(THE_Psi).*cos(THE_Phi_pend).*cos(THE_Psi_pend).^2.*cos(THE_Theta_pend).*sin(THE_Phi_pend).*sin(THE_Theta_pend).*(-2.0./3.0);
    et321 = I_xy.*THE_Psi_D.*cos(THE_Psi).*cos(THE_Theta)+Iprop_xy.*THE_Psi_D.*cos(THE_Psi).*cos(THE_Theta).*4.0-I_xz.*THE_Psi_D.*cos(THE_Theta).*sin(THE_Psi)-Iprop_xz.*THE_Psi_D.*cos(THE_Theta).*sin(THE_Psi).*4.0+Iprop_yz.*wMOT_1.*cos(THE_Psi).*cos(THE_Theta)+Iprop_yz.*wMOT_2.*cos(THE_Psi).*cos(THE_Theta)+Iprop_yz.*wMOT_3.*cos(THE_Psi).*cos(THE_Theta)+Iprop_yz.*wMOT_4.*cos(THE_Psi).*cos(THE_Theta)-Iprop_zz.*wMOT_1.*cos(THE_Theta).*sin(THE_Psi)-Iprop_zz.*wMOT_2.*cos(THE_Theta).*sin(THE_Psi)-Iprop_zz.*wMOT_3.*cos(THE_Theta).*sin(THE_Psi)-Iprop_zz.*wMOT_4.*cos(THE_Theta).*sin(THE_Psi)-Lz_pend.^2.*THE_Phi_pend_D.*m_pend.*cos(THE_Theta).*sin(THE_Psi).*(2.0./3.0)-(Ly_pend.^2.*THE_Phi_pend_D.*m_pend.*cos(THE_Phi_pend).*sin(THE_Theta).*sin(THE_Phi_pend))./6.0-(Ly_pend.^2.*THE_Psi_pend_D.*m_pend.*cos(THE_Psi_pend).*sin(THE_Theta).*sin(THE_Psi_pend))./6.0+Lz_pend.^2.*THE_Psi_pend_D.*m_pend.*cos(THE_Theta).*sin(THE_Psi).*sin(THE_Theta_pend).*(2.0./3.0)+Lz_pend.^2.*THE_Phi_pend_D.*m_pend.*cos(THE_Phi_pend).*sin(THE_Theta).*sin(THE_Phi_pend).*(2.0./3.0)+Lz_pend.^2.*THE_Psi_pend_D.*m_pend.*cos(THE_Psi_pend).*sin(THE_Theta).*sin(THE_Psi_pend).*(2.0./3.0);
    et322 = Ly_pend.^2.*THE_Phi_pend_D.*m_pend.*cos(THE_Theta).*cos(THE_Phi_pend).^2.*sin(THE_Psi).*(-1.0./6.0)-(Ly_pend.^2.*THE_Phi_pend_D.*m_pend.*cos(THE_Theta).*cos(THE_Psi_pend).^2.*sin(THE_Psi))./6.0+Lz_pend.^2.*THE_Phi_pend_D.*m_pend.*cos(THE_Theta).*cos(THE_Phi_pend).^2.*sin(THE_Psi).*(2.0./3.0)+Lz_pend.^2.*THE_Phi_pend_D.*m_pend.*cos(THE_Theta).*cos(THE_Psi_pend).^2.*sin(THE_Psi).*(2.0./3.0)+(Ly_pend.^2.*THE_Theta_pend_D.*m_pend.*cos(THE_Psi).*cos(THE_Theta).*cos(THE_Phi_pend))./6.0+Lz_pend.*THE_Psi_pend_D.*Tv_Z_pend.*m_pend.*cos(THE_Theta_pend).*sin(THE_Theta).*sin(THE_Psi_pend)+Lz_pend.*THE_Theta_pend_D.*Tv_Z_pend.*m_pend.*cos(THE_Psi_pend).*sin(THE_Theta).*sin(THE_Theta_pend)+(Lx_pend.^2.*THE_Theta_pend_D.*m_pend.*cos(THE_Psi).*cos(THE_Theta).*cos(THE_Phi_pend).*cos(THE_Theta_pend).^2)./6.0-(Ly_pend.^2.*THE_Theta_pend_D.*m_pend.*cos(THE_Psi).*cos(THE_Theta).*cos(THE_Phi_pend).*cos(THE_Psi_pend).^2)./6.0-(Ly_pend.^2.*THE_Theta_pend_D.*m_pend.*cos(THE_Psi).*cos(THE_Theta).*cos(THE_Phi_pend).*cos(THE_Theta_pend).^2)./6.0+Lz_pend.^2.*THE_Theta_pend_D.*m_pend.*cos(THE_Psi).*cos(THE_Theta).*cos(THE_Phi_pend).*cos(THE_Psi_pend).^2.*(2.0./3.0);
    et323 = Lx_pend.^2.*THE_Phi_pend_D.*m_pend.*cos(THE_Phi_pend).*cos(THE_Theta_pend).^2.*sin(THE_Theta).*sin(THE_Phi_pend).*(-1.0./6.0)-(Lx_pend.^2.*THE_Theta_pend_D.*m_pend.*cos(THE_Phi_pend).^2.*cos(THE_Theta_pend).*sin(THE_Theta).*sin(THE_Theta_pend))./6.0+(Ly_pend.^2.*THE_Psi_pend_D.*m_pend.*cos(THE_Theta).*cos(THE_Phi_pend).^2.*sin(THE_Psi).*sin(THE_Theta_pend))./6.0+(Ly_pend.^2.*THE_Psi_pend_D.*m_pend.*cos(THE_Theta).*cos(THE_Psi_pend).^2.*sin(THE_Psi).*sin(THE_Theta_pend))./6.0+(Ly_pend.^2.*THE_Phi_pend_D.*m_pend.*cos(THE_Phi_pend).*cos(THE_Psi_pend).^2.*sin(THE_Theta).*sin(THE_Phi_pend))./3.0+(Ly_pend.^2.*THE_Psi_pend_D.*m_pend.*cos(THE_Phi_pend).^2.*cos(THE_Psi_pend).*sin(THE_Theta).*sin(THE_Psi_pend))./3.0+(Ly_pend.^2.*THE_Phi_pend_D.*m_pend.*cos(THE_Phi_pend).*cos(THE_Theta_pend).^2.*sin(THE_Theta).*sin(THE_Phi_pend))./6.0+(Ly_pend.^2.*THE_Theta_pend_D.*m_pend.*cos(THE_Phi_pend).^2.*cos(THE_Theta_pend).*sin(THE_Theta).*sin(THE_Theta_pend))./6.0-Lz_pend.^2.*THE_Psi_pend_D.*m_pend.*cos(THE_Theta).*cos(THE_Phi_pend).^2.*sin(THE_Psi).*sin(THE_Theta_pend).*(2.0./3.0)-Lz_pend.^2.*THE_Psi_pend_D.*m_pend.*cos(THE_Theta).*cos(THE_Psi_pend).^2.*sin(THE_Psi).*sin(THE_Theta_pend).*(2.0./3.0);
    et324 = Lz_pend.^2.*THE_Phi_pend_D.*m_pend.*cos(THE_Phi_pend).*cos(THE_Psi_pend).^2.*sin(THE_Theta).*sin(THE_Phi_pend).*(-4.0./3.0)-Lz_pend.^2.*THE_Psi_pend_D.*m_pend.*cos(THE_Phi_pend).^2.*cos(THE_Psi_pend).*sin(THE_Theta).*sin(THE_Psi_pend).*(4.0./3.0)-(Lx_pend.^2.*THE_Phi_pend_D.*m_pend.*cos(THE_Theta).*cos(THE_Phi_pend).^2.*cos(THE_Theta_pend).^2.*sin(THE_Psi))./6.0+(Ly_pend.^2.*THE_Phi_pend_D.*m_pend.*cos(THE_Theta).*cos(THE_Phi_pend).^2.*cos(THE_Psi_pend).^2.*sin(THE_Psi))./3.0+(Ly_pend.^2.*THE_Phi_pend_D.*m_pend.*cos(THE_Theta).*cos(THE_Phi_pend).^2.*cos(THE_Theta_pend).^2.*sin(THE_Psi))./6.0-Lz_pend.^2.*THE_Phi_pend_D.*m_pend.*cos(THE_Theta).*cos(THE_Phi_pend).^2.*cos(THE_Psi_pend).^2.*sin(THE_Psi).*(4.0./3.0)-(Ly_pend.^2.*THE_Psi_D.*m_pend.*cos(THE_Psi).*cos(THE_Theta).*cos(THE_Phi_pend).*sin(THE_Phi_pend))./1.2e+1+(Lz_pend.^2.*THE_Psi_D.*m_pend.*cos(THE_Psi).*cos(THE_Theta).*cos(THE_Phi_pend).*sin(THE_Phi_pend))./3.0+Lz_pend.^2.*THE_Psi_pend_D.*m_pend.*cos(THE_Psi).*cos(THE_Theta).*cos(THE_Theta_pend).*sin(THE_Phi_pend).*(2.0./3.0)+(Ly_pend.^2.*THE_Psi_pend_D.*m_pend.*cos(THE_Phi_pend).*sin(THE_Theta).*sin(THE_Phi_pend).*sin(THE_Theta_pend))./6.0;
    et325 = (Ly_pend.^2.*THE_Phi_pend_D.*m_pend.*cos(THE_Psi_pend).*sin(THE_Theta).*sin(THE_Psi_pend).*sin(THE_Theta_pend))./6.0-Lz_pend.^2.*THE_Psi_pend_D.*m_pend.*cos(THE_Phi_pend).*sin(THE_Theta).*sin(THE_Phi_pend).*sin(THE_Theta_pend).*(2.0./3.0)-Lz_pend.^2.*THE_Phi_pend_D.*m_pend.*cos(THE_Psi_pend).*sin(THE_Theta).*sin(THE_Psi_pend).*sin(THE_Theta_pend).*(2.0./3.0)+(Ly_pend.^2.*THE_Theta_pend_D.*m_pend.*cos(THE_Psi).*cos(THE_Theta).*cos(THE_Phi_pend).*cos(THE_Psi_pend).^2.*cos(THE_Theta_pend).^2)./6.0-Lz_pend.^2.*THE_Theta_pend_D.*m_pend.*cos(THE_Psi).*cos(THE_Theta).*cos(THE_Phi_pend).*cos(THE_Psi_pend).^2.*cos(THE_Theta_pend).^2.*(2.0./3.0)-(Ly_pend.^2.*THE_Psi_pend_D.*m_pend.*cos(THE_Theta).*cos(THE_Phi_pend).^2.*cos(THE_Psi_pend).^2.*sin(THE_Psi).*sin(THE_Theta_pend))./3.0-(Ly_pend.^2.*THE_Phi_pend_D.*m_pend.*cos(THE_Phi_pend).*cos(THE_Psi_pend).^2.*cos(THE_Theta_pend).^2.*sin(THE_Theta).*sin(THE_Phi_pend))./6.0-(Ly_pend.^2.*THE_Psi_pend_D.*m_pend.*cos(THE_Phi_pend).^2.*cos(THE_Psi_pend).*cos(THE_Theta_pend).^2.*sin(THE_Theta).*sin(THE_Psi_pend))./6.0-(Ly_pend.^2.*THE_Theta_pend_D.*m_pend.*cos(THE_Phi_pend).^2.*cos(THE_Psi_pend).^2.*cos(THE_Theta_pend).*sin(THE_Theta).*sin(THE_Theta_pend))./6.0;
    et326 = Lz_pend.^2.*THE_Psi_pend_D.*m_pend.*cos(THE_Theta).*cos(THE_Phi_pend).^2.*cos(THE_Psi_pend).^2.*sin(THE_Psi).*sin(THE_Theta_pend).*(4.0./3.0)+Lz_pend.^2.*THE_Phi_pend_D.*m_pend.*cos(THE_Phi_pend).*cos(THE_Psi_pend).^2.*cos(THE_Theta_pend).^2.*sin(THE_Theta).*sin(THE_Phi_pend).*(2.0./3.0)+Lz_pend.^2.*THE_Psi_pend_D.*m_pend.*cos(THE_Phi_pend).^2.*cos(THE_Psi_pend).*cos(THE_Theta_pend).^2.*sin(THE_Theta).*sin(THE_Psi_pend).*(2.0./3.0)+Lz_pend.^2.*THE_Theta_pend_D.*m_pend.*cos(THE_Phi_pend).^2.*cos(THE_Psi_pend).^2.*cos(THE_Theta_pend).*sin(THE_Theta).*sin(THE_Theta_pend).*(2.0./3.0)-(Lx_pend.^2.*THE_Psi_D.*m_pend.*cos(THE_Theta).*cos(THE_Phi_pend).*cos(THE_Theta_pend).*sin(THE_Psi).*sin(THE_Theta_pend))./1.2e+1+(Ly_pend.^2.*THE_Psi_D.*m_pend.*cos(THE_Psi).*cos(THE_Theta).*cos(THE_Psi_pend).*sin(THE_Psi_pend).*sin(THE_Theta_pend))./1.2e+1+(Ly_pend.^2.*THE_Psi_D.*m_pend.*cos(THE_Theta).*cos(THE_Phi_pend).*cos(THE_Theta_pend).*sin(THE_Psi).*sin(THE_Theta_pend))./1.2e+1+(Ly_pend.^2.*THE_Theta_pend_D.*m_pend.*cos(THE_Theta).*cos(THE_Psi_pend).*cos(THE_Theta_pend).*sin(THE_Psi).*sin(THE_Psi_pend))./6.0-(Lz_pend.^2.*THE_Psi_D.*m_pend.*cos(THE_Psi).*cos(THE_Theta).*cos(THE_Psi_pend).*sin(THE_Psi_pend).*sin(THE_Theta_pend))./3.0;
    et327 = Lz_pend.^2.*THE_Theta_pend_D.*m_pend.*cos(THE_Theta).*cos(THE_Psi_pend).*cos(THE_Theta_pend).*sin(THE_Psi).*sin(THE_Psi_pend).*(-2.0./3.0)-(Ly_pend.^2.*THE_Phi_pend_D.*m_pend.*cos(THE_Theta).*cos(THE_Phi_pend).^2.*cos(THE_Psi_pend).^2.*cos(THE_Theta_pend).^2.*sin(THE_Psi))./6.0+Lz_pend.^2.*THE_Phi_pend_D.*m_pend.*cos(THE_Theta).*cos(THE_Phi_pend).^2.*cos(THE_Psi_pend).^2.*cos(THE_Theta_pend).^2.*sin(THE_Psi).*(2.0./3.0)+(Lz_pend.*THE_Psi_D.*Tv_Z_pend.*m_pend.*cos(THE_Theta).*sin(THE_Psi).*sin(THE_Phi_pend).*sin(THE_Psi_pend))./2.0-(Lx_pend.^2.*THE_Psi_D.*m_pend.*cos(THE_Psi).*cos(THE_Theta).*cos(THE_Phi_pend).*cos(THE_Theta_pend).^2.*sin(THE_Phi_pend))./1.2e+1+(Ly_pend.^2.*THE_Psi_D.*m_pend.*cos(THE_Psi).*cos(THE_Theta).*cos(THE_Phi_pend).*cos(THE_Psi_pend).^2.*sin(THE_Phi_pend))./6.0+(Ly_pend.^2.*THE_Psi_D.*m_pend.*cos(THE_Psi).*cos(THE_Theta).*cos(THE_Phi_pend).*cos(THE_Theta_pend).^2.*sin(THE_Phi_pend))./1.2e+1+(Ly_pend.^2.*THE_Psi_pend_D.*m_pend.*cos(THE_Psi).*cos(THE_Theta).*cos(THE_Psi_pend).^2.*cos(THE_Theta_pend).*sin(THE_Phi_pend))./6.0-Lz_pend.^2.*THE_Psi_D.*m_pend.*cos(THE_Psi).*cos(THE_Theta).*cos(THE_Phi_pend).*cos(THE_Psi_pend).^2.*sin(THE_Phi_pend).*(2.0./3.0);
    et328 = Lz_pend.^2.*THE_Psi_pend_D.*m_pend.*cos(THE_Psi).*cos(THE_Theta).*cos(THE_Psi_pend).^2.*cos(THE_Theta_pend).*sin(THE_Phi_pend).*(-2.0./3.0)-(Ly_pend.^2.*THE_Phi_pend_D.*m_pend.*cos(THE_Phi_pend).^2.*cos(THE_Psi_pend).*sin(THE_Theta).*sin(THE_Psi_pend).*sin(THE_Theta_pend))./3.0-(Ly_pend.^2.*THE_Psi_pend_D.*m_pend.*cos(THE_Phi_pend).*cos(THE_Psi_pend).^2.*sin(THE_Theta).*sin(THE_Phi_pend).*sin(THE_Theta_pend))./3.0+Lz_pend.^2.*THE_Phi_pend_D.*m_pend.*cos(THE_Phi_pend).^2.*cos(THE_Psi_pend).*sin(THE_Theta).*sin(THE_Psi_pend).*sin(THE_Theta_pend).*(4.0./3.0)+Lz_pend.^2.*THE_Psi_pend_D.*m_pend.*cos(THE_Phi_pend).*cos(THE_Psi_pend).^2.*sin(THE_Theta).*sin(THE_Phi_pend).*sin(THE_Theta_pend).*(4.0./3.0)+(Lx_pend.^2.*THE_Theta_pend_D.*m_pend.*cos(THE_Theta).*cos(THE_Phi_pend).*cos(THE_Theta_pend).*sin(THE_Psi).*sin(THE_Phi_pend).*sin(THE_Theta_pend))./6.0-(Ly_pend.^2.*THE_Psi_D.*m_pend.*cos(THE_Theta).*cos(THE_Psi_pend).*cos(THE_Theta_pend).*sin(THE_Psi).*sin(THE_Phi_pend).*sin(THE_Psi_pend))./1.2e+1-(Ly_pend.^2.*THE_Psi_pend_D.*m_pend.*cos(THE_Theta).*cos(THE_Phi_pend).*cos(THE_Psi_pend).*sin(THE_Psi).*sin(THE_Phi_pend).*sin(THE_Psi_pend))./3.0-(Ly_pend.^2.*THE_Theta_pend_D.*m_pend.*cos(THE_Psi).*cos(THE_Theta).*cos(THE_Psi_pend).*sin(THE_Phi_pend).*sin(THE_Psi_pend).*sin(THE_Theta_pend))./6.0;
    et329 = Ly_pend.^2.*THE_Theta_pend_D.*m_pend.*cos(THE_Theta).*cos(THE_Phi_pend).*cos(THE_Theta_pend).*sin(THE_Psi).*sin(THE_Phi_pend).*sin(THE_Theta_pend).*(-1.0./6.0)-(Ly_pend.^2.*THE_Theta_pend_D.*m_pend.*cos(THE_Phi_pend).*cos(THE_Psi_pend).*cos(THE_Theta_pend).*sin(THE_Theta).*sin(THE_Phi_pend).*sin(THE_Psi_pend))./6.0+(Lz_pend.^2.*THE_Psi_D.*m_pend.*cos(THE_Theta).*cos(THE_Psi_pend).*cos(THE_Theta_pend).*sin(THE_Psi).*sin(THE_Phi_pend).*sin(THE_Psi_pend))./3.0+Lz_pend.^2.*THE_Psi_pend_D.*m_pend.*cos(THE_Theta).*cos(THE_Phi_pend).*cos(THE_Psi_pend).*sin(THE_Psi).*sin(THE_Phi_pend).*sin(THE_Psi_pend).*(4.0./3.0)+Lz_pend.^2.*THE_Theta_pend_D.*m_pend.*cos(THE_Psi).*cos(THE_Theta).*cos(THE_Psi_pend).*sin(THE_Phi_pend).*sin(THE_Psi_pend).*sin(THE_Theta_pend).*(2.0./3.0)+Lz_pend.^2.*THE_Theta_pend_D.*m_pend.*cos(THE_Phi_pend).*cos(THE_Psi_pend).*cos(THE_Theta_pend).*sin(THE_Theta).*sin(THE_Phi_pend).*sin(THE_Psi_pend).*(2.0./3.0)+(Lz_pend.*THE_Psi_D.*Tv_Z_pend.*m_pend.*cos(THE_Theta).*cos(THE_Phi_pend).*cos(THE_Psi_pend).*sin(THE_Psi).*sin(THE_Theta_pend))./2.0-(Ly_pend.^2.*THE_Psi_D.*m_pend.*cos(THE_Psi).*cos(THE_Theta).*cos(THE_Phi_pend).^2.*cos(THE_Psi_pend).*sin(THE_Psi_pend).*sin(THE_Theta_pend))./6.0-(Ly_pend.^2.*THE_Psi_D.*m_pend.*cos(THE_Theta).*cos(THE_Phi_pend).*cos(THE_Psi_pend).^2.*cos(THE_Theta_pend).*sin(THE_Psi).*sin(THE_Theta_pend))./1.2e+1;
    et330 = Ly_pend.^2.*THE_Theta_pend_D.*m_pend.*cos(THE_Theta).*cos(THE_Phi_pend).^2.*cos(THE_Psi_pend).*cos(THE_Theta_pend).*sin(THE_Psi).*sin(THE_Psi_pend).*(-1.0./6.0)+Lz_pend.^2.*THE_Psi_D.*m_pend.*cos(THE_Psi).*cos(THE_Theta).*cos(THE_Phi_pend).^2.*cos(THE_Psi_pend).*sin(THE_Psi_pend).*sin(THE_Theta_pend).*(2.0./3.0)+(Lz_pend.^2.*THE_Psi_D.*m_pend.*cos(THE_Theta).*cos(THE_Phi_pend).*cos(THE_Psi_pend).^2.*cos(THE_Theta_pend).*sin(THE_Psi).*sin(THE_Theta_pend))./3.0+Lz_pend.^2.*THE_Theta_pend_D.*m_pend.*cos(THE_Theta).*cos(THE_Phi_pend).^2.*cos(THE_Psi_pend).*cos(THE_Theta_pend).*sin(THE_Psi).*sin(THE_Psi_pend).*(2.0./3.0)-(Ly_pend.^2.*THE_Psi_D.*m_pend.*cos(THE_Psi).*cos(THE_Theta).*cos(THE_Phi_pend).*cos(THE_Psi_pend).^2.*cos(THE_Theta_pend).^2.*sin(THE_Phi_pend))./1.2e+1+(Lz_pend.^2.*THE_Psi_D.*m_pend.*cos(THE_Psi).*cos(THE_Theta).*cos(THE_Phi_pend).*cos(THE_Psi_pend).^2.*cos(THE_Theta_pend).^2.*sin(THE_Phi_pend))./3.0+(Ly_pend.^2.*THE_Phi_pend_D.*m_pend.*cos(THE_Theta).*cos(THE_Phi_pend).*cos(THE_Psi_pend).*sin(THE_Psi).*sin(THE_Phi_pend).*sin(THE_Psi_pend).*sin(THE_Theta_pend))./3.0-Lz_pend.^2.*THE_Phi_pend_D.*m_pend.*cos(THE_Theta).*cos(THE_Phi_pend).*cos(THE_Psi_pend).*sin(THE_Psi).*sin(THE_Phi_pend).*sin(THE_Psi_pend).*sin(THE_Theta_pend).*(4.0./3.0);
    et331 = (Ly_pend.^2.*THE_Psi_pend_D.*m_pend.*cos(THE_Theta).*cos(THE_Phi_pend).*cos(THE_Psi_pend).*cos(THE_Theta_pend).^2.*sin(THE_Psi).*sin(THE_Phi_pend).*sin(THE_Psi_pend))./6.0+(Ly_pend.^2.*THE_Theta_pend_D.*m_pend.*cos(THE_Theta).*cos(THE_Phi_pend).*cos(THE_Psi_pend).^2.*cos(THE_Theta_pend).*sin(THE_Psi).*sin(THE_Phi_pend).*sin(THE_Theta_pend))./6.0-Lz_pend.^2.*THE_Psi_pend_D.*m_pend.*cos(THE_Theta).*cos(THE_Phi_pend).*cos(THE_Psi_pend).*cos(THE_Theta_pend).^2.*sin(THE_Psi).*sin(THE_Phi_pend).*sin(THE_Psi_pend).*(2.0./3.0)-Lz_pend.^2.*THE_Theta_pend_D.*m_pend.*cos(THE_Theta).*cos(THE_Phi_pend).*cos(THE_Psi_pend).^2.*cos(THE_Theta_pend).*sin(THE_Psi).*sin(THE_Phi_pend).*sin(THE_Theta_pend).*(2.0./3.0)-(Ly_pend.^2.*THE_Psi_pend_D.*m_pend.*cos(THE_Psi).*cos(THE_Theta).*cos(THE_Phi_pend).*cos(THE_Psi_pend).*cos(THE_Theta_pend).*sin(THE_Psi_pend).*sin(THE_Theta_pend))./6.0+Lz_pend.^2.*THE_Psi_pend_D.*m_pend.*cos(THE_Psi).*cos(THE_Theta).*cos(THE_Phi_pend).*cos(THE_Psi_pend).*cos(THE_Theta_pend).*sin(THE_Psi_pend).*sin(THE_Theta_pend).*(2.0./3.0);
    et332 = Lz_pend.*m_pend;
    et333 = THE_Phi_pend_D.*cos(THE_Phi).*cos(THE_Psi).*cos(THE_Phi_pend).*sin(THE_Psi_pend)+THE_Psi_pend_D.*cos(THE_Phi).*cos(THE_Psi).*cos(THE_Psi_pend).*sin(THE_Phi_pend).*2.0+THE_Psi_pend_D.*cos(THE_Theta).*cos(THE_Phi_pend).*cos(THE_Psi_pend).*sin(THE_Phi).*2.0-THE_Phi_pend_D.*cos(THE_Theta).*sin(THE_Phi).*sin(THE_Phi_pend).*sin(THE_Psi_pend)+THE_Theta_pend_D.*cos(THE_Phi).*cos(THE_Psi).*cos(THE_Phi_pend).*cos(THE_Psi_pend).*cos(THE_Theta_pend).*2.0-THE_Phi_pend_D.*cos(THE_Phi).*cos(THE_Psi).*cos(THE_Psi_pend).*sin(THE_Phi_pend).*sin(THE_Theta_pend)-THE_Psi_pend_D.*cos(THE_Phi).*cos(THE_Psi).*cos(THE_Phi_pend).*sin(THE_Psi_pend).*sin(THE_Theta_pend).*2.0-THE_Phi_pend_D.*cos(THE_Theta).*cos(THE_Phi_pend).*cos(THE_Psi_pend).*sin(THE_Phi).*sin(THE_Theta_pend)-THE_Theta_pend_D.*cos(THE_Theta).*cos(THE_Psi_pend).*cos(THE_Theta_pend).*sin(THE_Phi).*sin(THE_Phi_pend).*2.0+THE_Phi_pend_D.*cos(THE_Phi_pend).*sin(THE_Phi).*sin(THE_Psi).*sin(THE_Theta).*sin(THE_Psi_pend)+THE_Psi_pend_D.*cos(THE_Psi_pend).*sin(THE_Phi).*sin(THE_Psi).*sin(THE_Theta).*sin(THE_Phi_pend).*2.0+THE_Psi_pend_D.*cos(THE_Theta).*sin(THE_Phi).*sin(THE_Phi_pend).*sin(THE_Psi_pend).*sin(THE_Theta_pend).*2.0+THE_Theta_pend_D.*cos(THE_Phi_pend).*cos(THE_Psi_pend).*cos(THE_Theta_pend).*sin(THE_Phi).*sin(THE_Psi).*sin(THE_Theta).*2.0-THE_Phi_pend_D.*cos(THE_Psi_pend).*sin(THE_Phi).*sin(THE_Psi).*sin(THE_Theta).*sin(THE_Phi_pend).*sin(THE_Theta_pend)-THE_Psi_pend_D.*cos(THE_Phi_pend).*sin(THE_Phi).*sin(THE_Psi).*sin(THE_Theta).*sin(THE_Psi_pend).*sin(THE_Theta_pend).*2.0;
    et334 = 1.0./2.0;
    et335 = Lz_pend.*m_pend.*(THE_Psi_pend_D.*cos(THE_Phi).*cos(THE_Theta).*cos(THE_Phi_pend).*cos(THE_Psi_pend).*-2.0+THE_Phi_pend_D.*cos(THE_Psi).*cos(THE_Phi_pend).*sin(THE_Phi).*sin(THE_Psi_pend)+THE_Psi_pend_D.*cos(THE_Psi).*cos(THE_Psi_pend).*sin(THE_Phi).*sin(THE_Phi_pend).*2.0+THE_Phi_pend_D.*cos(THE_Phi).*cos(THE_Theta).*sin(THE_Phi_pend).*sin(THE_Psi_pend)+THE_Phi_pend_D.*cos(THE_Phi).*cos(THE_Theta).*cos(THE_Phi_pend).*cos(THE_Psi_pend).*sin(THE_Theta_pend)+THE_Theta_pend_D.*cos(THE_Psi).*cos(THE_Phi_pend).*cos(THE_Psi_pend).*cos(THE_Theta_pend).*sin(THE_Phi).*2.0+THE_Theta_pend_D.*cos(THE_Phi).*cos(THE_Theta).*cos(THE_Psi_pend).*cos(THE_Theta_pend).*sin(THE_Phi_pend).*2.0-THE_Phi_pend_D.*cos(THE_Phi).*cos(THE_Phi_pend).*sin(THE_Psi).*sin(THE_Theta).*sin(THE_Psi_pend)-THE_Psi_pend_D.*cos(THE_Phi).*cos(THE_Psi_pend).*sin(THE_Psi).*sin(THE_Theta).*sin(THE_Phi_pend).*2.0-THE_Phi_pend_D.*cos(THE_Psi).*cos(THE_Psi_pend).*sin(THE_Phi).*sin(THE_Phi_pend).*sin(THE_Theta_pend)-THE_Psi_pend_D.*cos(THE_Psi).*cos(THE_Phi_pend).*sin(THE_Phi).*sin(THE_Psi_pend).*sin(THE_Theta_pend).*2.0-THE_Psi_pend_D.*cos(THE_Phi).*cos(THE_Theta).*sin(THE_Phi_pend).*sin(THE_Psi_pend).*sin(THE_Theta_pend).*2.0-THE_Theta_pend_D.*cos(THE_Phi).*cos(THE_Phi_pend).*cos(THE_Psi_pend).*cos(THE_Theta_pend).*sin(THE_Psi).*sin(THE_Theta).*2.0+THE_Phi_pend_D.*cos(THE_Phi).*cos(THE_Psi_pend).*sin(THE_Psi).*sin(THE_Theta).*sin(THE_Phi_pend).*sin(THE_Theta_pend)+THE_Psi_pend_D.*cos(THE_Phi).*cos(THE_Phi_pend).*sin(THE_Psi).*sin(THE_Theta).*sin(THE_Psi_pend).*sin(THE_Theta_pend).*2.0);
    et336 = -1.0./2.0;
    et337 = Lx_pend.^2.*THE_Theta_pend_D.*m_pend.*cos(THE_Phi_pend).*(-1.0./6.0)-(Ly_pend.^2.*THE_Psi_pend_D.*m_pend.*cos(THE_Theta_pend).*sin(THE_Phi_pend))./6.0+(Lx_pend.^2.*THE_Theta_pend_D.*m_pend.*cos(THE_Phi_pend).*cos(THE_Theta_pend).^2)./6.0-(Ly_pend.^2.*THE_Theta_pend_D.*m_pend.*cos(THE_Phi_pend).*cos(THE_Theta_pend).^2)./6.0-(Lx_pend.^2.*THE_Phi_pend_D.*m_pend.*cos(THE_Theta_pend).*sin(THE_Phi_pend).*sin(THE_Theta_pend))./1.2e+1+(Ly_pend.^2.*THE_Phi_pend_D.*m_pend.*cos(THE_Theta_pend).*sin(THE_Phi_pend).*sin(THE_Theta_pend))./1.2e+1-(Lz_pend.*THE_Phi_pend_D.*Tv_Z_pend.*m_pend.*cos(THE_Phi_pend).*sin(THE_Psi_pend))./2.0-Lz_pend.*THE_Psi_pend_D.*Tv_Z_pend.*m_pend.*cos(THE_Psi_pend).*sin(THE_Phi_pend)+(Ly_pend.^2.*THE_Psi_pend_D.*m_pend.*cos(THE_Psi_pend).^2.*cos(THE_Theta_pend).*sin(THE_Phi_pend))./6.0-Lz_pend.^2.*THE_Psi_pend_D.*m_pend.*cos(THE_Psi_pend).^2.*cos(THE_Theta_pend).*sin(THE_Phi_pend).*(2.0./3.0)+(Ly_pend.^2.*THE_Theta_pend_D.*m_pend.*cos(THE_Phi_pend).*cos(THE_Psi_pend).^2.*cos(THE_Theta_pend).^2)./6.0-Lz_pend.^2.*THE_Theta_pend_D.*m_pend.*cos(THE_Phi_pend).*cos(THE_Psi_pend).^2.*cos(THE_Theta_pend).^2.*(2.0./3.0);
    et338 = (Lz_pend.*THE_Phi_pend_D.*Tv_Z_pend.*m_pend.*cos(THE_Psi_pend).*sin(THE_Phi_pend).*sin(THE_Theta_pend))./2.0+Lz_pend.*THE_Psi_pend_D.*Tv_Z_pend.*m_pend.*cos(THE_Phi_pend).*sin(THE_Psi_pend).*sin(THE_Theta_pend)-(Ly_pend.^2.*THE_Phi_pend_D.*m_pend.*cos(THE_Psi_pend).^2.*cos(THE_Theta_pend).*sin(THE_Phi_pend).*sin(THE_Theta_pend))./1.2e+1+(Lz_pend.^2.*THE_Phi_pend_D.*m_pend.*cos(THE_Psi_pend).^2.*cos(THE_Theta_pend).*sin(THE_Phi_pend).*sin(THE_Theta_pend))./3.0+(Ly_pend.^2.*THE_Phi_pend_D.*m_pend.*cos(THE_Phi_pend).*cos(THE_Psi_pend).*cos(THE_Theta_pend).*sin(THE_Psi_pend))./1.2e+1-(Lz_pend.^2.*THE_Phi_pend_D.*m_pend.*cos(THE_Phi_pend).*cos(THE_Psi_pend).*cos(THE_Theta_pend).*sin(THE_Psi_pend))./3.0-Lz_pend.*THE_Theta_pend_D.*Tv_Z_pend.*m_pend.*cos(THE_Phi_pend).*cos(THE_Psi_pend).*cos(THE_Theta_pend)-(Ly_pend.^2.*THE_Psi_pend_D.*m_pend.*cos(THE_Phi_pend).*cos(THE_Psi_pend).*cos(THE_Theta_pend).*sin(THE_Psi_pend).*sin(THE_Theta_pend))./6.0+Lz_pend.^2.*THE_Psi_pend_D.*m_pend.*cos(THE_Phi_pend).*cos(THE_Psi_pend).*cos(THE_Theta_pend).*sin(THE_Psi_pend).*sin(THE_Theta_pend).*(2.0./3.0);
    et339 = Lx_pend.^2.*THE_Theta_pend_D.*m_pend.*cos(THE_Psi).*sin(THE_Phi_pend).*(-1.0./6.0)+(Lx_pend.^2.*THE_Theta_pend_D.*m_pend.*cos(THE_Theta_pend).*sin(THE_Psi).*sin(THE_Theta_pend))./6.0-(Ly_pend.^2.*THE_Theta_pend_D.*m_pend.*cos(THE_Theta_pend).*sin(THE_Psi).*sin(THE_Theta_pend))./6.0+(Lx_pend.^2.*THE_Theta_pend_D.*m_pend.*cos(THE_Psi).*cos(THE_Theta_pend).^2.*sin(THE_Phi_pend))./6.0-(Ly_pend.^2.*THE_Theta_pend_D.*m_pend.*cos(THE_Psi).*cos(THE_Theta_pend).^2.*sin(THE_Phi_pend))./6.0+(Ly_pend.^2.*THE_Psi_pend_D.*m_pend.*cos(THE_Psi).*cos(THE_Phi_pend).*cos(THE_Theta_pend))./6.0-(Lz_pend.*THE_Phi_pend_D.*Tv_Z_pend.*m_pend.*cos(THE_Psi).*sin(THE_Phi_pend).*sin(THE_Psi_pend))./2.0-(Ly_pend.^2.*THE_Psi_pend_D.*m_pend.*cos(THE_Psi).*cos(THE_Phi_pend).*cos(THE_Psi_pend).^2.*cos(THE_Theta_pend))./6.0+Lz_pend.^2.*THE_Psi_pend_D.*m_pend.*cos(THE_Psi).*cos(THE_Phi_pend).*cos(THE_Psi_pend).^2.*cos(THE_Theta_pend).*(2.0./3.0)+(Ly_pend.^2.*THE_Psi_pend_D.*m_pend.*cos(THE_Psi_pend).*cos(THE_Theta_pend).^2.*sin(THE_Psi).*sin(THE_Psi_pend))./6.0+(Ly_pend.^2.*THE_Theta_pend_D.*m_pend.*cos(THE_Psi_pend).^2.*cos(THE_Theta_pend).*sin(THE_Psi).*sin(THE_Theta_pend))./6.0;
    et340 = Lz_pend.^2.*THE_Psi_pend_D.*m_pend.*cos(THE_Psi_pend).*cos(THE_Theta_pend).^2.*sin(THE_Psi).*sin(THE_Psi_pend).*(-2.0./3.0)-Lz_pend.^2.*THE_Theta_pend_D.*m_pend.*cos(THE_Psi_pend).^2.*cos(THE_Theta_pend).*sin(THE_Psi).*sin(THE_Theta_pend).*(2.0./3.0)+(Ly_pend.^2.*THE_Theta_pend_D.*m_pend.*cos(THE_Psi).*cos(THE_Psi_pend).^2.*cos(THE_Theta_pend).^2.*sin(THE_Phi_pend))./6.0-Lz_pend.^2.*THE_Theta_pend_D.*m_pend.*cos(THE_Psi).*cos(THE_Psi_pend).^2.*cos(THE_Theta_pend).^2.*sin(THE_Phi_pend).*(2.0./3.0)+(Lx_pend.^2.*THE_Phi_pend_D.*m_pend.*cos(THE_Psi).*cos(THE_Phi_pend).*cos(THE_Theta_pend).*sin(THE_Theta_pend))./1.2e+1-(Ly_pend.^2.*THE_Phi_pend_D.*m_pend.*cos(THE_Psi).*cos(THE_Phi_pend).*cos(THE_Theta_pend).*sin(THE_Theta_pend))./1.2e+1+Lz_pend.*THE_Psi_pend_D.*Tv_Z_pend.*m_pend.*cos(THE_Psi).*cos(THE_Phi_pend).*cos(THE_Psi_pend)+(Ly_pend.^2.*THE_Phi_pend_D.*m_pend.*cos(THE_Psi).*cos(THE_Psi_pend).*cos(THE_Theta_pend).*sin(THE_Phi_pend).*sin(THE_Psi_pend))./1.2e+1-(Lz_pend.^2.*THE_Phi_pend_D.*m_pend.*cos(THE_Psi).*cos(THE_Psi_pend).*cos(THE_Theta_pend).*sin(THE_Phi_pend).*sin(THE_Psi_pend))./3.0-(Lz_pend.*THE_Phi_pend_D.*Tv_Z_pend.*m_pend.*cos(THE_Psi).*cos(THE_Phi_pend).*cos(THE_Psi_pend).*sin(THE_Theta_pend))./2.0;
    et341 = -Lz_pend.*THE_Theta_pend_D.*Tv_Z_pend.*m_pend.*cos(THE_Psi).*cos(THE_Psi_pend).*cos(THE_Theta_pend).*sin(THE_Phi_pend)+Lz_pend.*THE_Psi_pend_D.*Tv_Z_pend.*m_pend.*cos(THE_Psi).*sin(THE_Phi_pend).*sin(THE_Psi_pend).*sin(THE_Theta_pend)+(Ly_pend.^2.*THE_Phi_pend_D.*m_pend.*cos(THE_Psi).*cos(THE_Phi_pend).*cos(THE_Psi_pend).^2.*cos(THE_Theta_pend).*sin(THE_Theta_pend))./1.2e+1-(Lz_pend.^2.*THE_Phi_pend_D.*m_pend.*cos(THE_Psi).*cos(THE_Phi_pend).*cos(THE_Psi_pend).^2.*cos(THE_Theta_pend).*sin(THE_Theta_pend))./3.0-(Ly_pend.^2.*THE_Psi_pend_D.*m_pend.*cos(THE_Psi).*cos(THE_Psi_pend).*cos(THE_Theta_pend).*sin(THE_Phi_pend).*sin(THE_Psi_pend).*sin(THE_Theta_pend))./6.0+Lz_pend.^2.*THE_Psi_pend_D.*m_pend.*cos(THE_Psi).*cos(THE_Psi_pend).*cos(THE_Theta_pend).*sin(THE_Phi_pend).*sin(THE_Psi_pend).*sin(THE_Theta_pend).*(2.0./3.0);
    et342 = (Lx_pend.^2.*THE_Theta_pend_D.*m_pend.*cos(THE_Phi_pend).*sin(THE_Theta))./6.0-(Lx_pend.^2.*THE_Theta_pend_D.*m_pend.*cos(THE_Theta).*sin(THE_Psi).*sin(THE_Phi_pend))./6.0+(Ly_pend.^2.*THE_Psi_pend_D.*m_pend.*cos(THE_Theta_pend).*sin(THE_Theta).*sin(THE_Phi_pend))./6.0-(Lx_pend.^2.*THE_Theta_pend_D.*m_pend.*cos(THE_Phi_pend).*cos(THE_Theta_pend).^2.*sin(THE_Theta))./6.0+(Ly_pend.^2.*THE_Theta_pend_D.*m_pend.*cos(THE_Phi_pend).*cos(THE_Theta_pend).^2.*sin(THE_Theta))./6.0+(Lz_pend.*THE_Phi_pend_D.*Tv_Z_pend.*m_pend.*cos(THE_Phi_pend).*sin(THE_Theta).*sin(THE_Psi_pend))./2.0+Lz_pend.*THE_Psi_pend_D.*Tv_Z_pend.*m_pend.*cos(THE_Psi_pend).*sin(THE_Theta).*sin(THE_Phi_pend)+(Lx_pend.^2.*THE_Theta_pend_D.*m_pend.*cos(THE_Theta).*cos(THE_Theta_pend).^2.*sin(THE_Psi).*sin(THE_Phi_pend))./6.0-(Ly_pend.^2.*THE_Theta_pend_D.*m_pend.*cos(THE_Theta).*cos(THE_Theta_pend).^2.*sin(THE_Psi).*sin(THE_Phi_pend))./6.0-(Ly_pend.^2.*THE_Psi_pend_D.*m_pend.*cos(THE_Psi_pend).^2.*cos(THE_Theta_pend).*sin(THE_Theta).*sin(THE_Phi_pend))./6.0+Lz_pend.^2.*THE_Psi_pend_D.*m_pend.*cos(THE_Psi_pend).^2.*cos(THE_Theta_pend).*sin(THE_Theta).*sin(THE_Phi_pend).*(2.0./3.0);
    et343 = Ly_pend.^2.*THE_Theta_pend_D.*m_pend.*cos(THE_Phi_pend).*cos(THE_Psi_pend).^2.*cos(THE_Theta_pend).^2.*sin(THE_Theta).*(-1.0./6.0)+Lz_pend.^2.*THE_Theta_pend_D.*m_pend.*cos(THE_Phi_pend).*cos(THE_Psi_pend).^2.*cos(THE_Theta_pend).^2.*sin(THE_Theta).*(2.0./3.0)-(Lx_pend.^2.*THE_Theta_pend_D.*m_pend.*cos(THE_Psi).*cos(THE_Theta).*cos(THE_Theta_pend).*sin(THE_Theta_pend))./6.0+(Ly_pend.^2.*THE_Psi_pend_D.*m_pend.*cos(THE_Theta).*cos(THE_Phi_pend).*cos(THE_Theta_pend).*sin(THE_Psi))./6.0+(Ly_pend.^2.*THE_Theta_pend_D.*m_pend.*cos(THE_Psi).*cos(THE_Theta).*cos(THE_Theta_pend).*sin(THE_Theta_pend))./6.0+(Lx_pend.^2.*THE_Phi_pend_D.*m_pend.*cos(THE_Theta_pend).*sin(THE_Theta).*sin(THE_Phi_pend).*sin(THE_Theta_pend))./1.2e+1-(Ly_pend.^2.*THE_Phi_pend_D.*m_pend.*cos(THE_Theta_pend).*sin(THE_Theta).*sin(THE_Phi_pend).*sin(THE_Theta_pend))./1.2e+1+(Ly_pend.^2.*THE_Theta_pend_D.*m_pend.*cos(THE_Theta).*cos(THE_Psi_pend).^2.*cos(THE_Theta_pend).^2.*sin(THE_Psi).*sin(THE_Phi_pend))./6.0-Lz_pend.^2.*THE_Theta_pend_D.*m_pend.*cos(THE_Theta).*cos(THE_Psi_pend).^2.*cos(THE_Theta_pend).^2.*sin(THE_Psi).*sin(THE_Phi_pend).*(2.0./3.0)+(Lx_pend.^2.*THE_Phi_pend_D.*m_pend.*cos(THE_Theta).*cos(THE_Phi_pend).*cos(THE_Theta_pend).*sin(THE_Psi).*sin(THE_Theta_pend))./1.2e+1;
    et344 = Ly_pend.^2.*THE_Phi_pend_D.*m_pend.*cos(THE_Theta).*cos(THE_Phi_pend).*cos(THE_Theta_pend).*sin(THE_Psi).*sin(THE_Theta_pend).*(-1.0./1.2e+1)-(Ly_pend.^2.*THE_Phi_pend_D.*m_pend.*cos(THE_Phi_pend).*cos(THE_Psi_pend).*cos(THE_Theta_pend).*sin(THE_Theta).*sin(THE_Psi_pend))./1.2e+1+(Lz_pend.^2.*THE_Phi_pend_D.*m_pend.*cos(THE_Phi_pend).*cos(THE_Psi_pend).*cos(THE_Theta_pend).*sin(THE_Theta).*sin(THE_Psi_pend))./3.0+Lz_pend.*THE_Psi_pend_D.*Tv_Z_pend.*m_pend.*cos(THE_Theta).*cos(THE_Phi_pend).*cos(THE_Psi_pend).*sin(THE_Psi)+Lz_pend.*THE_Theta_pend_D.*Tv_Z_pend.*m_pend.*cos(THE_Phi_pend).*cos(THE_Psi_pend).*cos(THE_Theta_pend).*sin(THE_Theta)-(Lz_pend.*THE_Phi_pend_D.*Tv_Z_pend.*m_pend.*cos(THE_Theta).*sin(THE_Psi).*sin(THE_Phi_pend).*sin(THE_Psi_pend))./2.0-(Lz_pend.*THE_Phi_pend_D.*Tv_Z_pend.*m_pend.*cos(THE_Psi_pend).*sin(THE_Theta).*sin(THE_Phi_pend).*sin(THE_Theta_pend))./2.0-Lz_pend.*THE_Psi_pend_D.*Tv_Z_pend.*m_pend.*cos(THE_Phi_pend).*sin(THE_Theta).*sin(THE_Psi_pend).*sin(THE_Theta_pend)-(Ly_pend.^2.*THE_Psi_pend_D.*m_pend.*cos(THE_Theta).*cos(THE_Phi_pend).*cos(THE_Psi_pend).^2.*cos(THE_Theta_pend).*sin(THE_Psi))./6.0-(Ly_pend.^2.*THE_Psi_pend_D.*m_pend.*cos(THE_Psi).*cos(THE_Theta).*cos(THE_Psi_pend).*cos(THE_Theta_pend).^2.*sin(THE_Psi_pend))./6.0;
    et345 = Ly_pend.^2.*THE_Theta_pend_D.*m_pend.*cos(THE_Psi).*cos(THE_Theta).*cos(THE_Psi_pend).^2.*cos(THE_Theta_pend).*sin(THE_Theta_pend).*(-1.0./6.0)+Lz_pend.^2.*THE_Psi_pend_D.*m_pend.*cos(THE_Theta).*cos(THE_Phi_pend).*cos(THE_Psi_pend).^2.*cos(THE_Theta_pend).*sin(THE_Psi).*(2.0./3.0)+Lz_pend.^2.*THE_Psi_pend_D.*m_pend.*cos(THE_Psi).*cos(THE_Theta).*cos(THE_Psi_pend).*cos(THE_Theta_pend).^2.*sin(THE_Psi_pend).*(2.0./3.0)+Lz_pend.^2.*THE_Theta_pend_D.*m_pend.*cos(THE_Psi).*cos(THE_Theta).*cos(THE_Psi_pend).^2.*cos(THE_Theta_pend).*sin(THE_Theta_pend).*(2.0./3.0)+(Ly_pend.^2.*THE_Phi_pend_D.*m_pend.*cos(THE_Psi_pend).^2.*cos(THE_Theta_pend).*sin(THE_Theta).*sin(THE_Phi_pend).*sin(THE_Theta_pend))./1.2e+1-(Lz_pend.^2.*THE_Phi_pend_D.*m_pend.*cos(THE_Psi_pend).^2.*cos(THE_Theta_pend).*sin(THE_Theta).*sin(THE_Phi_pend).*sin(THE_Theta_pend))./3.0+(Ly_pend.^2.*THE_Phi_pend_D.*m_pend.*cos(THE_Theta).*cos(THE_Psi_pend).*cos(THE_Theta_pend).*sin(THE_Psi).*sin(THE_Phi_pend).*sin(THE_Psi_pend))./1.2e+1+(Ly_pend.^2.*THE_Psi_pend_D.*m_pend.*cos(THE_Phi_pend).*cos(THE_Psi_pend).*cos(THE_Theta_pend).*sin(THE_Theta).*sin(THE_Psi_pend).*sin(THE_Theta_pend))./6.0-(Lz_pend.^2.*THE_Phi_pend_D.*m_pend.*cos(THE_Theta).*cos(THE_Psi_pend).*cos(THE_Theta_pend).*sin(THE_Psi).*sin(THE_Phi_pend).*sin(THE_Psi_pend))./3.0;
    et346 = Lz_pend.^2.*THE_Psi_pend_D.*m_pend.*cos(THE_Phi_pend).*cos(THE_Psi_pend).*cos(THE_Theta_pend).*sin(THE_Theta).*sin(THE_Psi_pend).*sin(THE_Theta_pend).*(-2.0./3.0)-(Lz_pend.*THE_Phi_pend_D.*Tv_Z_pend.*m_pend.*cos(THE_Theta).*cos(THE_Phi_pend).*cos(THE_Psi_pend).*sin(THE_Psi).*sin(THE_Theta_pend))./2.0-Lz_pend.*THE_Theta_pend_D.*Tv_Z_pend.*m_pend.*cos(THE_Theta).*cos(THE_Psi_pend).*cos(THE_Theta_pend).*sin(THE_Psi).*sin(THE_Phi_pend)+Lz_pend.*THE_Psi_pend_D.*Tv_Z_pend.*m_pend.*cos(THE_Theta).*sin(THE_Psi).*sin(THE_Phi_pend).*sin(THE_Psi_pend).*sin(THE_Theta_pend)+(Ly_pend.^2.*THE_Phi_pend_D.*m_pend.*cos(THE_Theta).*cos(THE_Phi_pend).*cos(THE_Psi_pend).^2.*cos(THE_Theta_pend).*sin(THE_Psi).*sin(THE_Theta_pend))./1.2e+1-(Lz_pend.^2.*THE_Phi_pend_D.*m_pend.*cos(THE_Theta).*cos(THE_Phi_pend).*cos(THE_Psi_pend).^2.*cos(THE_Theta_pend).*sin(THE_Psi).*sin(THE_Theta_pend))./3.0-(Ly_pend.^2.*THE_Psi_pend_D.*m_pend.*cos(THE_Theta).*cos(THE_Psi_pend).*cos(THE_Theta_pend).*sin(THE_Psi).*sin(THE_Phi_pend).*sin(THE_Psi_pend).*sin(THE_Theta_pend))./6.0+Lz_pend.^2.*THE_Psi_pend_D.*m_pend.*cos(THE_Theta).*cos(THE_Psi_pend).*cos(THE_Theta_pend).*sin(THE_Psi).*sin(THE_Phi_pend).*sin(THE_Psi_pend).*sin(THE_Theta_pend).*(2.0./3.0);
    et347 = Lz_pend.^2.*THE_Psi_pend_D.*m_pend.*cos(THE_Theta_pend).*sin(THE_Psi).*(2.0./3.0)-Lz_pend.^2.*THE_Psi_pend_D.*m_pend.*cos(THE_Psi).*sin(THE_Phi_pend).*sin(THE_Theta_pend).*(2.0./3.0)+(Ly_pend.^2.*THE_Psi_pend_D.*m_pend.*cos(THE_Psi_pend).^2.*cos(THE_Theta_pend).*sin(THE_Psi))./6.0-Lz_pend.^2.*THE_Psi_pend_D.*m_pend.*cos(THE_Psi_pend).^2.*cos(THE_Theta_pend).*sin(THE_Psi).*(2.0./3.0)-(Ly_pend.^2.*THE_Psi_pend_D.*m_pend.*cos(THE_Psi).*cos(THE_Psi_pend).^2.*sin(THE_Phi_pend).*sin(THE_Theta_pend))./6.0+Lz_pend.^2.*THE_Psi_pend_D.*m_pend.*cos(THE_Psi).*cos(THE_Psi_pend).^2.*sin(THE_Phi_pend).*sin(THE_Theta_pend).*(2.0./3.0)+(Ly_pend.^2.*THE_Psi_pend_D.*m_pend.*cos(THE_Psi).*cos(THE_Phi_pend).*cos(THE_Psi_pend).*sin(THE_Psi_pend))./6.0-Lz_pend.^2.*THE_Psi_pend_D.*m_pend.*cos(THE_Psi).*cos(THE_Phi_pend).*cos(THE_Psi_pend).*sin(THE_Psi_pend).*(2.0./3.0)-(Ly_pend.^2.*THE_Theta_pend_D.*m_pend.*cos(THE_Psi_pend).*sin(THE_Psi).*sin(THE_Psi_pend).*sin(THE_Theta_pend))./1.2e+1+(Lz_pend.^2.*THE_Theta_pend_D.*m_pend.*cos(THE_Psi_pend).*sin(THE_Psi).*sin(THE_Psi_pend).*sin(THE_Theta_pend))./3.0-(Ly_pend.^2.*THE_Theta_pend_D.*m_pend.*cos(THE_Psi).*cos(THE_Psi_pend).*cos(THE_Theta_pend).*sin(THE_Phi_pend).*sin(THE_Psi_pend))./1.2e+1;
    et348 = (Lz_pend.^2.*THE_Theta_pend_D.*m_pend.*cos(THE_Psi).*cos(THE_Psi_pend).*cos(THE_Theta_pend).*sin(THE_Phi_pend).*sin(THE_Psi_pend))./3.0-Lz_pend.*THE_Psi_pend_D.*Tv_Z_pend.*m_pend.*cos(THE_Psi).*cos(THE_Phi_pend).*cos(THE_Theta_pend).*sin(THE_Psi_pend)-(Lz_pend.*THE_Theta_pend_D.*Tv_Z_pend.*m_pend.*cos(THE_Psi).*cos(THE_Phi_pend).*cos(THE_Psi_pend).*sin(THE_Theta_pend))./2.0;
    et349 = Lz_pend.^2.*THE_Psi_pend_D.*m_pend.*cos(THE_Phi_pend).*sin(THE_Theta).*sin(THE_Theta_pend).*(2.0./3.0)-Lz_pend.^2.*THE_Psi_pend_D.*m_pend.*cos(THE_Psi).*cos(THE_Theta).*cos(THE_Theta_pend).*(2.0./3.0)-(Ly_pend.^2.*THE_Psi_pend_D.*m_pend.*cos(THE_Psi).*cos(THE_Theta).*cos(THE_Psi_pend).^2.*cos(THE_Theta_pend))./6.0+Lz_pend.^2.*THE_Psi_pend_D.*m_pend.*cos(THE_Psi).*cos(THE_Theta).*cos(THE_Psi_pend).^2.*cos(THE_Theta_pend).*(2.0./3.0)+(Ly_pend.^2.*THE_Psi_pend_D.*m_pend.*cos(THE_Phi_pend).*cos(THE_Psi_pend).^2.*sin(THE_Theta).*sin(THE_Theta_pend))./6.0-Lz_pend.^2.*THE_Psi_pend_D.*m_pend.*cos(THE_Phi_pend).*cos(THE_Psi_pend).^2.*sin(THE_Theta).*sin(THE_Theta_pend).*(2.0./3.0)+(Ly_pend.^2.*THE_Psi_pend_D.*m_pend.*cos(THE_Psi_pend).*sin(THE_Theta).*sin(THE_Phi_pend).*sin(THE_Psi_pend))./6.0-Lz_pend.^2.*THE_Psi_pend_D.*m_pend.*cos(THE_Theta).*sin(THE_Psi).*sin(THE_Phi_pend).*sin(THE_Theta_pend).*(2.0./3.0)-Lz_pend.^2.*THE_Psi_pend_D.*m_pend.*cos(THE_Psi_pend).*sin(THE_Theta).*sin(THE_Phi_pend).*sin(THE_Psi_pend).*(2.0./3.0)+(Ly_pend.^2.*THE_Psi_pend_D.*m_pend.*cos(THE_Theta).*cos(THE_Phi_pend).*cos(THE_Psi_pend).*sin(THE_Psi).*sin(THE_Psi_pend))./6.0;
    et350 = (Ly_pend.^2.*THE_Theta_pend_D.*m_pend.*cos(THE_Psi).*cos(THE_Theta).*cos(THE_Psi_pend).*sin(THE_Psi_pend).*sin(THE_Theta_pend))./1.2e+1+(Ly_pend.^2.*THE_Theta_pend_D.*m_pend.*cos(THE_Phi_pend).*cos(THE_Psi_pend).*cos(THE_Theta_pend).*sin(THE_Theta).*sin(THE_Psi_pend))./1.2e+1-Lz_pend.^2.*THE_Psi_pend_D.*m_pend.*cos(THE_Theta).*cos(THE_Phi_pend).*cos(THE_Psi_pend).*sin(THE_Psi).*sin(THE_Psi_pend).*(2.0./3.0)-(Lz_pend.^2.*THE_Theta_pend_D.*m_pend.*cos(THE_Psi).*cos(THE_Theta).*cos(THE_Psi_pend).*sin(THE_Psi_pend).*sin(THE_Theta_pend))./3.0-(Lz_pend.^2.*THE_Theta_pend_D.*m_pend.*cos(THE_Phi_pend).*cos(THE_Psi_pend).*cos(THE_Theta_pend).*sin(THE_Theta).*sin(THE_Psi_pend))./3.0-Lz_pend.*THE_Psi_pend_D.*Tv_Z_pend.*m_pend.*cos(THE_Theta_pend).*sin(THE_Theta).*sin(THE_Phi_pend).*sin(THE_Psi_pend)-(Lz_pend.*THE_Theta_pend_D.*Tv_Z_pend.*m_pend.*cos(THE_Psi_pend).*sin(THE_Theta).*sin(THE_Phi_pend).*sin(THE_Theta_pend))./2.0-(Ly_pend.^2.*THE_Psi_pend_D.*m_pend.*cos(THE_Theta).*cos(THE_Psi_pend).^2.*sin(THE_Psi).*sin(THE_Phi_pend).*sin(THE_Theta_pend))./6.0+Lz_pend.^2.*THE_Psi_pend_D.*m_pend.*cos(THE_Theta).*cos(THE_Psi_pend).^2.*sin(THE_Psi).*sin(THE_Phi_pend).*sin(THE_Theta_pend).*(2.0./3.0)-(Ly_pend.^2.*THE_Theta_pend_D.*m_pend.*cos(THE_Theta).*cos(THE_Psi_pend).*cos(THE_Theta_pend).*sin(THE_Psi).*sin(THE_Phi_pend).*sin(THE_Psi_pend))./1.2e+1;
    et351 = (Lz_pend.^2.*THE_Theta_pend_D.*m_pend.*cos(THE_Theta).*cos(THE_Psi_pend).*cos(THE_Theta_pend).*sin(THE_Psi).*sin(THE_Phi_pend).*sin(THE_Psi_pend))./3.0-Lz_pend.*THE_Psi_pend_D.*Tv_Z_pend.*m_pend.*cos(THE_Theta).*cos(THE_Phi_pend).*cos(THE_Theta_pend).*sin(THE_Psi).*sin(THE_Psi_pend)-(Lz_pend.*THE_Theta_pend_D.*Tv_Z_pend.*m_pend.*cos(THE_Theta).*cos(THE_Phi_pend).*cos(THE_Psi_pend).*sin(THE_Psi).*sin(THE_Theta_pend))./2.0;
